simulink model "Computer"  (R2023a)
settings: Solver=VariableStepDiscrete  StartTime=0.0  StopTime=inf  RelTol=1e-3  EnableMultiTasking=on
values from neighbouring files (symbols this model uses):
  RomCode = Preprocessor(RomCode, c)    [ROM.m]
undefined symbols (not defined in the file or in its folder): c, in, RomCodeBreakpoints, RomData, RomDataBreakpoints, UartDataRx, UartDataRx_Active
libraries: Miscellaneous x281, simulink_extras x66, Memory_Blocks_Lib x46, simulink x42, Word_Multiplexers_Lib x31, Decoders_Lib x30, Encoders_Lib x10, Counters_Lib x9, Bit_Multiplexers_Lib x8, Arithmetic_Operations_Lib x5, Bit_Demultiplexers_Lib x4, Garbage x1
(part 1 of 6)
settings Model: NumberOfSteps=16  SnapshotInterval=1  PacingRate=8  Creator=Jozko Mrkvicka  LastModifiedBy=Jozko Mrkvicka
settings SolverCC: AlgebraicLoopSolver=TrustRegion
settings DataIOCC: ReturnWorkspaceOutputs=off
settings OptimizationCC: LifeSpan=inf
settings DebuggingCC: UnconnectedInputMsg=warning  UnconnectedOutputMsg=warning  UnconnectedLineMsg=warning  SFUnexpectedBacktrackingDiag=warning  SFNoUnconditionalDefaultTransitionDiag=warning  ArithmeticOperatorsInVariantConditions=warning
settings ModelReferenceCC: EnableRefExpFcnMdlSchedulingChecks=on
settings SFSimCC: SimUseLocalCustomCode=off  CustomCodeUndefinedFunction=UseInterfaceOnly
settings RTWCC: RTWUseLocalCustomCode=off
settings CodeAppCC: StateflowObjectComments=on
settings GRTTargetCC: TargetLangStandard=C89/C90 (ANSI)
settings ConfigComp: CovMetricSettings=dw  CovSaveCumulativeToWorkspaceVar=on  CovSaveSingleToWorkspaceVar=on  CovExternalEMLEnable=off
settings SimscapeCC: SimscapeNormalizeSystem=off

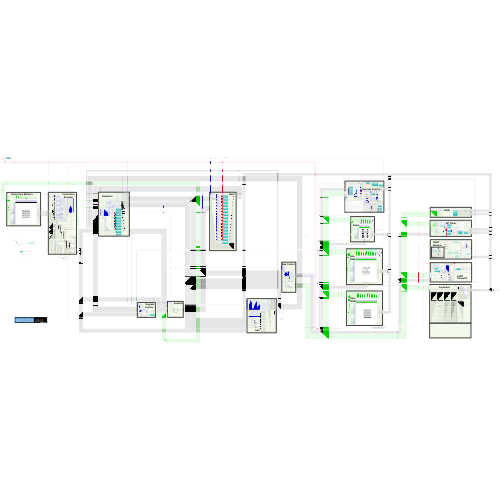
[thumbnail: Simulink's stored preview of the top-level diagram]
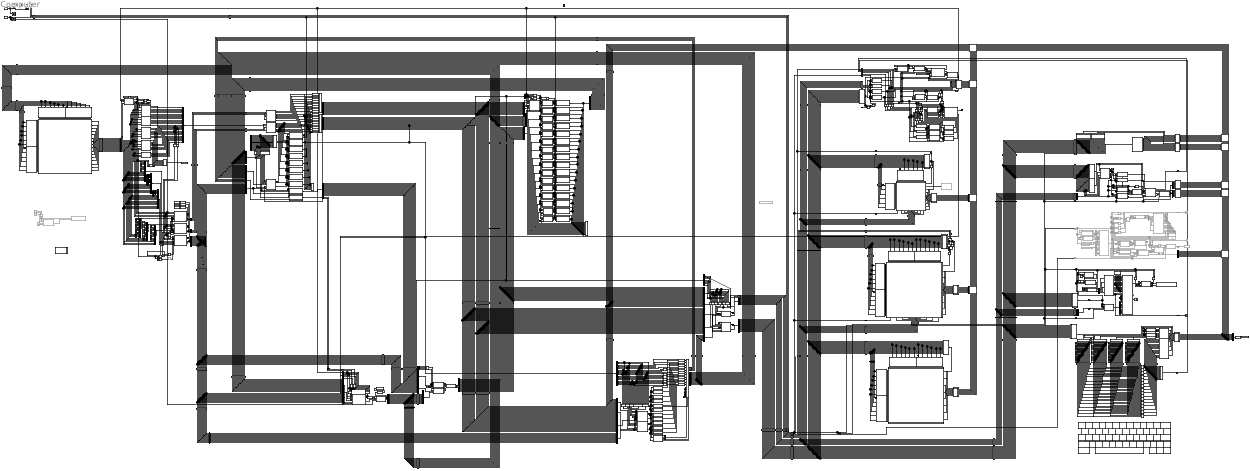
== system Computer ==
  note: TODO: Prerobit Interrupt control tak aby posielal adresu najprv dolu do zmuxovanych zbernic, a az z nich si ju bude program counter brat. Teraz je to spojene priamo.
  note: TODO: Nestacil by tu iba jeden delay blok pre celu zbernicu?
  note: TODO: Tento selector mozno nie je potrebny. Enablovat/disablovat output by sa mozno dalo pomocou signalov Enable(1b) v dekoderoch. Tam je vsak problem v tom, ze ked je enkoder disablovany, tak su vsetky jeho vystupy nulove. Potom pri konverzii nuly na index pola (uz priamo v subsysteme pamati) by mohlo dojst k problemu s matlabovskym polom. Tato poznamka plati pre vsetky vystupne selektory (Video, RAM, ROM).
  note: Note:
      | On physical layer, data read from the ferrite core memory will be immediately written back to that memory.
  note: janko halu š ka inside
  note: Interrupt Control
  note: Interrupt Control
  note: Interrupt Control
      |
      | Enabling/disabling of IRQs is controlled by IRQ Enable Register (memory mapped, read/write).
      | Each bit in the register controls specific IRQ (enable = 1, disable = 0).
      | The following interrupts are implemented in the system:
      | - (Bit 3) Keyboard IRQ
      | - (Bit 2) General Purpose Timer
      |
      | IRQs have different priorities, the higher is bit which enables an IRQ the higher priority that interrupt has.
      | Enabled IRQs are latched when they are activated by some system event (the keyboard IRQ is only exception, it is not latched at all).
      |
      | IRQ is handled in the following way:
      | - Execution of all instructions is blocked for one clock cycle.
      | - Actual Program Counter value (address of active instruction) is pushed to stack.
      | - Program Counter is loaded with an IRQ handler address of the active IRQ. The handler address is stored in the IRQ Vector Table and it can`t be reconfigured by user.
      | - Program execution jumps to the IRQ handler. Information about an IRQ handler being active is latched.
      | - When the IRQ handler is active, it can`t be interrupted by other IRQs, they are temporarily disabled, order of IRQ handling depends on their priorities).
      | - Code of the IRQ handler is executed.
      | - Once the IRQ is handled, it is deactivated. Instruction RET at the end of the handler also resets the handler latch. Now all other IRQs are re-enabled.
      | - Program execution jumps back to the address from which it was interrupted and it normally continues with next instruction.
  note: TODO: Ja si myslim ze format 0 by mal pouzivat iba unsigned immediate. Teraz pouziva signed (imm formatu 0 sa vzdy pouziva ako adresa a adresa nikdy nemoze byt zaporna).
  note: AuxALU
  note: Keyboard_IBM437
  note: Instruction Memory
  note: Video
  note: Data
      | ROM
  note: CYAN COLOR means that block contains sequential logic.
      | BLUE COLOR means that line represents control signal.
      | GREEN COLOR means that line represents address.
  note: Instruction Memory
  note: Stack
  note: Keyboard
  note: Keyboard
  note: Instruction_Decoder
  note: Instruction
      | Decoder
  note: ALU
  note: ALU
  note: Registers
  note: General_Purpose_Registers
  note: General_Purpose_Timer_16bit
  note: CMD_SET_STOP_VALUE
      | - Address 0x0000
      | - Data   <0x0000..0xFFFF>
      |
      | CMD_SET_START_VALUE
      | - Address 0x0001
      | - Data   <0x0000..0xFFFF>
      |
      | CMD_RESET
      | - Address 0x0002
      | - Data    N/A
      |
      | CMD_MODE
      | - Address 0x0003
      | - Data    0x0000 (One Shot)
      |           0x0001 (Free Run)
      |
      | CMD_RUN
      | - Address 0x0004
      | - Data    0x0000 (Halt)
      |           0x0001 (Run)
  note: 9000
  note: MRKVIČKA
  note: Stack
  note: UART
      | Transmitter
  note: UART Transmitter
  note: StartFcn*
      | disp('Starting UART...')
      | evalin('base', 'hSerialPort = serialport(in.UART_COM_PORT, in.UART_BAUD_RATE);');
      | evalin('base', 'configureCallback(hSerialPort, "byte", 1, @SerialPortCallback);');
  note: UART_Receiver
  note: This block is just a workaround (connector) between
      | the Simulink model of the UART digital hardware
      | and Windows virtual terminal. In real-world
      | implementation, this block will not be needed.
  note: StopFcn*
      | disp('Stopping UART...')
      | evalin('base', 'delete(hSerialPort);');
  note: This block is just a workaround (connector) between
      |                      the Simulink model of the UART digital hardware
      |                      and Windows virtual terminal. In real-world implementation,
      |                      this block will not be needed.
  note: UART
      | Receiver
  note: Data ROM
  note: Data
      | RAM
  note: Data RAM
  note: Video
  note: GP Timer
  note: Random_Number_Generator
  note: RNG
  note: Program Counter
  note: Program Counter
  note: Bus Control
  note: Bus Control
  "  Halt" : Constant  Value=0  OutDataTypeStr=boolean
  "  Idle" : Constant  Commented=on  OutDataTypeStr=boolean
  "  Reset" : Constant  Value=0  OutDataTypeStr=boolean
  "  Run" : Constant  OutDataTypeStr=boolean
  " Halt" : Constant  Value=0  OutDataTypeStr=boolean
   Halt{1,5..7,10} (5 alike) : Constant  Commented=on  Value=0  OutDataTypeStr=boolean
  " Halt2" : Constant  Commented=on  Value=0  OutDataTypeStr=uint16
  " Halt3" : Constant  Commented=on  Value=0  OutDataTypeStr=uint16
  " Halt4" : Constant  Value=0  OutDataTypeStr=boolean
  " Halt8" : Constant  Commented=on  Value=0  OutDataTypeStr=uint16
  " Halt9" : Constant  Value=0  OutDataTypeStr=uint16
  " Idle" : Constant  OutDataTypeStr=boolean
  " Reset" : Constant  Value=0  OutDataTypeStr=boolean
  " Run" : Constant  OutDataTypeStr=boolean
  " Run1" : Constant  Commented=on  OutDataTypeStr=boolean
  " Set" : Constant  OutDataTypeStr=boolean
  " StartBit" : Constant  Value=0  OutDataTypeStr=boolean
  " StopBit" : Constant  OutDataTypeStr=boolean
  !1 : Constant  Value=0  OutDataTypeStr=boolean
  "\"/?\"" : Constant  Value=0  OutDataTypeStr=boolean
  "\"2" : Constant  Value=0  OutDataTypeStr=boolean
  #3 : Constant  Value=0  OutDataTypeStr=boolean
  $4 : Constant  Value=0  OutDataTypeStr=boolean
  %5 : Constant  Value=0  OutDataTypeStr=boolean
  &6 : Constant  Value=0  OutDataTypeStr=boolean
  '7 : Constant  Value=0  OutDataTypeStr=boolean
  (8 : Constant  Value=0  OutDataTypeStr=boolean
  (UartRxPin) : Constant  Commented=on  Value=UartDataRx  OutDataTypeStr=uint8
  )9 : Constant  Value=0  OutDataTypeStr=boolean
  *: : Constant  Value=0  OutDataTypeStr=boolean
  +; : Constant  Value=0  OutDataTypeStr=boolean
  ,< : Constant  Value=0  OutDataTypeStr=boolean
  -= : Constant  Value=0  OutDataTypeStr=boolean
  .> : Constant  Value=0  OutDataTypeStr=boolean
  <0x0000..0x0FFF> : Subsystem
  <0x1000..0x1FFF> : Subsystem
  <0x2000..0x23FF> : Subsystem
  <0xFFF6..0xFFF6> : Subsystem
  <0xFFF7..0xFFF7> : Subsystem
  <0xFFF8..0xFFFD> : Subsystem
  <0xFFF8..0xFFFD>1 : Subsystem
  <0xFFFE..0xFFFE> : Subsystem
  <0xFFFF..0xFFFF> : Subsystem
  <0xFFFF..0xFFFF>1 : Subsystem
  @` : Constant  Value=0  OutDataTypeStr=boolean
  ADD ADDI MOVU SHIFT : Logic  Operator=OR  Inputs=13  IconShape=distinctive  AllPortsSameDT=off  OutDataTypeStr=boolean
  ADD_or_ADDI : Constant  Commented=on  Value=0  OutDataTypeStr=boolean
  Aa : Constant  Value=0  OutDataTypeStr=boolean
  Align{1,5,7..14,16..20,22..23,31,33,38,42,44..45,58..59,78..80,86..90,93,99..101} (37 alike) : Miscellaneous/Align16  SystemSampleTime=-1  VariantActivationTime=update diagram  Latency=0  AutoFrameSizeCalculation=off
  Align15 : Miscellaneous/Align6
  Align2 : Miscellaneous/Align6
  Align{21,24..30,34..37,39..41,43,81,92,95} (19 alike) : Miscellaneous/Align8  SystemSampleTime=-1  VariantActivationTime=update diagram  Latency=0  AutoFrameSizeCalculation=off
  Align{3..4,60..70,72..73,85,97..98} (18 alike) : Miscellaneous/Align12  SystemSampleTime=-1  VariantActivationTime=update diagram  Latency=0  AutoFrameSizeCalculation=off
  Align32 : Miscellaneous/Align5
  Align{46..51,54..57,82..84} (13 alike) : Miscellaneous/Align3  SystemSampleTime=-1  VariantActivationTime=update diagram  Latency=0  AutoFrameSizeCalculation=off
  Align{52..53,71,91} (4 alike) : Miscellaneous/Align2  SystemSampleTime=-1  VariantActivationTime=update diagram  Latency=0  AutoFrameSizeCalculation=off
  Align6 : Miscellaneous/Align6
  Align{74..77} (4 alike) : Miscellaneous/Align4  SystemSampleTime=-1  VariantActivationTime=update diagram  Latency=0  AutoFrameSizeCalculation=off
  Alignment{,1..8,10,13..15,17,23..26,28..30,34..36} (24 alike) : Miscellaneous/Alignment  SystemSampleTime=-1  VariantActivationTime=update diagram  Latency=0  AutoFrameSizeCalculation=off
  Alignment11 : Miscellaneous/Alignment  Commented=on  SystemSampleTime=-1  VariantActivationTime=update diagram  Latency=0  AutoFrameSizeCalculation=off
  Alignment12 : Miscellaneous/Alignment  Commented=on  SystemSampleTime=-1  VariantActivationTime=update diagram  Latency=0  AutoFrameSizeCalculation=off
  Alignment9 : Miscellaneous/Alignment  Commented=on  SystemSampleTime=-1  VariantActivationTime=update diagram  Latency=0  AutoFrameSizeCalculation=off
  AuxALU : Arithmetic_Operations_Lib/Word_Adder  SystemSampleTime=-1  VariantActivationTime=update diagram  Latency=0  AutoFrameSizeCalculation=off
      settings: LibrarySourceBlock=Arithmetic_Operations_Lib/Arithmetic_Operations_Lib/Word_Adder
  BaudRate : Scope
  Bb : Constant  Value=0  OutDataTypeStr=boolean
  Bit to Integer Converter{4..8,15} (6 alike) : simulink/Logic and Bit Operations/Bit to Integer Converter  nbits=16  bitOrder=MSB first  signedOutputValues=Unsigned  outDtype=uint16  outDtypeSigned=Inherit via internal rule
      settings: LibrarySourceBlock=|
      | commutil2/Bit to Integer
      | Converter
  Bit_Demux_{1..4} (4 alike) : Bit_Demultiplexers_Lib/Bit_Demux_2  SystemSampleTime=-1  VariantActivationTime=update diagram  Latency=0  AutoFrameSizeCalculation=off
      settings: LibrarySourceBlock=Garbage/Bit_Demux_2
  Bit_Mux_{1..4} (4 alike) : Bit_Multiplexers_Lib/Bit_Mux_2  SystemSampleTime=-1  VariantActivationTime=update diagram  Latency=0  AutoFrameSizeCalculation=off
  Bit_Mux_16 : Bit_Multiplexers_Lib/Bit_Mux_16  SystemSampleTime=-1  VariantActivationTime=update diagram  Latency=0  AutoFrameSizeCalculation=off
  Bit_Mux_16_Nand : Garbage/Bit_Mux_16_Nand  Commented=on  SystemSampleTime=-1  VariantActivationTime=update diagram  Latency=0  AutoFrameSizeCalculation=off
  Bit_Mux_2(1) : Bit_Multiplexers_Lib/Bit_Mux_2  SystemSampleTime=-1  VariantActivationTime=update diagram  Latency=0  AutoFrameSizeCalculation=off
  Bit_Mux_2(1)1 : Bit_Multiplexers_Lib/Bit_Mux_2  Commented=on  SystemSampleTime=-1  VariantActivationTime=update diagram  Latency=0  AutoFrameSizeCalculation=off
  Bit_Mux_2(1)2 : Bit_Multiplexers_Lib/Bit_Mux_2  SystemSampleTime=-1  VariantActivationTime=update diagram  Latency=0  AutoFrameSizeCalculation=off
  Block keyboard interrupt when the interrupt delay counter is running : Logic  Operator=NOT  IconShape=distinctive  AllPortsSameDT=off  OutDataTypeStr=boolean
  Bus Creator{1,4..9,11..14,21..26,29..30} (19 alike) : BusCreator  Inputs=16
  Bus Creator{2,10,20,27..28} (5 alike) : BusCreator  Inputs=8
  Bus Creator{15..18} (4 alike) : BusCreator  Inputs=12
  Bus Creator19 : BusCreator  Inputs=4
  Bus Creator3 : BusCreator  Inputs=29
  Bus Selector : BusSelector  OutputSignals=LDL,XOR,LDLI,OR,AND,ADD,ADDI,MOVU,SHIFTI,LDUI,LDU,NOT,SHIFT,MOVL,POP,MOV,SGMT,CMP,CMPI
  Bus Selector{1,9..10,13,18,26,28} (7 alike) : BusSelector  OutputSignals=b15,b14,b13,b12,b11,b10,b09,b08,b07,b06,b05,b04,b03,b02,b01,b00
  Bus Selector11 : BusSelector  OutputSignals=b11,b10,b09,b08,b07,b06,b05,b04,b03,b02,b01,b00
  Bus Selector15 : BusSelector  OutputSignals=b00
  Bus Selector16 : BusSelector  OutputSignals=b15,b14,b13,b12,b11,b10,b09,b08
  Bus Selector17 : BusSelector  OutputSignals=Equal,LessThanSigned
  Bus Selector19 : BusSelector  OutputSignals=b00,b01,b02,b03,b04,b05,b06,b07
  Bus Selector2 : BusSelector  OutputSignals=CMPI,CMP,NOT,XOR,OR,AND,ADDI,ADD,MOVU,SHIFT,SHIFTI,STUI,STU,STLI,STL,LDUI,LDU,LDLI,LDL
  Bus Selector20 : BusSelector  Commented=on  OutputSignals=b0,b1,b2,b3,b4,b5,b6,b7
  Bus Selector21 : BusSelector  Commented=on  OutputSignals=b3,b2,b1,b0
  Bus Selector22 : BusSelector  Commented=on  OutputSignals=b01,b00
  Bus Selector23 : BusSelector  OutputSignals=b03,b02,b01,b00
  Bus Selector24 : BusSelector  Commented=on  OutputSignals=b3,b2,b1,b0
  Bus Selector25 : BusSelector  OutputSignals=b07,b06,b05,b04,b03,b02,b01,b00
  Bus Selector27 : BusSelector  OutputSignals=b11,b10,b09,b08,b07,b06,b05,b04,b03,b02,b01,b00
  Bus Selector29 : BusSelector  OutputSignals=b02,b01,b00
  Bus Selector3 : BusSelector  OutputSignals=RET,STUI,STLI,STU,STL,LDUI,LDLI,LDU,LDL
  Bus Selector30 : BusSelector  OutputSignals=b02,b01,b00
  Bus Selector4 : BusSelector  OutputSignals=b07,b06,b05,b04,b03,b02,b01,b00
  Bus Selector5 : BusSelector  OutputSignals=PUSH,CALL,POP,RET
  Bus Selector6 : BusSelector  OutputSignals=b00,b01,b02,b03,b04,b05,b06,b07
  Bus Selector7 : BusSelector  OutputSignals=RET,JMP,CALL,JPE,JLT
  Bus Selector8 : BusSelector  OutputSignals=STUI,STLI,LDUI,LDLI,CALL
  CLK{,3..7} (6 alike) : Miscellaneous/Alignment  SystemSampleTime=-1  VariantActivationTime=update diagram  Latency=0  AutoFrameSizeCalculation=off
  CLK1 : Miscellaneous/Alignment  Commented=on  SystemSampleTime=-1  VariantActivationTime=update diagram  Latency=0  AutoFrameSizeCalculation=off
  CLK2 : Miscellaneous/Alignment  Commented=on  SystemSampleTime=-1  VariantActivationTime=update diagram  Latency=0  AutoFrameSizeCalculation=off
  CMP_or_CMPI : Constant  Commented=on  Value=0  OutDataTypeStr=boolean
  CPU : Scope
  Cc : Constant  Value=0  OutDataTypeStr=boolean
  Clear_RxBufferReady : Constant  Commented=on  OutDataTypeStr=boolean
  Clock : simulink_extras/Flip Flops/Clock  period=16
  Constant{1..2,5,9,11..13,15..16,18,26..44,46..59,61..66,69,72,75,87..90} (56 alike) : Constant  Value=0  OutDataTypeStr=boolean
  Constant{3,6..7,10,19,60,77} (7 alike) : Constant  Value=0  OutDataTypeStr=Bus: BUS_UINT16_T
  Constant45 : Constant  Commented=on  Value=10  OutDataTypeStr=uint8
  Constant67 : Constant  Value=in.IRQ_ADDR_KEYBOARD  OutDataTypeStr=uint16
  Constant68 : Constant  Value=in.IRQ_ADDR_UART  OutDataTypeStr=uint16
  Constant70 : Constant
  Constant71 : Constant  Value=in.IRQ_ADDR_TIMER  OutDataTypeStr=uint16
  Constant73 : Constant  Value=0
  Constant74 : Constant  Value=in.IRQ_ADDR_FPU  OutDataTypeStr=uint16
  Constant76 : Constant  Value=in.IRQ_Keyboard_Test  OutDataTypeStr=uint16
  Constant83 : Constant  Value=15  OutDataTypeStr=uint8
  Constant91 : Constant  Commented=on  Value=0  OutDataTypeStr=boolean
  Constant92 : Constant  Value=10  OutDataTypeStr=uint8
  Constant93 : Constant  Commented=on  Value=UartDataRx_Active  OutDataTypeStr=boolean
  Constant94 : Constant  Commented=on  Value=10  OutDataTypeStr=uint8
  Constant95 : Constant  OutDataTypeStr=boolean
  Constant96 : Constant  OutDataTypeStr=boolean
  Counter_16bit : Counters_Lib/Counter_16bit  SystemSampleTime=-1  VariantActivationTime=update diagram  Latency=0  AutoFrameSizeCalculation=off
  Counter_16bit(1) : Counters_Lib/Counter_16bit  SystemSampleTime=-1  VariantActivationTime=update diagram  Latency=0  AutoFrameSizeCalculation=off
  Counter_Control : Counters_Lib/Counter_Control  SystemSampleTime=-1  VariantActivationTime=update diagram  Latency=0  AutoFrameSizeCalculation=off
  Counter_Control(1) : Counters_Lib/Counter_Control  SystemSampleTime=-1  VariantActivationTime=update diagram  Latency=0  AutoFrameSizeCalculation=off
  CrRet undef : Constant  Value=0  OutDataTypeStr=boolean
  Ctrl01 : Constant  Value=0  OutDataTypeStr=boolean
  Ctrl02 : Constant  Value=0  OutDataTypeStr=boolean
  Ctrl03 : Constant  Value=0  OutDataTypeStr=boolean
  Ctrl04 : Constant  Value=0  OutDataTypeStr=boolean
  Ctrl05 : Constant  Value=0  OutDataTypeStr=boolean
  Ctrl06 : Constant  Value=0  OutDataTypeStr=boolean
  Ctrl07 : Constant  Value=0  OutDataTypeStr=boolean
  Ctrl12 : Constant  Value=0  OutDataTypeStr=boolean
  Ctrl14 : Constant  Value=0  OutDataTypeStr=boolean
  Ctrl15 : Constant  Value=0  OutDataTypeStr=boolean
  DataBitDetected (GoToNextState) : Logic  Commented=on  IconShape=distinctive  AllPortsSameDT=off  OutDataTypeStr=boolean
  Data_RAM (0x000 .. 0xFFF) : Subsystem
      settings: PortSchema="{\"entries\":[{\"content\":{\"sides\":[{\"content\":{\"connectorIds\":[\"In1\",\"In2\",\"In3\",\"In4\",\"In5\",\"In6\",\"In7\",\"In8\",\"In9\",\"In10\",\"In11\",\"In12\",\"In13\",\"In14\",\"In15\",\"In16\",\"In17\",\"In18\",\"In19\",\"In20\",\"In21\",\"In22\",\"In23\",\"In24\",\"In25\",\"In26\",\"In27\",\"In28\",\"In29\",\"In30\",\"In31\",\"In32\",\"In33\",\"In34\",\"In35\",\"In36\",\"In37\",\"In38\",\"In39\",\"In40\",\"In41\",\"In42\",\"In43\",\"In44\",\"In45\",\"In46\",\"In47\",\"In48\",\"In49\",\"In50\",\"In51\",\"In52\",\"In53\",\"In54\",\"In55\",\"In56\",\"In57\",\"In58\",\"In59\",\"In60\",\"In61\",\"In62\",\"In63\",\"In64\"]},\"type\":\"ConnectorPlacement.EquallySpacedRectSide\",\"uuid\":\"1db07b03-14d7-4059-8e9e-27241d1b2c6f\"},{\"content\":{\"connectorIds\":[\"In138\",\"Out1\",\"Out2\",\"Out3\",\"Out4\",\"Out5\",\"Out6\",\"Out7\",\"Out8\"],\"side\":\"RIGHT\"},\"type\":\"ConnectorPlacement.EquallySpacedRectSide\",\"uuid\":\"da5110d5-f105-41ed-a5ea-e540a7740f0d\"},{\"content\":{\"connectorIds\":[\"In65\",\"In66\",\"In67\",\"In68\",\"In69\",\"In70\",\"In71\",\"In72\",\"In73\",\"In74\",\"In75\",\"In76\",\"In77\",\"In78\",\"In79\",\"In80\",\"In81\",\"In82\",\"In83\",\"In84\",\"In85\",\"In86\",\"In87\",\"In88\",\"In89\",\"In90\",\"In91\",\"In92\",\"In93\",\"In94\",\"In95\",\"In96\",\"In97\",\"In98\",\"In99\",\"In100\",\"In101\",\"In102\",\"In103\",\"In104\",\"In105\",\"In106\",\"In107\",\"In108\",\"In109\",\"In110\",\"In111\",\"In112\",\"In113\",\"In114\",\"In115\",\"In116\",\"In117\",\"In118\",\"In119\",\"In120\",\"In121\",\"In122\",\"In123\",\"In124\",\"In125\",\"In126\",\"In127\",\"In128\"],\"side\":\"TOP\"},\"type\":\"ConnectorPlacement.EquallySpacedRectSide\",\"uuid\":\"ecc4e51e-7cb2-40ca-97e4-7326426aa5e7\"},{\"content\":{\"connectorIds\":[\"In129\",\"In130\",\"In131\",\"In132\",\"In133\",\"In134\",\"In135\",\"In136\",\"In137\"],\"side\":\"BOTTOM\"},\"type\":\"ConnectorPlacement.EquallySpacedRectSide\",\"uuid\":\"3d59fc9c-ab69-48a8-998e-8118c8f06a1a\"}]},\"type\":\"ConnectorPlacement.EquallySpacedConnector\",\"uuid\":\"5e28cbe1-b8ac-4836-91bf-5b5dc95013cb\"}],\"packageUris\":[\"http://schema.mathworks.com/mf0/Connector/R2020b\"],\"version\":\"1.0\"}"
  Data_ROM (0x000 .. 0xFFF) : Subsystem
      settings: PortSchema="{\"entries\":[{\"content\":{\"sides\":[{\"content\":{\"connectorIds\":[\"In1\",\"In2\",\"In3\",\"In4\",\"In5\",\"In6\",\"In7\",\"In8\",\"In9\",\"In10\",\"In11\",\"In12\",\"In13\",\"In14\",\"In15\",\"In16\",\"In17\",\"In18\",\"In19\",\"In20\",\"In21\",\"In22\",\"In23\",\"In24\",\"In25\",\"In26\",\"In27\",\"In28\",\"In29\",\"In30\",\"In31\",\"In32\",\"In33\",\"In34\",\"In35\",\"In36\",\"In37\",\"In38\",\"In39\",\"In40\",\"In41\",\"In42\",\"In43\",\"In44\",\"In45\",\"In46\",\"In47\",\"In48\",\"In49\",\"In50\",\"In51\",\"In52\",\"In53\",\"In54\",\"In55\",\"In56\",\"In57\",\"In58\",\"In59\",\"In60\",\"In61\",\"In62\",\"In63\",\"In64\"]},\"type\":\"ConnectorPlacement.EquallySpacedRectSide\",\"uuid\":\"1db07b03-14d7-4059-8e9e-27241d1b2c6f\"},{\"content\":{\"connectorIds\":[\"Out1\",\"Out2\",\"Out3\",\"Out4\",\"Out5\",\"Out6\",\"Out7\",\"Out8\"],\"side\":\"RIGHT\"},\"type\":\"ConnectorPlacement.EquallySpacedRectSide\",\"uuid\":\"da5110d5-f105-41ed-a5ea-e540a7740f0d\"},{\"content\":{\"connectorIds\":[\"In65\",\"In66\",\"In67\",\"In68\",\"In69\",\"In70\",\"In71\",\"In72\",\"In73\",\"In74\",\"In75\",\"In76\",\"In77\",\"In78\",\"In79\",\"In80\",\"In81\",\"In82\",\"In83\",\"In84\",\"In85\",\"In86\",\"In87\",\"In88\",\"In89\",\"In90\",\"In91\",\"In92\",\"In93\",\"In94\",\"In95\",\"In96\",\"In97\",\"In98\",\"In99\",\"In100\",\"In101\",\"In102\",\"In103\",\"In104\",\"In105\",\"In106\",\"In107\",\"In108\",\"In109\",\"In110\",\"In111\",\"In112\",\"In113\",\"In114\",\"In115\",\"In116\",\"In117\",\"In118\",\"In119\",\"In120\",\"In121\",\"In122\",\"In123\",\"In124\",\"In125\",\"In126\",\"In127\",\"In128\"],\"side\":\"TOP\"},\"type\":\"ConnectorPlacement.EquallySpacedRectSide\",\"uuid\":\"ecc4e51e-7cb2-40ca-97e4-7326426aa5e7\"}]},\"type\":\"ConnectorPlacement.EquallySpacedConnector\",\"uuid\":\"5e28cbe1-b8ac-4836-91bf-5b5dc95013cb\"}],\"packageUris\":[\"http://schema.mathworks.com/mf0/Connector/R2020b\"],\"version\":\"1.0\"}"
  Dd : Constant  Value=0  OutDataTypeStr=boolean
  Dec_1 : Decoders_Lib/Dec_8  SystemSampleTime=-1  VariantActivationTime=update diagram  Latency=0  AutoFrameSizeCalculation=off
  Dec_16 : Decoders_Lib/Dec_16  SystemSampleTime=-1  VariantActivationTime=update diagram  Latency=0  AutoFrameSizeCalculation=off
  Dec_32_Enbl{1,4..7,9,11..18} (14 alike) : Decoders_Lib/Dec_32_Enbl  SystemSampleTime=-1  VariantActivationTime=update diagram  Latency=0  AutoFrameSizeCalculation=off
  Dec_4_Enbl : Decoders_Lib/Dec_4_Enbl  SystemSampleTime=-1  VariantActivationTime=update diagram  Latency=0  AutoFrameSizeCalculation=off
  Dec_8 : Decoders_Lib/Dec_8  SystemSampleTime=-1  VariantActivationTime=update diagram  Latency=0  AutoFrameSizeCalculation=off
  Dec_8_Enbl : Decoders_Lib/Dec_8_Enbl  SystemSampleTime=-1  VariantActivationTime=update diagram  Latency=0  AutoFrameSizeCalculation=off
  Delay : Constant  Value=in.IRQ_KEYBOARD_DELAY  OutDataTypeStr=uint16
  Delay_8b : Miscellaneous/Delay_8b  SystemSampleTime=-1  VariantActivationTime=update diagram  Latency=0  AutoFrameSizeCalculation=off
  Delay_8b1 : Miscellaneous/Delay_8b  SystemSampleTime=-1  VariantActivationTime=update diagram  Latency=0  AutoFrameSizeCalculation=off
  Ee : Constant  Value=0  OutDataTypeStr=boolean
  Enable_IRQ_FPU : Memory_Blocks_Lib/Bit_DataEnbl  SystemSampleTime=-1  VariantActivationTime=update diagram  Latency=0  AutoFrameSizeCalculation=off
  Enable_IRQ_Keyboard : Memory_Blocks_Lib/Bit_DataEnbl  SystemSampleTime=-1  VariantActivationTime=update diagram  Latency=0  AutoFrameSizeCalculation=off
  Enable_IRQ_Timer : Memory_Blocks_Lib/Bit_DataEnbl  SystemSampleTime=-1  VariantActivationTime=update diagram  Latency=0  AutoFrameSizeCalculation=off
  Enable_IRQ_UART : Memory_Blocks_Lib/Bit_DataEnbl  SystemSampleTime=-1  VariantActivationTime=update diagram  Latency=0  AutoFrameSizeCalculation=off
  Enc_16 : Encoders_Lib/Enc_16  SystemSampleTime=-1  VariantActivationTime=update diagram  Latency=0  AutoFrameSizeCalculation=off
  Enc_2 : Encoders_Lib/Enc_8  SystemSampleTime=-1  VariantActivationTime=update diagram  Latency=0  AutoFrameSizeCalculation=off
  Entering_IRQ_Handler... (1 clock cycle) : Logic  Operator=NOT  IconShape=distinctive  AllPortsSameDT=off  OutDataTypeStr=boolean
  ErrorStopBitNotDetected : Terminator  Commented=on
  "Exiting_IRQ_Handler... (1 clock cycle) " : Logic  IconShape=distinctive  AllPortsSameDT=off  OutDataTypeStr=boolean
  Ff : Constant  Value=0  OutDataTypeStr=boolean
  "For simulation, use only data bits. Real-world implementation will use whole frame." : Logic  Operator=OR  Inputs=8  IconShape=distinctive  AllPortsSameDT=off  OutDataTypeStr=boolean
  Format 0: FF|OO|CCCC   CCCCCCCC : Decoders_Lib/Dec_4_Enbl  SystemSampleTime=-1  VariantActivationTime=update diagram  Latency=0  AutoFrameSizeCalculation=off
  Format 1: FF|OOO|SSS   CCCCCCCC : Decoders_Lib/Dec_8_Enbl  SystemSampleTime=-1  VariantActivationTime=update diagram  Latency=0  AutoFrameSizeCalculation=off
  Format 2: FF|OOO|DDD   CCCCCCCC : Decoders_Lib/Dec_8_Enbl  SystemSampleTime=-1  VariantActivationTime=update diagram  Latency=0  AutoFrameSizeCalculation=off
  Format 3: FF|OOOOO|R   R|DDD|R|SSS : Decoders_Lib/Dec_8_Enbl  SystemSampleTime=-1  VariantActivationTime=update diagram  Latency=0  AutoFrameSizeCalculation=off
  Format 3: FF|OOOOO|R   R|DDD|R|SSS2 : Decoders_Lib/Dec_8_Enbl  SystemSampleTime=-1  VariantActivationTime=update diagram  Latency=0  AutoFrameSizeCalculation=off
  Format_1_Signed : Logic  IconShape=distinctive  AllPortsSameDT=off  OutDataTypeStr=boolean
  Format_1_Unsigned : Logic  IconShape=distinctive  AllPortsSameDT=off  OutDataTypeStr=boolean
  Format_2_Signed : Logic  IconShape=distinctive  AllPortsSameDT=off  OutDataTypeStr=boolean
  Format_2_Unsigned : Logic  IconShape=distinctive  AllPortsSameDT=off  OutDataTypeStr=boolean
  FreqDivider : Counters_Lib/Counter_4bit_Cfg  SystemSampleTime=-1  VariantActivationTime=update diagram  Latency=0  AutoFrameSizeCalculation=off
  FromImmediate : Constant  Commented=on  Value=0  OutDataTypeStr=boolean
  General_Purpose_Register_{0..7} (8 alike) : Memory_Blocks_Lib/Word  SystemSampleTime=-1  VariantActivationTime=update diagram  Latency=0  AutoFrameSizeCalculation=off
      settings: LibrarySourceBlock=Memory_Blocks_Lib/Memory_Blocks_Lib/Word
  Gg : Constant  Value=0  OutDataTypeStr=boolean
  GreaterThan(1b) : Terminator
  GreaterThan(1b)1 : Terminator
  GreaterThan(1b)2 : Terminator
  Hh : Constant  Value=0  OutDataTypeStr=boolean
  IRQ_Active : Logic  Operator=NOT  IconShape=distinctive  AllPortsSameDT=off  OutDataTypeStr=boolean
  IRQ_FPU : Constant  Value=0  OutDataTypeStr=boolean
  IRQ_FPU_Latch : Memory_Blocks_Lib/Bit_DataEnbl  SystemSampleTime=-1  VariantActivationTime=update diagram  Latency=0  AutoFrameSizeCalculation=off
  IRQ_Handler_Active : Memory_Blocks_Lib/Bit_DataEnbl  SystemSampleTime=-1  VariantActivationTime=update diagram  Latency=0  AutoFrameSizeCalculation=off
  IRQ_Timer_Latch : Memory_Blocks_Lib/Bit_DataEnbl  SystemSampleTime=-1  VariantActivationTime=update diagram  Latency=0  AutoFrameSizeCalculation=off
  IRQ_UART : Constant  Value=0  OutDataTypeStr=boolean
  IRQ_UART_Latch : Memory_Blocks_Lib/Bit_DataEnbl  SystemSampleTime=-1  VariantActivationTime=update diagram  Latency=0  AutoFrameSizeCalculation=off
  IRQ_UART_RX (toStatusRegister...) : Display  Commented=on
  If IRQ is enabled then disable all instructions for one clock cycle to allow program counter to jump to a IRQ handler. : Logic  Operator=NOT  IconShape=distinctive  AllPortsSameDT=off  OutDataTypeStr=boolean
  Ii : Constant  Value=0  OutDataTypeStr=boolean
  Immediate_Signed : Logic  Commented=on  Operator=OR  IconShape=distinctive  AllPortsSameDT=off  OutDataTypeStr=boolean
  Immediate_Unsigned : Logic  Operator=OR  IconShape=distinctive  AllPortsSameDT=off  OutDataTypeStr=boolean
  Instruction_ADD : Arithmetic_Operations_Lib/Word_Adder  SystemSampleTime=-1  VariantActivationTime=update diagram  Latency=0  AutoFrameSizeCalculation=off
      settings: LibrarySourceBlock=Arithmetic_Operations_Lib/Arithmetic_Operations_Lib/Word_Adder
  Instruction_AND : Subsystem
  Instruction_CMP : Arithmetic_Operations_Lib/Word_Comparator  SystemSampleTime=-1  VariantActivationTime=update diagram  Latency=0  AutoFrameSizeCalculation=off
      settings: LibrarySourceBlock=Arithmetic_Operations_Lib/Arithmetic_Operations_Lib/Word_Comparator
  Instruction_LDL : Subsystem
  Instruction_LDU : Subsystem
  Instruction_MOVU : Subsystem
  Instruction_NOT : Arithmetic_Operations_Lib/Word_Not  SystemSampleTime=-1  VariantActivationTime=update diagram  Latency=0  AutoFrameSizeCalculation=off
      settings: LibrarySourceBlock=Arithmetic_Operations_Lib/Arithmetic_Operations_Lib/Bitwise_NOT
  Instruction_OR : Subsystem
  Instruction_ROM (0x000 .. 0xFFF) : Subsystem
      settings: PortSchema="{\"entries\":[{\"content\":{\"sides\":[{\"content\":{\"connectorIds\":[\"In1\",\"In2\",\"In3\",\"In4\",\"In5\",\"In6\",\"In7\",\"In8\",\"In9\",\"In10\",\"In11\",\"In12\",\"In13\",\"In14\",\"In15\",\"In16\",\"In17\",\"In18\",\"In19\",\"In20\",\"In21\",\"In22\",\"In23\",\"In24\",\"In25\",\"In26\",\"In27\",\"In28\",\"In29\",\"In30\",\"In31\",\"In32\",\"In33\",\"In34\",\"In35\",\"In36\",\"In37\",\"In38\",\"In39\",\"In40\",\"In41\",\"In42\",\"In43\",\"In44\",\"In45\",\"In46\",\"In47\",\"In48\",\"In49\",\"In50\",\"In51\",\"In52\",\"In53\",\"In54\",\"In55\",\"In56\",\"In57\",\"In58\",\"In59\",\"In60\",\"In61\",\"In62\",\"In63\",\"In64\"]},\"type\":\"ConnectorPlacement.EquallySpacedRectSide\",\"uuid\":\"1db07b03-14d7-4059-8e9e-27241d1b2c6f\"},{\"content\":{\"connectorIds\":[\"Out1\",\"Out2\",\"Out3\",\"Out4\",\"Out5\",\"Out6\",\"Out7\",\"Out8\",\"Out9\",\"Out10\",\"Out11\",\"Out12\",\"Out13\",\"Out14\",\"Out15\",\"Out16\"],\"side\":\"RIGHT\"},\"type\":\"ConnectorPlacement.EquallySpacedRectSide\",\"uuid\":\"da5110d5-f105-41ed-a5ea-e540a7740f0d\"},{\"content\":{\"connectorIds\":[\"In65\",\"In66\",\"In67\",\"In68\",\"In69\",\"In70\",\"In71\",\"In72\",\"In73\",\"In74\",\"In75\",\"In76\",\"In77\",\"In78\",\"In79\",\"In80\",\"In81\",\"In82\",\"In83\",\"In84\",\"In85\",\"In86\",\"In87\",\"In88\",\"In89\",\"In90\",\"In91\",\"In92\",\"In93\",\"In94\",\"In95\",\"In96\",\"In97\",\"In98\",\"In99\",\"In100\",\"In101\",\"In102\",\"In103\",\"In104\",\"In105\",\"In106\",\"In107\",\"In108\",\"In109\",\"In110\",\"In111\",\"In112\",\"In113\",\"In114\",\"In115\",\"In116\",\"In117\",\"In118\",\"In119\",\"In120\",\"In121\",\"In122\",\"In123\",\"In124\",\"In125\",\"In126\",\"In127\",\"In128\"],\"side\":\"TOP\"},\"type\":\"ConnectorPlacement.EquallySpacedRectSide\",\"uuid\":\"ecc4e51e-7cb2-40ca-97e4-7326426aa5e7\"}]},\"type\":\"ConnectorPlacement.EquallySpacedConnector\",\"uuid\":\"5e28cbe1-b8ac-4836-91bf-5b5dc95013cb\"}],\"packageUris\":[\"http://schema.mathworks.com/mf0/Connector/R2020b\"],\"version\":\"1.0\"}"
  Instruction_SHIFT : Subsystem
  Instruction_STL : Subsystem
  Instruction_STU : Subsystem
  Instruction_XOR : Arithmetic_Operations_Lib/Word_Xor  SystemSampleTime=-1  VariantActivationTime=update diagram  Latency=0  AutoFrameSizeCalculation=off
  IsAnyKeyPressed? : Logic  Operator=OR  Inputs=16  IconShape=distinctive  AllPortsSameDT=off  OutDataTypeStr=boolean
  Jj : Constant  Value=0  OutDataTypeStr=boolean
  Kk : Constant  Value=0  OutDataTypeStr=boolean
  Linear_Feedback_Shift_Register_15bit (random number generator) : Subsystem
  Ll : Constant  Value=0  OutDataTypeStr=boolean
  LnFeed Right : Constant  Value=0  OutDataTypeStr=boolean
  Logical Operator{1,27,31..32,35,71,75..76,78} (9 alike) : Logic  Operator=NOT  IconShape=distinctive  AllPortsSameDT=off  OutDataTypeStr=boolean
  Logical Operator10 : Logic  Operator=OR  Inputs=16  IconShape=distinctive  AllPortsSameDT=off  OutDataTypeStr=boolean
  Logical Operator{3,11,13,15..17,23,38,62} (9 alike) : Logic  Operator=OR  Inputs=4  IconShape=distinctive  AllPortsSameDT=off  OutDataTypeStr=boolean
  Logical Operator12 : Logic  Operator=OR  Inputs=6  IconShape=distinctive  AllPortsSameDT=off  OutDataTypeStr=boolean
  Logical Operator{9,14,24,26,29,39..42,49..51,54,69..70} (15 alike) : Logic  IconShape=distinctive  AllPortsSameDT=off  OutDataTypeStr=boolean
  Logical Operator18 : Logic  Operator=OR  Inputs=6  IconShape=distinctive  AllPortsSameDT=off  OutDataTypeStr=boolean
  Logical Operator19 : Logic  Operator=OR  Inputs=7  IconShape=distinctive  AllPortsSameDT=off  OutDataTypeStr=boolean
  Logical Operator{2,4..6,8,20,22,25,28,30,34,37,44..45,47,52..53,57,61,68} (20 alike) : Logic  Operator=OR  IconShape=distinctive  AllPortsSameDT=off  OutDataTypeStr=boolean
  Logical Operator21 : Logic  Operator=OR  Inputs=3  IconShape=distinctive  AllPortsSameDT=off  OutDataTypeStr=boolean
  Logical Operator36 : Logic  Operator=OR  Inputs=3  IconShape=distinctive  AllPortsSameDT=off  OutDataTypeStr=boolean
  Logical Operator43 : Logic  Commented=on  Operator=OR  Inputs=16  IconShape=distinctive  OutDataTypeStr=boolean
  Logical Operator46 : Logic  Operator=NOT  Inputs=4  IconShape=distinctive  AllPortsSameDT=off  OutDataTypeStr=boolean
  Logical Operator48 : Logic  Inputs=3  IconShape=distinctive  AllPortsSameDT=off  OutDataTypeStr=boolean
  Logical Operator55 : Logic  Operator=NAND  IconShape=distinctive  AllPortsSameDT=off  OutDataTypeStr=boolean
  Logical Operator56 : Logic  Operator=NAND  IconShape=distinctive  AllPortsSameDT=off  OutDataTypeStr=boolean
  Logical Operator58 : Logic  Operator=NAND  IconShape=distinctive  AllPortsSameDT=off  OutDataTypeStr=boolean
  Logical Operator59 : Logic  Commented=on  Operator=OR  Inputs=8  IconShape=distinctive  AllPortsSameDT=off  OutDataTypeStr=boolean
  Logical Operator60 : Logic  Commented=on  IconShape=distinctive  AllPortsSameDT=off  OutDataTypeStr=boolean
  Logical Operator63 : Logic  Commented=on  Operator=OR  Inputs=4  IconShape=distinctive  AllPortsSameDT=off  OutDataTypeStr=boolean
  Logical Operator64 : Logic  Commented=on  Operator=OR  IconShape=distinctive  AllPortsSameDT=off  OutDataTypeStr=boolean
  Logical Operator65 : Logic  Commented=on  IconShape=distinctive  AllPortsSameDT=off  OutDataTypeStr=boolean
  Logical Operator66 : Logic  Commented=on  Operator=NOT  IconShape=distinctive  AllPortsSameDT=off  OutDataTypeStr=boolean
  Logical Operator67 : Logic  Commented=on  Operator=OR  IconShape=distinctive  AllPortsSameDT=off  OutDataTypeStr=boolean
  Logical Operator7 : Logic  Operator=OR  Inputs=12  IconShape=distinctive  AllPortsSameDT=off  OutDataTypeStr=boolean
  Logical Operator72 : Logic  Commented=on  Operator=NOT  IconShape=distinctive  AllPortsSameDT=off  OutDataTypeStr=boolean
  Logical Operator73 : Logic  Commented=on  Operator=OR  IconShape=distinctive  AllPortsSameDT=off  OutDataTypeStr=boolean
  Logical Operator74 : Logic  Commented=on  Operator=OR  Inputs=3  IconShape=distinctive  AllPortsSameDT=off  OutDataTypeStr=boolean
  MATLAB Function : MATLAB Function  StartFcn=|  StopFcn=|  TreatAsAtomicUnit=on  SystemSampleTime=1
      StartFcn=|
      | %disp('Starting UART...')
      | evalin('base', 'hSerialPort = serialport(in.UART_COM_PORT, in.UART_BAUD_RATE);');
      | evalin('base', 'configureCallback(hSerialPort, "byte", 1, @SerialPortCallback);');
      StopFcn=|
      | %disp('Stopping UART...')
      | evalin('base', 'delete(hSerialPort);');
  MATLAB Function1 : MATLAB Function  Commented=on  TreatAsAtomicUnit=on
  Majority_Selector (2_out_of_3) : Subsystem  Commented=on
  Memory2 : Memory  Commented=on
  Merge16_Simulated : Miscellaneous/Merge16_Simulated
      settings: LibrarySourceBlock=Memory_Blocks_Lib/Memory_Blocks_Lib/4096x1B_RAM_Simulated
  Merge2_8b_Simulated{1..9} (9 alike) : Miscellaneous/Merge2_8b_Simulated  SystemSampleTime=-1  VariantActivationTime=update diagram  Latency=0  AutoFrameSizeCalculation=off
      settings: PortSchema="{\"entries\":[{\"content\":{\"sides\":[{\"content\":{\"connectorIds\":[\"In1\",\"In2\",\"In3\",\"In4\",\"In5\",\"In6\",\"In7\",\"In8\"]},\"type\":\"ConnectorPlacement.EquallySpacedRectSide\",\"uuid\":\"74758995-5ec8-49f8-a534-c3a678c5c312\"},{\"content\":{\"side\":\"RIGHT\"},\"type\":\"ConnectorPlacement.EquallySpacedRectSide\",\"uuid\":\"c467dbeb-9f00-48b9-a78d-a08162163a10\"},{\"content\":{\"connectorIds\":[\"Out1\",\"Out2\",\"Out3\",\"Out4\",\"Out5\",\"Out6\",\"Out7\",\"Out8\"],\"side\":\"TOP\"},\"type\":\"ConnectorPlacement.EquallySpacedRectSide\",\"uuid\":\"39dea3b5-6733-4ade-ab22-e62d310be187\"},{\"content\":{\"connectorIds\":[\"In9\",\"In10\",\"In11\",\"In12\",\"In13\",\"In14\",\"In15\",\"In16\"],\"side\":\"BOTTOM\"},\"type\":\"ConnectorPlacement.EquallySpacedRectSide\",\"uuid\":\"73149fc1-24d9-4bdc-92e2-12fb1d742836\"}]},\"type\":\"ConnectorPlacement.EquallySpacedConnector\",\"uuid\":\"fd2226dc-a4d3-43ad-9cda-54babd09ac78\"}],\"packageUris\":[\"http://schema.mathworks.com/mf0/Connector/R2020b\"],\"version\":\"1.0\"}"
  Merge8_Simulated : Miscellaneous/Merge8_Simulated
      settings: LibrarySourceBlock=Memory_Blocks_Lib/Memory_Blocks_Lib/4096x1B_RAM_Simulated
  Merge8_Simulated1 : Miscellaneous/Merge8_Simulated
      settings: LibrarySourceBlock=Memory_Blocks_Lib/Memory_Blocks_Lib/4096x1B_RAM_Simulated
  Mm : Constant  Value=0  OutDataTypeStr=boolean
  Mode : Memory_Blocks_Lib/Bit_DataEnbl  SystemSampleTime=-1  VariantActivationTime=update diagram  Latency=0  AutoFrameSizeCalculation=off
  Mux1 : Mux  Inputs=8
  Mux_1 : Word_Multiplexers_Lib/Word_Mux_4  SystemSampleTime=-1  VariantActivationTime=update diagram  Latency=0  AutoFrameSizeCalculation=off
  Mux_4 : Word_Multiplexers_Lib/Word_Mux_4  SystemSampleTime=-1  VariantActivationTime=update diagram  Latency=0  AutoFrameSizeCalculation=off
  NULL NULL : Constant  Value=0  OutDataTypeStr=boolean
  Name{1,5..6,8,11,16..17,19..29} (18 alike) : Miscellaneous/Name
  Nn : Constant  Value=0  OutDataTypeStr=boolean
  NotUsed0 : Constant  Commented=on  Value=0  OutDataTypeStr=boolean
  NotUsed1 : Constant  Value=0  OutDataTypeStr=boolean
  OneShot : Constant  Value=0  OutDataTypeStr=boolean
  Oo : Constant  Value=0  OutDataTypeStr=boolean
  Or{17..19,21} (4 alike) : Logic  Operator=OR  Inputs=16  IconShape=distinctive  AllPortsSameDT=off  OutDataTypeStr=boolean
  Or{20,22..36} (16 alike) : Logic  Operator=OR  Inputs=4  IconShape=distinctive  AllPortsSameDT=off  OutDataTypeStr=boolean
  Pp : Constant  Value=0  OutDataTypeStr=boolean
  Priority_Selector : Decoders_Lib/Priority_Selector_4  SystemSampleTime=-1  VariantActivationTime=update diagram  Latency=0  AutoFrameSizeCalculation=off
      settings: LibrarySourceBlock=Decoders_Lib/Priority_Selector
  Priority_Selector_1 : Decoders_Lib/Priority_Selector_2  SystemSampleTime=-1  VariantActivationTime=update diagram  Latency=0  AutoFrameSizeCalculation=off
  Priority_Selector_2 : Decoders_Lib/Priority_Selector_2  SystemSampleTime=-1  VariantActivationTime=update diagram  Latency=0  AutoFrameSizeCalculation=off
  Priority_Selector_3 : Decoders_Lib/Priority_Selector_2  SystemSampleTime=-1  VariantActivationTime=update diagram  Latency=0  AutoFrameSizeCalculation=off
  Program_Counter : Counters_Lib/Counter_16bit  SystemSampleTime=-1  VariantActivationTime=update diagram  Latency=0  AutoFrameSizeCalculation=off
  Push Button1 : PushButtonBlock  ButtonText=!1
  Push Button10 : PushButtonBlock  ButtonText=0
  Push Button12 : PushButtonBlock  ButtonText=G
  Push Button13 : PushButtonBlock  ButtonText=H
  Push Button14 : PushButtonBlock  ButtonText=J
  Push Button15 : PushButtonBlock  ButtonText=K
  Push Button16 : PushButtonBlock  ButtonText=L
  Push Button17 : PushButtonBlock  ButtonText=Z
  Push Button18 : PushButtonBlock  ButtonText=X
  Push Button19 : PushButtonBlock  ButtonText=C
  Push Button2 : PushButtonBlock  ButtonText=.>
  Push Button20 : PushButtonBlock  ButtonText=Q
  Push Button21 : PushButtonBlock  ButtonText=W
  Push Button22 : PushButtonBlock  ButtonText=E  OffValue=0.000000
  Push Button23 : PushButtonBlock  ButtonText=R
  Push Button24 : PushButtonBlock  ButtonText=T
  Push Button25 : PushButtonBlock  ButtonText=Y
  Push Button26 : PushButtonBlock  ButtonText=U
  Push Button27 : PushButtonBlock  ButtonText=I
  Push Button28 : PushButtonBlock  ButtonText=O
  Push Button29 : PushButtonBlock  ButtonText=P
  Push Button3 : PushButtonBlock  ButtonText=/?  OffValue=0.000000
  Push Button30 : PushButtonBlock  ButtonText=A
  Push Button31 : PushButtonBlock  ButtonText=S
  Push Button32 : PushButtonBlock  ButtonText=D
  Push Button33 : PushButtonBlock  ButtonText=F
  Push Button34 : PushButtonBlock  ButtonText=V
  Push Button35 : PushButtonBlock  ButtonText=B
  Push Button36 : PushButtonBlock  ButtonText=N
  Push Button37 : PushButtonBlock  ButtonText=M
  Push Button38 : PushButtonBlock  ButtonText=@`
  Push Button39 : PushButtonBlock  ButtonText=_
  Push Button40 : PushButtonBlock  ButtonText=\|  OffValue=0.000000
  Push Button41 : PushButtonBlock  ButtonText=^~
  Push Button42 : PushButtonBlock  ButtonText=-=
  Push Button43 : PushButtonBlock  ButtonText=SHIFT  ButtonType=Latch  OffValue=0.000000
  Push Button44 : PushButtonBlock  ButtonText=SPACE  ButtonType=Latch  OffValue=0.000000
  Push Button45 : PushButtonBlock  ButtonText=LEFT
  Push Button46 : PushButtonBlock  ButtonText=RIGHT
  Push Button47 : PushButtonBlock  ButtonText=DOWN
  Push Button48 : PushButtonBlock  ButtonText=UP
  Push Button49 : PushButtonBlock  ButtonText=]}
  Push Button50 : PushButtonBlock  ButtonText=,<
  Push Button51 : PushButtonBlock  ButtonText=╣ ╤░█  ButtonType=Latch  OffValue=0.000000
  Push Button52 : PushButtonBlock  ButtonText=&6
  Push Button53 : PushButtonBlock  ButtonText=%5
  Push Button54 : PushButtonBlock  ButtonText=+;
  Push Button55 : PushButtonBlock  ButtonText=*:
  Push Button56 : PushButtonBlock  ButtonText=Backspace
  Push Button57 : PushButtonBlock  ButtonText=$4
  Push Button58 : PushButtonBlock  ButtonText=)9
  Push Button59 : PushButtonBlock  ButtonText="\"2"
  Push Button60 : PushButtonBlock  ButtonText=[{
  Push Button61 : PushButtonBlock  ButtonText=(8
  Push Button62 : PushButtonBlock  ButtonText='7
  Push Button63 : PushButtonBlock  ButtonText=#3
  Push Button64 : PushButtonBlock  ButtonText=Enter
  Qq : Constant  Value=0  OutDataTypeStr=boolean
  Register Debug : Subsystem
  Reset : Constant  Value=0  OutDataTypeStr=boolean
  Rr : Constant  Value=0  OutDataTypeStr=boolean
  Run : Memory_Blocks_Lib/Bit_DataEnbl  SystemSampleTime=-1  VariantActivationTime=update diagram  Latency=0  AutoFrameSizeCalculation=off
  Run/Halt : Memory_Blocks_Lib/Bit_DataEnbl  SystemSampleTime=-1  VariantActivationTime=update diagram  Latency=0  AutoFrameSizeCalculation=off
  RxStateMachine : Counters_Lib/Counter_4bit_Cfg  Commented=on  SystemSampleTime=-1  VariantActivationTime=update diagram  Latency=0  AutoFrameSizeCalculation=off
  RxStates : Decoders_Lib/Dec_16  Commented=on  SystemSampleTime=-1  VariantActivationTime=update diagram  Latency=0  AutoFrameSizeCalculation=off
  Rx_Buffer : Memory_Blocks_Lib/Shift_Register  Commented=on  SystemSampleTime=-1  VariantActivationTime=update diagram  Latency=0  AutoFrameSizeCalculation=off
  Rx_Buffer_Ready : Memory_Blocks_Lib/Bit_DataEnbl  Commented=on  SystemSampleTime=-1  VariantActivationTime=update diagram  Latency=0  AutoFrameSizeCalculation=off
  "Rx_State_Machine " : Counters_Lib/Counter_4bit_Cfg  Commented=on  SystemSampleTime=-1  VariantActivationTime=update diagram  Latency=0  AutoFrameSizeCalculation=off
  STS : Constant  Commented=on  Value=0  OutDataTypeStr=boolean
  SamplingFinished(16x) : Miscellaneous/Color  SystemSampleTime=-1  VariantActivationTime=update diagram  Latency=0  AutoFrameSizeCalculation=off
  Scope : Scope
  Screen_40x25 : Subsystem  Commented=on
  Segment_Register : Subsystem
      settings: LibrarySourceBlock=Memory_Blocks_Lib/Memory_Blocks_Lib/Word
  "SelectUpperPage  " : Constant  Value=0  OutDataTypeStr=boolean
  Select_Address : Word_Multiplexers_Lib/Word_Mux_4  SystemSampleTime=-1  VariantActivationTime=update diagram  Latency=0  AutoFrameSizeCalculation=off
  "Select_Data  " : Word_Multiplexers_Lib/Word_Mux_2  SystemSampleTime=-1  VariantActivationTime=update diagram  Latency=0  AutoFrameSizeCalculation=off
  Select_Dest_Reg_Idx : Word_Multiplexers_Lib/Word_Mux_4  SystemSampleTime=-1  VariantActivationTime=update diagram  Latency=0  AutoFrameSizeCalculation=off
  Select_Immediate : Word_Multiplexers_Lib/Word_Mux_4  SystemSampleTime=-1  VariantActivationTime=update diagram  Latency=0  AutoFrameSizeCalculation=off
  Select_Src_Reg_Idx : Word_Multiplexers_Lib/Word_Mux_4  SystemSampleTime=-1  VariantActivationTime=update diagram  Latency=0  AutoFrameSizeCalculation=off
  Serial : Constant  Value=0  OutDataTypeStr=boolean
  Serial_Port_Sampling_Freq : simulink_extras/Flip Flops/Clock  period=1
  Set : Constant  OutDataTypeStr=boolean
  "Shift  " : Constant  Value=0  OutDataTypeStr=boolean
  Shift_Register (Higher_Byte) : Memory_Blocks_Lib/Shift_Register  Commented=on  SystemSampleTime=-1  VariantActivationTime=update diagram  Latency=0  AutoFrameSizeCalculation=off
  Shift_Register (Lower_Byte) : Memory_Blocks_Lib/Shift_Register  Commented=on  SystemSampleTime=-1  VariantActivationTime=update diagram  Latency=0  AutoFrameSizeCalculation=off
  Shift_Register3 : Memory_Blocks_Lib/Shift_Register  SystemSampleTime=-1  VariantActivationTime=update diagram  Latency=0  AutoFrameSizeCalculation=off
  Space/0 : Constant  Value=0  OutDataTypeStr=boolean
  Ss : Constant  Value=0  OutDataTypeStr=boolean
  Stack Debug : Subsystem
  StartBit : Constant  Commented=on  Value=0  OutDataTypeStr=boolean
  StartBitDetected (GoToStart) : Logic  Commented=on  Inputs=3  IconShape=distinctive  AllPortsSameDT=off  OutDataTypeStr=boolean
  StartBitNotDetected (GoToIdle) : Logic  Commented=on  Inputs=3  IconShape=distinctive  AllPortsSameDT=off  OutDataTypeStr=boolean
  StartVal : Memory_Blocks_Lib/Word  SystemSampleTime=-1  VariantActivationTime=update diagram  Latency=0  AutoFrameSizeCalculation=off
  StartValue : Constant  Value=0  OutDataTypeStr=uint16
  StatusFromALU : Constant  Commented=on  Value=0  OutDataTypeStr=boolean
  Status_Register : Subsystem
  Status_Register1 : Subsystem  Commented=on
  Status_TxBufferReady (will go to status register) : Terminator
  StopBit : Constant  Commented=on  OutDataTypeStr=boolean
  StopBitDetected (GoToStop) : Logic  Commented=on  Inputs=3  IconShape=distinctive  AllPortsSameDT=off  OutDataTypeStr=boolean
  StopBitNotDetected (GoToError) : Logic  Commented=on  Inputs=3  IconShape=distinctive  AllPortsSameDT=off  OutDataTypeStr=boolean
  StopVal : Memory_Blocks_Lib/Word  SystemSampleTime=-1  VariantActivationTime=update diagram  Latency=0  AutoFrameSizeCalculation=off
  Terminator{1..36,46} (37 alike) : Terminator
  Terminator{37..45} (9 alike) : Terminator  Commented=on
  Test_Outputs : Subsystem
  To Workspace1 : ToWorkspace  VariableName=instruction  SampleTime=-1
      settings: MaxDataPoints=1  Save2DSignal=2-D array (concatenate along first dimension)
  To Workspace16 : ToWorkspace  VariableName=program_counter  SampleTime=-1
      settings: MaxDataPoints=1  Save2DSignal=2-D array (concatenate along first dimension)
  To Workspace2 : ToWorkspace  VariableName=unknown_instruction  SampleTime=-1
      settings: MaxDataPoints=1  Save2DSignal=2-D array (concatenate along first dimension)
  To Workspace5 : ToWorkspace  VariableName=dest_reg_idx  SampleTime=-1
      settings: MaxDataPoints=1  Save2DSignal=2-D array (concatenate along first dimension)
  To Workspace6 : ToWorkspace  VariableName=src_reg_idx  SampleTime=-1
      settings: MaxDataPoints=1  Save2DSignal=2-D array (concatenate along first dimension)
  To Workspace7 : ToWorkspace  VariableName=keyboard  SampleTime=-1
      settings: MaxDataPoints=1  Save2DSignal=2-D array (concatenate along first dimension)
  To Workspace8 : ToWorkspace  VariableName=immediate  SampleTime=-1
      settings: MaxDataPoints=1  Save2DSignal=2-D array (concatenate along first dimension)
  Tt : Constant  Value=0  OutDataTypeStr=boolean
  Tx_Active_Latch (BlockTransmissionWhenIdle) : Memory_Blocks_Lib/Bit_DataEnbl  SystemSampleTime=-1  VariantActivationTime=update diagram  Latency=0  AutoFrameSizeCalculation=off
  Tx_Output_Buffer : Memory_Blocks_Lib/Byte  SystemSampleTime=-1  VariantActivationTime=update diagram  Latency=0  AutoFrameSizeCalculation=off
  Tx_State_Machine : Counters_Lib/Counter_4bit_Cfg  SystemSampleTime=-1  VariantActivationTime=update diagram  Latency=0  AutoFrameSizeCalculation=off
  Unknown Instruction : Logic  Operator=OR  Inputs=8  IconShape=distinctive  AllPortsSameDT=off  OutDataTypeStr=boolean
  Uu : Constant  Value=0  OutDataTypeStr=boolean
  Video_RAM (0x000 .. 0x3FF) : Subsystem
      settings: PortSchema="{\"entries\":[{\"content\":{\"sides\":[{\"content\":{\"connectorIds\":[\"In1\",\"In2\",\"In3\",\"In4\",\"In5\",\"In6\",\"In7\",\"In8\",\"In9\",\"In10\",\"In11\",\"In12\",\"In13\",\"In14\",\"In15\",\"In16\",\"In17\",\"In18\",\"In19\",\"In20\",\"In21\",\"In22\",\"In23\",\"In24\",\"In25\",\"In26\",\"In27\",\"In28\",\"In29\",\"In30\",\"In31\",\"In32\"]},\"type\":\"ConnectorPlacement.EquallySpacedRectSide\",\"uuid\":\"1eaf8664-d966-4015-add6-8fc8ededb4cf\"},{\"content\":{\"connectorIds\":[\"In74\",\"Out1\",\"Out2\",\"Out3\",\"Out4\",\"Out5\",\"Out6\",\"Out7\",\"Out8\",\"Out9\"],\"side\":\"RIGHT\"},\"type\":\"ConnectorPlacement.EquallySpacedRectSide\",\"uuid\":\"3c4416de-c171-4f92-9892-106dbfd5c35b\"},{\"content\":{\"connectorIds\":[\"In33\",\"In34\",\"In35\",\"In36\",\"In37\",\"In38\",\"In39\",\"In40\",\"In41\",\"In42\",\"In43\",\"In44\",\"In45\",\"In46\",\"In47\",\"In48\",\"In49\",\"In50\",\"In51\",\"In52\",\"In53\",\"In54\",\"In55\",\"In56\",\"In57\",\"In58\",\"In59\",\"In60\",\"In61\",\"In62\",\"In63\",\"In64\"],\"side\":\"TOP\"},\"type\":\"ConnectorPlacement.EquallySpacedRectSide\",\"uuid\":\"6f02514a-f13d-46d7-86d2-212fd71e0356\"},{\"content\":{\"connectorIds\":[\"In65\",\"In66\",\"In67\",\"In68\",\"In69\",\"In70\",\"In71\",\"In72\",\"In73\"],\"side\":\"BOTTOM\"},\"type\":\"ConnectorPlacement.EquallySpacedRectSide\",\"uuid\":\"2ea63344-e6d7-4ee2-99d1-4b7c6fc28cc8\"}]},\"type\":\"ConnectorPlacement.EquallySpacedConnector\",\"uuid\":\"dd0fe977-d8de-4751-ab8c-29f8f242b401\"}],\"packageUris\":[\"http://schema.mathworks.com/mf0/Connector/R2020b\"],\"version\":\"1.0\"}"
  Vv : Constant  Value=0  OutDataTypeStr=boolean
  Word_00 : Memory_Blocks_Lib/Word  SystemSampleTime=-1  VariantActivationTime=update diagram  Latency=0  AutoFrameSizeCalculation=off
      settings: LibrarySourceBlock=Memory_Blocks_Lib/Memory_Blocks_Lib/Word
  Word_01 : Memory_Blocks_Lib/Word  SystemSampleTime=-1  VariantActivationTime=update diagram  Latency=0  AutoFrameSizeCalculation=off
      settings: LibrarySourceBlock=Memory_Blocks_Lib/Memory_Blocks_Lib/Word
  Word_02 : Memory_Blocks_Lib/Word  SystemSampleTime=-1  VariantActivationTime=update diagram  Latency=0  AutoFrameSizeCalculation=off
      settings: LibrarySourceBlock=Memory_Blocks_Lib/Memory_Blocks_Lib/Word
  Word_03 : Memory_Blocks_Lib/Word  SystemSampleTime=-1  VariantActivationTime=update diagram  Latency=0  AutoFrameSizeCalculation=off
      settings: LibrarySourceBlock=Memory_Blocks_Lib/Memory_Blocks_Lib/Word
  Word_04 : Memory_Blocks_Lib/Word  SystemSampleTime=-1  VariantActivationTime=update diagram  Latency=0  AutoFrameSizeCalculation=off
      settings: LibrarySourceBlock=Memory_Blocks_Lib/Memory_Blocks_Lib/Word
  Word_05 : Memory_Blocks_Lib/Word  SystemSampleTime=-1  VariantActivationTime=update diagram  Latency=0  AutoFrameSizeCalculation=off
      settings: LibrarySourceBlock=Memory_Blocks_Lib/Memory_Blocks_Lib/Word
  Word_06 : Memory_Blocks_Lib/Word  SystemSampleTime=-1  VariantActivationTime=update diagram  Latency=0  AutoFrameSizeCalculation=off
      settings: LibrarySourceBlock=Memory_Blocks_Lib/Memory_Blocks_Lib/Word
  Word_07 : Memory_Blocks_Lib/Word  SystemSampleTime=-1  VariantActivationTime=update diagram  Latency=0  AutoFrameSizeCalculation=off
      settings: LibrarySourceBlock=Memory_Blocks_Lib/Memory_Blocks_Lib/Word
  Word_08 : Memory_Blocks_Lib/Word  SystemSampleTime=-1  VariantActivationTime=update diagram  Latency=0  AutoFrameSizeCalculation=off
      settings: LibrarySourceBlock=Memory_Blocks_Lib/Memory_Blocks_Lib/Word
  Word_09 : Memory_Blocks_Lib/Word  SystemSampleTime=-1  VariantActivationTime=update diagram  Latency=0  AutoFrameSizeCalculation=off
      settings: LibrarySourceBlock=Memory_Blocks_Lib/Memory_Blocks_Lib/Word
  Word_{10..15} (6 alike) : Memory_Blocks_Lib/Word  SystemSampleTime=-1  VariantActivationTime=update diagram  Latency=0  AutoFrameSizeCalculation=off
      settings: LibrarySourceBlock=Memory_Blocks_Lib/Memory_Blocks_Lib/Word
  Word_Enable{,1..26} (27 alike) : Miscellaneous/Word_Enable  SystemSampleTime=-1  VariantActivationTime=update diagram  Latency=0  AutoFrameSizeCalculation=off
  Word_Enable27 : Subsystem
  Word_Enable28 : Subsystem
  Word_Enable29 : Subsystem
  Word_Enable30 : Subsystem
  Word_Enable32 : Subsystem
  Word_Enable33 : Subsystem
  Word_Enable34 : Subsystem
  Word_Enable35 : Subsystem
  Word_Enable36 : Subsystem
  Word_Multiplexer_2_to_1 DirSel(00) : Word_Multiplexers_Lib/Word_Mux_2  SystemSampleTime=-1  VariantActivationTime=update diagram  Latency=0  AutoFrameSizeCalculation=off
      settings: LibrarySourceBlock=Word_Multiplexers_Lib/Word_Multiplexers_Lib/Word_Multiplexer_2_to_1_DirSel
  Word_Multiplexer_2_to_1 DirSel(01) : Word_Multiplexers_Lib/Word_Mux_2  SystemSampleTime=-1  VariantActivationTime=update diagram  Latency=0  AutoFrameSizeCalculation=off
      settings: LibrarySourceBlock=Word_Multiplexers_Lib/Word_Multiplexers_Lib/Word_Multiplexer_2_to_1_DirSel
  Word_Multiplexer_2_to_1 DirSel(02) : Word_Multiplexers_Lib/Word_Mux_2  SystemSampleTime=-1  VariantActivationTime=update diagram  Latency=0  AutoFrameSizeCalculation=off
      settings: LibrarySourceBlock=Word_Multiplexers_Lib/Word_Multiplexers_Lib/Word_Multiplexer_2_to_1_DirSel
  Word_Multiplexer_2_to_1 DirSel(03) : Word_Multiplexers_Lib/Word_Mux_2  SystemSampleTime=-1  VariantActivationTime=update diagram  Latency=0  AutoFrameSizeCalculation=off
      settings: LibrarySourceBlock=Word_Multiplexers_Lib/Word_Multiplexers_Lib/Word_Multiplexer_2_to_1_DirSel
  Word_Multiplexer_2_to_1 DirSel(04) : Word_Multiplexers_Lib/Word_Mux_2  SystemSampleTime=-1  VariantActivationTime=update diagram  Latency=0  AutoFrameSizeCalculation=off
      settings: LibrarySourceBlock=Word_Multiplexers_Lib/Word_Multiplexers_Lib/Word_Multiplexer_2_to_1_DirSel
  Word_Multiplexer_2_to_1 DirSel(05) : Word_Multiplexers_Lib/Word_Mux_2  SystemSampleTime=-1  VariantActivationTime=update diagram  Latency=0  AutoFrameSizeCalculation=off
      settings: LibrarySourceBlock=Word_Multiplexers_Lib/Word_Multiplexers_Lib/Word_Multiplexer_2_to_1_DirSel
  Word_Multiplexer_2_to_1 DirSel(06){,1..9} (10 alike) : Word_Multiplexers_Lib/Word_Mux_2  SystemSampleTime=-1  VariantActivationTime=update diagram  Latency=0  AutoFrameSizeCalculation=off
      settings: LibrarySourceBlock=Word_Multiplexers_Lib/Word_Multiplexers_Lib/Word_Multiplexer_2_to_1_DirSel
  Word_Mux_1 : Word_Multiplexers_Lib/Word_Mux_2  SystemSampleTime=-1  VariantActivationTime=update diagram  Latency=0  AutoFrameSizeCalculation=off
  Word_Mux_2 : Word_Multiplexers_Lib/Word_Mux_4  SystemSampleTime=-1  VariantActivationTime=update diagram  Latency=0  AutoFrameSizeCalculation=off
  Word_Mux_3 : Word_Multiplexers_Lib/Word_Mux_4  SystemSampleTime=-1  VariantActivationTime=update diagram  Latency=0  AutoFrameSizeCalculation=off
  Word_Mux_4 : Word_Multiplexers_Lib/Word_Mux_2  SystemSampleTime=-1  VariantActivationTime=update diagram  Latency=0  AutoFrameSizeCalculation=off
  Word_Mux_4(6) : Word_Multiplexers_Lib/Word_Mux_4  SystemSampleTime=-1  VariantActivationTime=update diagram  Latency=0  AutoFrameSizeCalculation=off
  Word_Mux_5 : Word_Multiplexers_Lib/Word_Mux_2  SystemSampleTime=-1  VariantActivationTime=update diagram  Latency=0  AutoFrameSizeCalculation=off
  Word_Mux_6 : Word_Multiplexers_Lib/Word_Mux_2  Commented=on  SystemSampleTime=-1  VariantActivationTime=update diagram  Latency=0  AutoFrameSizeCalculation=off
  Word_Mux_7 : Word_Multiplexers_Lib/Word_Mux_4  SystemSampleTime=-1  VariantActivationTime=update diagram  Latency=0  AutoFrameSizeCalculation=off
  Write : Logic  Operator=OR  IconShape=distinctive  AllPortsSameDT=off  OutDataTypeStr=boolean
  Ww : Constant  Value=0  OutDataTypeStr=boolean
  Xx : Constant  Value=0  OutDataTypeStr=boolean
  Yy : Constant  Value=0  OutDataTypeStr=boolean
  Zz : Constant  Value=0  OutDataTypeStr=boolean
  "[{" : Constant  Value=0  OutDataTypeStr=boolean
  \| : Constant  Value=0  OutDataTypeStr=boolean
  "]}" : Constant  Value=0  OutDataTypeStr=boolean
  ^~ : Constant  Value=0  OutDataTypeStr=boolean
  _ : Constant  Value=0  OutDataTypeStr=boolean
  bus_to_uint(byte) : Miscellaneous/bus_to_uint(byte)
  bus_to_uint(word) : Miscellaneous/bus_to_uint(word)  Commented=on
  logic : Logic  Operator=OR  IconShape=distinctive  AllPortsSameDT=off  OutDataTypeStr=boolean
  not{,1..3} (4 alike) : Logic  Operator=NOT  IconShape=distinctive  AllPortsSameDT=off  OutDataTypeStr=boolean
  uint_to_bus{,1..7} (8 alike) : Miscellaneous/uint_to_bus(word)
      settings: LibrarySourceBlock=Miscellaneous/uint_to_bus
  uint_to_bus(byte)1 : Miscellaneous/uint_to_bus(byte)  Commented=on  SystemSampleTime=-1  VariantActivationTime=update diagram  Latency=0  AutoFrameSizeCalculation=off
  uint_to_bus(byte)2 : Miscellaneous/uint_to_bus(byte)  SystemSampleTime=-1  VariantActivationTime=update diagram  Latency=0  AutoFrameSizeCalculation=off
  uint_to_bus(byte)4 : Miscellaneous/uint_to_bus(byte)  SystemSampleTime=-1  VariantActivationTime=update diagram  Latency=0  AutoFrameSizeCalculation=off
  uint_to_bus(byte)5 : Miscellaneous/uint_to_bus(byte)  Commented=on  SystemSampleTime=-1  VariantActivationTime=update diagram  Latency=0  AutoFrameSizeCalculation=off
  uint_to_bus(byte)6 : Miscellaneous/uint_to_bus(byte)  Commented=on  SystemSampleTime=-1  VariantActivationTime=update diagram  Latency=0  AutoFrameSizeCalculation=off
  uint_to_bus(word)1 : Miscellaneous/uint_to_bus(word)  Commented=on
  uint_to_bus(word)2 : Miscellaneous/uint_to_bus(word)  Commented=on
  uint_to_bus(word)3 : Miscellaneous/uint_to_bus(word)  Commented=on
  uint_to_bus(word)4 : Miscellaneous/uint_to_bus(word)
  undef Down : Constant  Value=0  OutDataTypeStr=boolean
  undef Left : Constant  Value=0  OutDataTypeStr=boolean
  undef Up : Constant  Value=0  OutDataTypeStr=boolean
  wires:
  <0x1000..0x1FFF>/1(Sel(1b)) -> Word_Enable35/1(Sel(1b)), Logical Operator14/2, Logical Operator54/2
  Dec_32_Enbl4/31 -> Instruction_ROM (0x000 .. 0xFFF)/127(X01)
  Dec_32_Enbl5/29 -> Instruction_ROM (0x000 .. 0xFFF)/93(X35)
  Bus Selector7/3 -> Logical Operator18/3, Logical Operator11/2  "<CALL>"
  Logical Operator32/1 -> Dec_32_Enbl4/1
  Word_Mux_4/2 -> AuxALU/1
  Dec_32_Enbl6/27 -> Instruction_ROM (0x000 .. 0xFFF)/59(Y05)
  Bus Selector3/5 -> Logical Operator2/1, Logical Operator16/1, Logical Operator15/1  "<STL>"
  Align61/4 -> Dec_32_Enbl4/4, Dec_32_Enbl5/4
  Dec_32_Enbl4/14 -> Instruction_ROM (0x000 .. 0xFFF)/110(X18)
  Dec_32_Enbl4/13 -> Instruction_ROM (0x000 .. 0xFFF)/109(X19)
  Bus Selector3/3 -> Logical Operator3/3, Logical Operator16/3, Logical Operator15/3  "<STLI>"
  Dec_32_Enbl6/32 -> Instruction_ROM (0x000 .. 0xFFF)/64(Y00)
  Dec_32_Enbl5/31 -> Instruction_ROM (0x000 .. 0xFFF)/95(X33)
  Dec_32_Enbl6/10 -> Instruction_ROM (0x000 .. 0xFFF)/42(Y22)
  Dec_32_Enbl4/5 -> Instruction_ROM (0x000 .. 0xFFF)/101(X27)
  Dec_32_Enbl4/10 -> Instruction_ROM (0x000 .. 0xFFF)/106(X22)
  Align6/1 -> Dec_32_Enbl7/6, Dec_32_Enbl6/6
  Dec_32_Enbl7/12 -> Instruction_ROM (0x000 .. 0xFFF)/12(Y52)
  Dec_32_Enbl7/1 -> Instruction_ROM (0x000 .. 0xFFF)/1(Y63)
  Dec_32_Enbl5/13 -> Instruction_ROM (0x000 .. 0xFFF)/77(X51)
  Logical Operator26/1 -> Video_RAM (0x000 .. 0x3FF)/74(Write(1b))
  Dec_32_Enbl5/19 -> Instruction_ROM (0x000 .. 0xFFF)/83(X45)
  Dec_32_Enbl5/27 -> Instruction_ROM (0x000 .. 0xFFF)/91(X37)
  Bus Creator23/1 -> Select_Address/8  "SrcRegVal"
  Dec_32_Enbl5/30 -> Instruction_ROM (0x000 .. 0xFFF)/94(X34)
  Dec_32_Enbl7/27 -> Instruction_ROM (0x000 .. 0xFFF)/27(Y37)
  Dec_32_Enbl5/17 -> Instruction_ROM (0x000 .. 0xFFF)/81(X47)
  Dec_32_Enbl7/28 -> Instruction_ROM (0x000 .. 0xFFF)/28(Y36)
  Dec_32_Enbl4/19 -> Instruction_ROM (0x000 .. 0xFFF)/115(X13)
  Dec_32_Enbl5/4 -> Instruction_ROM (0x000 .. 0xFFF)/68(X60)
  Dec_32_Enbl7/8 -> Instruction_ROM (0x000 .. 0xFFF)/8(Y56)
  Align6/6 -> Dec_32_Enbl7/1, Logical Operator31/1
  Dec_32_Enbl5/21 -> Instruction_ROM (0x000 .. 0xFFF)/85(X43)
  Dec_32_Enbl5/24 -> Instruction_ROM (0x000 .. 0xFFF)/88(X40)
  Logical Operator11/1 -> Mux_4/3
  Dec_32_Enbl6/19 -> Instruction_ROM (0x000 .. 0xFFF)/51(Y13)
  Dec_32_Enbl4/30 -> Instruction_ROM (0x000 .. 0xFFF)/126(X02)
  Dec_32_Enbl4/17 -> Instruction_ROM (0x000 .. 0xFFF)/113(X15)
  Dec_32_Enbl5/10 -> Instruction_ROM (0x000 .. 0xFFF)/74(X54)
  Dec_32_Enbl7/30 -> Instruction_ROM (0x000 .. 0xFFF)/30(Y34)
  Dec_32_Enbl7/21 -> Instruction_ROM (0x000 .. 0xFFF)/21(Y43)
  Dec_32_Enbl5/5 -> Instruction_ROM (0x000 .. 0xFFF)/69(X59)
  Dec_32_Enbl7/13 -> Instruction_ROM (0x000 .. 0xFFF)/13(Y51)
  Align71/1 -> Logical Operator9/1
  Dec_32_Enbl6/9 -> Instruction_ROM (0x000 .. 0xFFF)/41(Y23)
  Dec_32_Enbl6/24 -> Instruction_ROM (0x000 .. 0xFFF)/56(Y08)
  Dec_32_Enbl7/20 -> Instruction_ROM (0x000 .. 0xFFF)/20(Y44)
  Logical Operator31/1 -> Dec_32_Enbl6/1
  Dec_32_Enbl6/5 -> Instruction_ROM (0x000 .. 0xFFF)/37(Y27)
  Dec_32_Enbl7/10 -> Instruction_ROM (0x000 .. 0xFFF)/10(Y54)
  Dec_32_Enbl7/23 -> Instruction_ROM (0x000 .. 0xFFF)/23(Y41)
  Dec_32_Enbl7/16 -> Instruction_ROM (0x000 .. 0xFFF)/16(Y48)
  uint_to_bus1/1 -> Word_Mux_4/4
  Dec_32_Enbl5/2 -> Instruction_ROM (0x000 .. 0xFFF)/66(X62)
  Dec_32_Enbl7/26 -> Instruction_ROM (0x000 .. 0xFFF)/26(Y38)
  Dec_32_Enbl4/2 -> Instruction_ROM (0x000 .. 0xFFF)/98(X30)
  Align6/2 -> Dec_32_Enbl7/5, Dec_32_Enbl6/5
  Constant7/1 -> Select_Address/5
  Dec_32_Enbl5/3 -> Instruction_ROM (0x000 .. 0xFFF)/67(X61)
  Bus Selector5/1 -> Word_Mux_4(6)/3, Logical Operator36/2  "<PUSH>"
  Bus Selector3/9 -> Logical Operator4/1, Logical Operator17/1  "<LDL>"
  Align61/6 -> Dec_32_Enbl4/6, Dec_32_Enbl5/6
  Dec_32_Enbl7/6 -> Instruction_ROM (0x000 .. 0xFFF)/6(Y58)
  Dec_32_Enbl4/27 -> Instruction_ROM (0x000 .. 0xFFF)/123(X05)
  Dec_32_Enbl4/32 -> Instruction_ROM (0x000 .. 0xFFF)/128(X00)
  Dec_32_Enbl4/23 -> Instruction_ROM (0x000 .. 0xFFF)/119(X09)
  Dec_32_Enbl4/24 -> Instruction_ROM (0x000 .. 0xFFF)/120(X08)
  <0xFFFE..0xFFFE>/1(Sel(1b)) -> Word_Enable28/1(Sel(1b))
  Dec_32_Enbl5/22 -> Instruction_ROM (0x000 .. 0xFFF)/86(X42)
  Dec_32_Enbl7/4 -> Instruction_ROM (0x000 .. 0xFFF)/4(Y60)
  Bus Selector3/4 -> Logical Operator2/2, Logical Operator16/2, Logical Operator15/2  "<STU>"
  Select_Src_Reg_Idx/2 -> Bus Selector29/1, Bit to Integer Converter7/1  "SrcRegIdx"
  Dec_32_Enbl5/32 -> Instruction_ROM (0x000 .. 0xFFF)/96(X32)
  Dec_32_Enbl6/25 -> Instruction_ROM (0x000 .. 0xFFF)/57(Y07)
  Dec_32_Enbl6/30 -> Instruction_ROM (0x000 .. 0xFFF)/62(Y02)
  Dec_32_Enbl5/8 -> Instruction_ROM (0x000 .. 0xFFF)/72(X56)
  Dec_32_Enbl4/4 -> Instruction_ROM (0x000 .. 0xFFF)/100(X28)
  Bus Selector5/3 -> Logical Operator34/1  "<POP>"
  Dec_32_Enbl7/19 -> Instruction_ROM (0x000 .. 0xFFF)/19(Y45)
  Dec_32_Enbl4/7 -> Instruction_ROM (0x000 .. 0xFFF)/103(X25)
  Align6/5 -> Dec_32_Enbl7/2, Dec_32_Enbl6/2
  Dec_32_Enbl6/28 -> Instruction_ROM (0x000 .. 0xFFF)/60(Y04)
  Dec_32_Enbl7/17 -> Instruction_ROM (0x000 .. 0xFFF)/17(Y47)
  Dec_32_Enbl7/31 -> Instruction_ROM (0x000 .. 0xFFF)/31(Y33)
  Dec_32_Enbl6/8 -> Instruction_ROM (0x000 .. 0xFFF)/40(Y24)
  Dec_32_Enbl6/16 -> Instruction_ROM (0x000 .. 0xFFF)/48(Y16)
  Dec_32_Enbl7/5 -> Instruction_ROM (0x000 .. 0xFFF)/5(Y59)
  Word_Mux_5/2 -> AuxALU/2
  Dec_32_Enbl5/12 -> Instruction_ROM (0x000 .. 0xFFF)/76(X52)
  Dec_32_Enbl6/20 -> Instruction_ROM (0x000 .. 0xFFF)/52(Y12)
  Dec_32_Enbl5/16 -> Instruction_ROM (0x000 .. 0xFFF)/80(X48)
  Logical Operator38/1 -> Word_Mux_5/1, Word_Mux_4/1
  Bus Selector7/1 -> Logical Operator18/5, Mux_4/4  "<RET>"
  Dec_32_Enbl5/18 -> Instruction_ROM (0x000 .. 0xFFF)/82(X46)
  Dec_32_Enbl5/28 -> Instruction_ROM (0x000 .. 0xFFF)/92(X36)
  Dec_32_Enbl4/3 -> Instruction_ROM (0x000 .. 0xFFF)/99(X29)
  Dec_32_Enbl4/11 -> Instruction_ROM (0x000 .. 0xFFF)/107(X21)
  Dec_32_Enbl4/6 -> Instruction_ROM (0x000 .. 0xFFF)/102(X26)
  Constant9/1 -> Select_Address/1
  Dec_32_Enbl6/15 -> Instruction_ROM (0x000 .. 0xFFF)/47(Y17)
  Dec_32_Enbl6/23 -> Instruction_ROM (0x000 .. 0xFFF)/55(Y09)
  Align61/3 -> Dec_32_Enbl4/3, Dec_32_Enbl5/3
  Dec_32_Enbl5/26 -> Instruction_ROM (0x000 .. 0xFFF)/90(X38)
  Dec_32_Enbl6/29 -> Instruction_ROM (0x000 .. 0xFFF)/61(Y03)
  Dec_32_Enbl7/25 -> Instruction_ROM (0x000 .. 0xFFF)/25(Y39)
  Select_Dest_Reg_Idx/2 -> Bus Selector30/1, Bit to Integer Converter4/1  "DestRegIdx"
  Bus Selector3/8 -> Logical Operator4/2, Logical Operator17/2  "<LDU>"
  Logical Operator16/1 -> Align46/2
  Bus Selector5/4 -> Logical Operator34/2  "<RET>"
  Bus Selector3/6 -> Logical Operator3/2, Logical Operator17/4  "<LDUI>"
  Dec_32_Enbl5/20 -> Instruction_ROM (0x000 .. 0xFFF)/84(X44)
  Dec_32_Enbl5/15 -> Instruction_ROM (0x000 .. 0xFFF)/79(X49)
  Bus Selector8/2 -> Logical Operator38/2  "<STLI>"
  AuxALU/2 -> GreaterThan(1b)/1
  Dec_32_Enbl5/6 -> Instruction_ROM (0x000 .. 0xFFF)/70(X58)
  Bus Selector7/2 -> Logical Operator18/4, Logical Operator11/1  "<JMP>"
  Dec_32_Enbl5/23 -> Instruction_ROM (0x000 .. 0xFFF)/87(X41)
  Logical Operator15/1 -> "Select_Data  "/2
  Dec_32_Enbl4/28 -> Instruction_ROM (0x000 .. 0xFFF)/124(X04)
  Dec_32_Enbl4/22 -> Instruction_ROM (0x000 .. 0xFFF)/118(X10)
  Dec_32_Enbl7/7 -> Instruction_ROM (0x000 .. 0xFFF)/7(Y57)
  Align61/2 -> Dec_32_Enbl4/2, Dec_32_Enbl5/2
  Dec_32_Enbl6/22 -> Instruction_ROM (0x000 .. 0xFFF)/54(Y10)
  Align6/4 -> Dec_32_Enbl6/3, Dec_32_Enbl7/3
  Bus Selector7/5 -> Logical Operator24/2  "<JLT>"
  Dec_32_Enbl7/24 -> Instruction_ROM (0x000 .. 0xFFF)/24(Y40)
  Dec_32_Enbl5/7 -> Instruction_ROM (0x000 .. 0xFFF)/71(X57)
  Dec_32_Enbl4/29 -> Instruction_ROM (0x000 .. 0xFFF)/125(X03)
  Dec_32_Enbl6/3 -> Instruction_ROM (0x000 .. 0xFFF)/35(Y29)
  Bus Creator26/1 -> Select_Address/7  "DestRegVal"
  Dec_32_Enbl7/2 -> Instruction_ROM (0x000 .. 0xFFF)/2(Y62)
  Dec_32_Enbl7/29 -> Instruction_ROM (0x000 .. 0xFFF)/29(Y35)
  Dec_32_Enbl6/26 -> Instruction_ROM (0x000 .. 0xFFF)/58(Y06)
  Logical Operator9/1 -> Logical Operator18/2, Logical Operator11/3
  Dec_32_Enbl6/17 -> Instruction_ROM (0x000 .. 0xFFF)/49(Y15)
  Dec_32_Enbl7/32 -> Instruction_ROM (0x000 .. 0xFFF)/32(Y32)
  Dec_32_Enbl7/14 -> Instruction_ROM (0x000 .. 0xFFF)/14(Y50)
  Dec_32_Enbl7/3 -> Instruction_ROM (0x000 .. 0xFFF)/3(Y61)
  Dec_32_Enbl5/1 -> Instruction_ROM (0x000 .. 0xFFF)/65(X63)
  Word_00/1 -> Stack Debug/1(In1), Word_Multiplexer_2_to_1 DirSel(01)/4  "Stack"
  Dec_32_Enbl6/7 -> Instruction_ROM (0x000 .. 0xFFF)/39(Y25)
  Dec_32_Enbl4/20 -> Instruction_ROM (0x000 .. 0xFFF)/116(X12)
  Dec_32_Enbl5/14 -> Instruction_ROM (0x000 .. 0xFFF)/78(X50)
  Bus Selector3/2 -> Logical Operator3/4, Logical Operator16/4, Logical Operator15/4  "<STUI>"
  Dec_32_Enbl6/1 -> Instruction_ROM (0x000 .. 0xFFF)/33(Y31)
  Dec_32_Enbl4/26 -> Instruction_ROM (0x000 .. 0xFFF)/122(X06)
  Dec_32_Enbl4/18 -> Instruction_ROM (0x000 .. 0xFFF)/114(X14)
  Dec_32_Enbl7/11 -> Instruction_ROM (0x000 .. 0xFFF)/11(Y53)
  Logical Operator4/1 -> Select_Address/4
  Dec_32_Enbl5/11 -> Instruction_ROM (0x000 .. 0xFFF)/75(X53)
  Dec_32_Enbl6/6 -> Instruction_ROM (0x000 .. 0xFFF)/38(Y26)
  Dec_32_Enbl6/31 -> Instruction_ROM (0x000 .. 0xFFF)/63(Y01)
  Dec_32_Enbl6/14 -> Instruction_ROM (0x000 .. 0xFFF)/46(Y18)
  Dec_32_Enbl5/9 -> Instruction_ROM (0x000 .. 0xFFF)/73(X55)
  Dec_32_Enbl6/4 -> Instruction_ROM (0x000 .. 0xFFF)/36(Y28)
  Align6/3 -> Dec_32_Enbl7/4, Dec_32_Enbl6/4
  Dec_32_Enbl5/25 -> Instruction_ROM (0x000 .. 0xFFF)/89(X39)
  Dec_32_Enbl6/11 -> Instruction_ROM (0x000 .. 0xFFF)/43(Y21)
  Align71/2 -> Logical Operator24/1
  Align59/16 -> Bus Creator12/16
  Dec_32_Enbl6/2 -> Instruction_ROM (0x000 .. 0xFFF)/34(Y30)
  Dec_32_Enbl4/16 -> Instruction_ROM (0x000 .. 0xFFF)/112(X16)
  Bus Selector8/4 -> Logical Operator38/4  "<LDLI>"
  Dec_32_Enbl7/18 -> Instruction_ROM (0x000 .. 0xFFF)/18(Y46)
  Bus Selector3/7 -> Logical Operator3/1, Logical Operator17/3  "<LDLI>"
  Bus Selector7/4 -> Logical Operator9/2  "<JPE>"
  Dec_32_Enbl4/9 -> Instruction_ROM (0x000 .. 0xFFF)/105(X23)
  Dec_32_Enbl6/13 -> Instruction_ROM (0x000 .. 0xFFF)/45(Y19)
  Bus Selector5/2 -> Word_Mux_4(6)/2, Logical Operator36/3  "<CALL>"
  Dec_32_Enbl4/12 -> Instruction_ROM (0x000 .. 0xFFF)/108(X20)
  Align61/5 -> Dec_32_Enbl4/5, Dec_32_Enbl5/5
  Dec_32_Enbl4/15 -> Instruction_ROM (0x000 .. 0xFFF)/111(X17)
  Dec_32_Enbl6/12 -> Instruction_ROM (0x000 .. 0xFFF)/44(Y20)
  Dec_32_Enbl4/8 -> Instruction_ROM (0x000 .. 0xFFF)/104(X24)
  Video_RAM (0x000 .. 0x3FF)/1(Video(1000B)) -> Screen_40x25/1(Data(1000B))
  Dec_32_Enbl4/25 -> Instruction_ROM (0x000 .. 0xFFF)/121(X07)
  Bus Selector8/1 -> Logical Operator38/1  "<STUI>"
  Bus Creator22/1 -> Word_Mux_4(6)/7
  Dec_32_Enbl7/22 -> Instruction_ROM (0x000 .. 0xFFF)/22(Y42)
  Dec_32_Enbl4/21 -> Instruction_ROM (0x000 .. 0xFFF)/117(X11)
  Dec_32_Enbl7/9 -> Instruction_ROM (0x000 .. 0xFFF)/9(Y55)
  Bus Selector8/3 -> Logical Operator38/3  "<LDUI>"
  Dec_32_Enbl6/21 -> Instruction_ROM (0x000 .. 0xFFF)/53(Y11)
  Dec_32_Enbl6/18 -> Instruction_ROM (0x000 .. 0xFFF)/50(Y14)
  Logical Operator2/1 -> Select_Address/3
  Logical Operator24/1 -> Logical Operator18/1, Logical Operator11/4
  Align61/1 -> Dec_32_Enbl5/1, Logical Operator32/1
  Dec_32_Enbl7/15 -> Instruction_ROM (0x000 .. 0xFFF)/15(Y49)
  Logical Operator3/1 -> Select_Address/2
  Dec_32_Enbl4/1 -> Instruction_ROM (0x000 .. 0xFFF)/97(X31)
  Logical Operator36/1 -> Word_Multiplexer_2_to_1 DirSel(06)9/1, Word_Multiplexer_2_to_1 DirSel(06)6/1, Word_Multiplexer_2_to_1 DirSel(06)5/1, Word_Multiplexer_2_to_1 DirSel(06)1/1, Word_Multiplexer_2_to_1 DirSel(06)/1, Word_Multiplexer_2_to_1 DirSel(00)/1, Word_Multiplexer_2_to_1 DirSel(01)/1, Word_Multiplexer_2_to_1 DirSel(02)/1, Word_Multiplexer_2_to_1 DirSel(03)/1, Word_Multiplexer_2_to_1 DirSel(04)/1, Word_Multiplexer_2_to_1 DirSel(05)/1, Word_Multiplexer_2_to_1 DirSel(06)2/1, Word_Multiplexer_2_to_1 DirSel(06)3/1, Word_Multiplexer_2_to_1 DirSel(06)4/1, Word_Multiplexer_2_to_1 DirSel(06)7/1, Word_Multiplexer_2_to_1 DirSel(06)8/1, Write/1
  Logical Operator34/1 -> Word_Multiplexer_2_to_1 DirSel(00)/2, Word_Multiplexer_2_to_1 DirSel(01)/2, Word_Multiplexer_2_to_1 DirSel(02)/2, Word_Multiplexer_2_to_1 DirSel(03)/2, Word_Multiplexer_2_to_1 DirSel(04)/2, Word_Multiplexer_2_to_1 DirSel(05)/2, Word_Multiplexer_2_to_1 DirSel(06)/2, Word_Multiplexer_2_to_1 DirSel(06)1/2, Word_Multiplexer_2_to_1 DirSel(06)2/2, Word_Multiplexer_2_to_1 DirSel(06)3/2, Word_Multiplexer_2_to_1 DirSel(06)4/2, Word_Multiplexer_2_to_1 DirSel(06)5/2, Word_Multiplexer_2_to_1 DirSel(06)6/2, Word_Multiplexer_2_to_1 DirSel(06)7/2, Word_Multiplexer_2_to_1 DirSel(06)8/2, Word_Multiplexer_2_to_1 DirSel(06)9/2, Write/2
  Write/1 -> Word_15/2, Word_00/2, Word_00/1, Word_01/2, Word_01/1, Word_02/2, Word_02/1, Word_03/2, Word_03/1, Word_04/2, Word_04/1, Word_05/2, Word_05/1, Word_06/2, Word_06/1, Word_07/2, Word_07/1, Word_08/2, Word_08/1, Word_09/2, Word_09/1, Word_10/2, Word_10/1, Word_11/2, Word_11/1, Word_12/2, Word_12/1, Word_13/2, Word_13/1, Word_14/2, Word_14/1, Word_15/1
  Word_Multiplexer_2_to_1 DirSel(00)/2 -> Word_00/3
  Word_01/1 -> Stack Debug/2(In16), Word_Multiplexer_2_to_1 DirSel(00)/3, Word_Multiplexer_2_to_1 DirSel(02)/4
  Constant10/1 -> Word_Multiplexer_2_to_1 DirSel(00)/4
  Word_Mux_4(6)/2 -> Word_Multiplexer_2_to_1 DirSel(06)9/3
  Word_09/1 -> Word_Multiplexer_2_to_1 DirSel(06)2/3, Stack Debug/10(In8), Word_Multiplexer_2_to_1 DirSel(06)4/4
  Word_Multiplexer_2_to_1 DirSel(06)9/2 -> Word_15/3
  Word_Multiplexer_2_to_1 DirSel(06)8/2 -> Word_14/3
  Word_Multiplexer_2_to_1 DirSel(06)7/2 -> Word_13/3
  Word_Multiplexer_2_to_1 DirSel(06)6/2 -> Word_12/3
  Word_Multiplexer_2_to_1 DirSel(06)5/2 -> Word_11/3
  Word_Multiplexer_2_to_1 DirSel(06)4/2 -> Word_10/3
  Word_Multiplexer_2_to_1 DirSel(06)3/2 -> Word_09/3
  Word_Multiplexer_2_to_1 DirSel(06)2/2 -> Word_08/3
  Word_Multiplexer_2_to_1 DirSel(06)1/2 -> Word_07/3
  Word_Multiplexer_2_to_1 DirSel(06)/2 -> Word_06/3
  Word_Multiplexer_2_to_1 DirSel(05)/2 -> Word_05/3
  Word_Multiplexer_2_to_1 DirSel(04)/2 -> Word_04/3
  Word_Multiplexer_2_to_1 DirSel(03)/2 -> Word_03/3
  Word_Multiplexer_2_to_1 DirSel(02)/2 -> Word_02/3
  Word_Multiplexer_2_to_1 DirSel(01)/2 -> Word_01/3
  Word_14/1 -> Word_Multiplexer_2_to_1 DirSel(06)7/3, Stack Debug/15(In3), Word_Multiplexer_2_to_1 DirSel(06)9/4
  Word_13/1 -> Word_Multiplexer_2_to_1 DirSel(06)6/3, Stack Debug/14(In4), Word_Multiplexer_2_to_1 DirSel(06)8/4
  Word_12/1 -> Word_Multiplexer_2_to_1 DirSel(06)5/3, Stack Debug/13(In5), Word_Multiplexer_2_to_1 DirSel(06)7/4
  Word_11/1 -> Word_Multiplexer_2_to_1 DirSel(06)4/3, Stack Debug/12(In6), Word_Multiplexer_2_to_1 DirSel(06)6/4
  Word_10/1 -> Word_Multiplexer_2_to_1 DirSel(06)3/3, Stack Debug/11(In7), Word_Multiplexer_2_to_1 DirSel(06)5/4
  Word_08/1 -> Word_Multiplexer_2_to_1 DirSel(06)1/3, Stack Debug/9(In9), Word_Multiplexer_2_to_1 DirSel(06)3/4
  Word_07/1 -> Stack Debug/8(In10), Word_Multiplexer_2_to_1 DirSel(06)/3, Word_Multiplexer_2_to_1 DirSel(06)2/4
  Word_06/1 -> Stack Debug/7(In11), Word_Multiplexer_2_to_1 DirSel(05)/3, Word_Multiplexer_2_to_1 DirSel(06)1/4
  Word_05/1 -> Stack Debug/6(In12), Word_Multiplexer_2_to_1 DirSel(04)/3, Word_Multiplexer_2_to_1 DirSel(06)/4
  Word_04/1 -> Stack Debug/5(In13), Word_Multiplexer_2_to_1 DirSel(03)/3, Word_Multiplexer_2_to_1 DirSel(05)/4
  Word_03/1 -> Stack Debug/4(In14), Word_Multiplexer_2_to_1 DirSel(02)/3, Word_Multiplexer_2_to_1 DirSel(04)/4
  Word_02/1 -> Stack Debug/3(In15), Word_Multiplexer_2_to_1 DirSel(01)/3, Word_Multiplexer_2_to_1 DirSel(03)/4
  Align14/2 -> Or28/1
  Align13/9 -> Or36/2
  Align13/1 -> Or29/2
  Align11/2 -> Or28/4
  Align13/14 -> Or31/2
  Align16/14 -> Or31/3
  Align13/5 -> Or25/2
  Align11/4 -> Or26/4
  Align11/10 -> Or35/4
  Align16/10 -> Or35/3
  Align13/7 -> Or23/2
  Align14/4 -> Or26/1
  Align11/14 -> Or31/4
  Align14/5 -> Or25/1
  Align13/16 -> Or22/2
  Align11/6 -> Or24/4
  Bit_Demux_2/1 -> Enc_2/7
  Bit_Demux_2/2 -> Enc_2/8
  Align16/16 -> Or22/3
  Bit_Demux_4/1 -> Enc_2/1
  Or18/1 -> Bit_Demux_1/2
  Enc_16/1 -> Word_Enable28/6(b03)  "b03"
  Align12/8 -> Enc_16/8
  "]}"/1 -> Or17/14, Align11/14
  ^~/1 -> Or17/15, Align11/15
  _/1 -> Or17/16, Align11/16
  "[{"/1 -> Or17/12, Align11/12
  Align13/15 -> Or30/2
  Gg/1 -> Or21/8, Align16/8
  Align12/6 -> Enc_16/6
  Align11/16 -> Or22/4
  Align13/12 -> Or33/2
  Align14/1 -> Or29/1
  Align14/7 -> Or23/1
  Enc_2/1 -> Word_Enable28/3(b06)  "b06"
  "SelectUpperPage  "/1 -> Word_Enable28/2(b07)  "b07"
  Uu/1 -> Or17/6, Align11/6
  Align12/7 -> Enc_16/7
  Hh/1 -> Or21/9, Align16/9
  Ii/1 -> Or21/10, Align16/10
  Ll/1 -> Or21/13, Align16/13
  Logical Operator30/1 -> Align16/16, Or21/16
  Kk/1 -> Or21/12, Align16/12
  Bit_Demux_1/1 -> Enc_2/5
  Align16/6 -> Or24/3
  Align12/9 -> Enc_16/9
  Enc_16/2 -> Word_Enable28/7(b02)  "b02"
  Enc_2/2 -> Word_Enable28/4(b05)  "b05"
  Align11/3 -> Or27/4
  Align13/10 -> Or35/2
  Pp/1 -> Or17/1, Align11/1
  Ww/1 -> Or17/8, Align11/8
  Align12/14 -> Enc_16/14
  Or35/1 -> Align12/7, IsAnyKeyPressed?/7
  Or36/1 -> Align12/8, IsAnyKeyPressed?/8
  Align14/16 -> Or22/1
  Align16/7 -> Or23/3
  Bit_Demux_3/1 -> Enc_2/2
  Or32/1 -> Align12/4, IsAnyKeyPressed?/4
  Or33/1 -> Align12/5, IsAnyKeyPressed?/5
  Align12/12 -> Enc_16/12
  Align16/3 -> Or27/3
  Or17/1 -> Bit_Demux_4/2
  Ctrl01/1 -> Or19/2, Align14/2
  Ctrl03/1 -> Or19/4, Align14/4
  Ctrl02/1 -> Or19/3, Align14/3
  NULL NULL/1 -> Or19/1, Align14/1
  Ctrl05/1 -> Or19/6, Align14/6
  Or20/1 -> IsAnyKeyPressed?/9, Align12/9
  Zz/1 -> Or17/11, Align11/11
  Mm/1 -> Or21/14, Align16/14
  *:/1 -> Or18/11, Align13/11
  ,</1 -> Or18/13, Align13/13
  (8/1 -> Or18/9, Align13/9
  .>/1 -> Or18/15, Align13/15
  )9/1 -> Or18/10, Align13/10
  "\"/?\""/1 -> Or18/16, Align13/16
  -=/1 -> Or18/14, Align13/14
  Ctrl04/1 -> Or19/5, Align14/5
  Align12/13 -> Enc_16/13
  Align14/12 -> Or33/1
  Or28/1 -> IsAnyKeyPressed?/15, Align12/15
  Align12/15 -> Enc_16/15
  Align11/11 -> Or34/4
  Align13/6 -> Or24/2
  Align11/8 -> Or20/4
  Ctrl07/1 -> Or19/8, Align14/8
  Align14/6 -> Or24/1
  Or26/1 -> IsAnyKeyPressed?/13, Align12/13
  Align11/1 -> Or29/4
  Align16/9 -> Or36/3
  Align11/15 -> Or30/4
  !1/1 -> Or18/2, Align13/2
  #3/1 -> Or18/4, Align13/4
  '7/1 -> Or18/8, Align13/8
  %5/1 -> Or18/6, Align13/6
  Align14/9 -> Or36/1
  Tt/1 -> Or17/5, Align11/5
  Align16/12 -> Or33/3
  Nn/1 -> Or21/15, Align16/15
  "Shift  "/1 -> Bit_Demux_4/1, Bit_Demux_3/1, Bit_Demux_1/1, Bit_Demux_2/1
  Align11/13 -> Or32/3
  Align16/5 -> Or25/3
  Enc_2/3 -> Word_Enable28/5(b04)  "b04"
  Align13/13 -> Or32/2
  Space/0/1 -> Or18/1, Align13/1
  Align12/1 -> Enc_16/1
  Align14/15 -> Or30/1
  undef Left/1 -> Or19/12, Align14/12
  Ctrl14/1 -> Or19/15, Align14/15
  CrRet undef/1 -> Or19/14, Align14/14
  undef Up/1 -> Or19/9, Align14/9
  undef Down/1 -> Or19/10, Align14/10
  LnFeed Right/1 -> Or19/11, Align14/11
  Align14/13 -> Or32/4
  $4/1 -> Or18/5, Align13/5
  Aa/1 -> Or21/2, Align16/2
  Ff/1 -> Or21/7, Align16/7
  &6/1 -> Or18/7, Align13/7
  Align16/1 -> Or29/3
  Ee/1 -> Or21/6, Align16/6
  Bb/1 -> Or21/3, Align16/3
  Align12/10 -> Enc_16/10
  Cc/1 -> Or21/4, Align16/4
  \|/1 -> Or17/13, Align11/13
  Dd/1 -> Or21/5, Align16/5
  Ctrl15/1 -> Or19/16, Align14/16
  Bit_Demux_1/2 -> Enc_2/6
  Xx/1 -> Or17/9, Align11/9
  Bit to Integer Converter5/1 -> To Workspace7/1
  Ctrl12/1 -> Or19/13, Align14/13
  @`/1 -> Or21/1, Align16/1
  Align12/5 -> Enc_16/5
  Align13/8 -> Or20/2
  IsAnyKeyPressed?/1 -> Alignment14/1  "IRQ_Keyboard"
  Align12/3 -> Enc_16/3
  Or23/1 -> IsAnyKeyPressed?/10, Align12/10
  Align11/7 -> Or23/4
  Or34/1 -> Align12/6, IsAnyKeyPressed?/6
  Or22/1 -> Align12/1, IsAnyKeyPressed?/1
  Rr/1 -> Or17/3, Align11/3
  Align11/5 -> Or25/4
  Align11/12 -> Or33/4
  Or19/1 -> Bit_Demux_2/2
  Qq/1 -> Or17/2, Align11/2
  Align16/4 -> Or26/3
  Align12/11 -> Enc_16/11
  Align11/9 -> Or36/4
  Align14/11 -> Or34/1
  Or21/1 -> Bit_Demux_3/2
  +;/1 -> Or18/12, Align13/12
  Ss/1 -> Or17/4, Align11/4
  Align14/10 -> Or35/1
  Align16/13 -> Or32/1
  Or27/1 -> IsAnyKeyPressed?/14, Align12/14
  Align16/11 -> Or34/3
  Align12/2 -> Enc_16/2
  Align13/3 -> Or27/2
  Or25/1 -> IsAnyKeyPressed?/12, Align12/12
  Jj/1 -> Or21/11, Align16/11
  Align13/4 -> Or26/2
  Align13/2 -> Or28/2
  Align14/3 -> Or27/1
  Enc_16/4 -> Word_Enable28/9(b00)  "b00"
  Bit_Demux_3/2 -> Enc_2/4
  Or29/1 -> IsAnyKeyPressed?/16, Align12/16
  Align12/4 -> Enc_16/4
  Align13/11 -> Or34/2
  Align14/8 -> Or20/1
  Or24/1 -> IsAnyKeyPressed?/11, Align12/11
  "\"2"/1 -> Or18/3, Align13/3
  Or30/1 -> Align12/2, IsAnyKeyPressed?/2
  Vv/1 -> Or17/7, Align11/7
  Bit_Demux_4/2 -> Enc_2/3
  Align16/8 -> Or20/3
  Enc_16/3 -> Word_Enable28/8(b01)  "b01"
  Ctrl06/1 -> Or19/7, Align14/7
  Align16/2 -> Or28/3
  Align14/14 -> Or31/1
  Or31/1 -> Align12/3, IsAnyKeyPressed?/3
  Align16/15 -> Or30/3
  Align12/16 -> Enc_16/16
  Yy/1 -> Or17/10, Align11/10
  Format 1: FF|OOO|SSS   CCCCCCCC/4 -> Bus Creator3/21  "SGMT"
  Bit to Integer Converter8/1 -> To Workspace8/1
  Format 2: FF|OOO|DDD   CCCCCCCC/5 -> Bus Creator3/17, Logical Operator21/2  "ADDI"
  Format 1: FF|OOO|SSS   CCCCCCCC/6 -> Bus Creator3/23  "STUI"
  Format 3: FF|OOOOO|R   R|DDD|R|SSS/1 -> Bus Creator3/8  "SHIFT"
  Constant53/1 -> Bus Creator8/6  "b10"
  Constant63/1 -> Bus Creator8/4  "b12"
  Constant50/1 -> Bus Creator8/2  "b14"
  Constant62/1 -> Bus Creator8/11  "b05"
  Constant55/1 -> Bus Creator8/13  "b03"
  Constant56/1 -> Bus Creator8/7  "b09"
  Constant61/1 -> Bus Creator8/3  "b13"
  Constant58/1 -> Bus Creator8/9  "b07"
  Constant57/1 -> Bus Creator8/8  "b08"
  Align9/15 -> Bus Creator4/15, Bus Creator9/15, Bus Creator7/15, Bus Creator6/15
  Align9/14 -> Bus Creator4/14, Bus Creator9/14, Bus Creator7/14, Bus Creator6/14
  Constant59/1 -> Bus Creator8/10  "b06"
  Bit to Integer Converter6/1 -> To Workspace1/1
  Bus Creator7/1 -> Select_Immediate/6, Select_Immediate/7
  Format 1: FF|OOO|SSS   CCCCCCCC/7 -> Bus Creator3/24, Format_1_Unsigned/1, Logical Operator1/1  "STLI"
  Constant54/1 -> Bus Creator8/12  "b04"
  Constant30/1 -> Bus Creator4/10  "b06"
  Constant26/1 -> Bus Creator4/6  "b10"
  Constant33/1 -> Bus Creator4/13  "b03"
  Constant5/1 -> Bus Creator4/3  "b13"
  Format 1: FF|OOO|SSS   CCCCCCCC/2 -> Unknown Instruction/6
  Constant28/1 -> Bus Creator4/8  "b08"
  Constant31/1 -> Bus Creator4/11  "b05"
  Constant13/1 -> Bus Creator4/4  "b12"
  Constant29/1 -> Bus Creator4/9  "b07"
  Constant32/1 -> Bus Creator4/12  "b04"
  Constant46/1 -> Bus Creator5/11  "b05"
  Constant48/1 -> Bus Creator5/13  "b03"
  Constant38/1 -> Bus Creator5/1  "b15"
  Constant40/1 -> Bus Creator5/6  "b10"
  Constant44/1 -> Bus Creator5/10  "b06"
  Constant43/1 -> Bus Creator5/9  "b07"
  Constant42/1 -> Bus Creator5/8  "b08"
  Constant36/1 -> Bus Creator5/3  "b13"
  Name22/1 -> Bus Creator5/15  "b01"
  Name23/1 -> Bus Creator5/16  "b00"
  Bus Creator4/1 -> Select_Src_Reg_Idx/5
  Format 3: FF|OOOOO|R   R|DDD|R|SSS/4 -> Bus Creator3/11  "STL"
  Format 3: FF|OOOOO|R   R|DDD|R|SSS2/4 -> Bus Creator3/3  "LDU"
  Format 2: FF|OOO|DDD   CCCCCCCC/6 -> Bus Creator3/18, Logical Operator20/2  "MOVU"
  Name17/1 -> Bus Creator8/14  "b02"
  Format 3: FF|OOOOO|R   R|DDD|R|SSS/5 -> Bus Creator3/12  "STU"
  Name16/1 -> Bus Creator9/1  "b15"
  Constant35/1 -> Bus Creator5/2  "b14"
  Name11/1 -> Bus Creator9/2  "b14"
  Name29/1 -> Bus Creator9/4  "b12"
  Name28/1 -> Bus Creator9/3  "b13"
  Align9/5 -> Bus Creator9/5, Name29/1, Name28/1, Name11/1, Name16/1, Format 1: FF|OOO|SSS   CCCCCCCC/4, Format 3: FF|OOOOO|R   R|DDD|R|SSS2/2, Format 3: FF|OOOOO|R   R|DDD|R|SSS/2, Format 2: FF|OOO|DDD   CCCCCCCC/4
  Align9/7 -> Name19/1, Bus Creator9/7, Format 3: FF|OOOOO|R   R|DDD|R|SSS2/4, Format 3: FF|OOOOO|R   R|DDD|R|SSS/4
  Format 1: FF|OOO|SSS   CCCCCCCC/3 -> Unknown Instruction/7
  Format 3: FF|OOOOO|R   R|DDD|R|SSS2/7 -> Bus Creator3/6  "POP"
  Align9/12 -> Bus Creator6/12, Bus Creator7/12, Name23/1, Bus Creator9/12
  Constant15/1 -> Bus Creator4/1  "b15"
  Constant1/1 -> Bus Creator4/2  "b14"
  Constant16/1 -> Bus Creator4/5  "b11"
  Constant41/1 -> Bus Creator5/7  "b09"
  Name21/1 -> Bus Creator5/14  "b02"
  Name6/1 -> Bus Creator7/4  "b12"
  Constant47/1 -> Bus Creator5/12  "b04"
  Format 1: FF|OOO|SSS   CCCCCCCC/1 -> Unknown Instruction/5
  Name27/1 -> Bus Creator7/8  "b08"
  Name26/1 -> Bus Creator7/7  "b09"
  Constant52/1 -> Bus Creator8/5  "b11"
  Name25/1 -> Bus Creator7/6  "b10"
  Name1/1 -> Bus Creator7/2  "b14"
  Constant66/1 -> Bus Creator6/5  "b11"
  Constant12/1 -> Bus Creator6/8  "b08"
  Constant64/1 -> Bus Creator6/4  "b12"
  Constant11/1 -> Bus Creator6/7  "b09"
  Constant49/1 -> Bus Creator6/3  "b13"
  Constant51/1 -> Bus Creator8/1  "b15"
  Constant65/1 -> Bus Creator6/1  "b15"
  Format 2: FF|OOO|DDD   CCCCCCCC/4 -> Bus Creator3/16, Logical Operator21/3  "LDUI"
  Format 2: FF|OOO|DDD   CCCCCCCC/8 -> Bus Creator3/20, Logical Operator21/1  "MOVL"
  Logical Operator20/1 -> Format_2_Unsigned/2
  Dec_4_Enbl/2 -> Format 2: FF|OOO|DDD   CCCCCCCC/1, Format_2_Signed/1, Format_2_Unsigned/1, Select_Dest_Reg_Idx/2, Select_Src_Reg_Idx/2
  Format_2_Signed/1 -> Select_Immediate/2
  Dec_4_Enbl/4 -> Select_Immediate/4, Select_Dest_Reg_Idx/4, Select_Src_Reg_Idx/4, Format 0: FF|OO|CCCC   CCCCCCCC/1
  Constant60/1 -> Select_Dest_Reg_Idx/8, Select_Src_Reg_Idx/8
  Format 1: FF|OOO|SSS   CCCCCCCC/8 -> Bus Creator3/25  "CMPI"
  Format 3: FF|OOOOO|R   R|DDD|R|SSS2/5 -> Bus Creator3/4  "CMP"
  Constant34/1 -> Bus Creator6/2  "b14"
  Name5/1 -> Bus Creator7/3  "b13"
  Name8/1 -> Bus Creator8/16  "b00"
  Format 0: FF|OO|CCCC   CCCCCCCC/1 -> Bus Creator3/26  "JLT"
  Format 3: FF|OOOOO|R   R|DDD|R|SSS/8 -> Bus Creator3/15  "MOV"
  Bus Creator8/1 -> Select_Dest_Reg_Idx/7, Select_Dest_Reg_Idx/6, Select_Src_Reg_Idx/7, Select_Src_Reg_Idx/6
  Format 3: FF|OOOOO|R   R|DDD|R|SSS2/3 -> Bus Creator3/2  "LDL"
  Name24/1 -> Bus Creator7/5  "b11"
  Align9/4 -> Format 0: FF|OO|CCCC   CCCCCCCC/3, Format 1: FF|OOO|SSS   CCCCCCCC/3, Logical Operator55/2, not/1, Format 2: FF|OOO|DDD   CCCCCCCC/3
  Format 1: FF|OOO|SSS   CCCCCCCC/5 -> Bus Creator3/22  "SHIFTI"
  Align9/3 -> Logical Operator58/2, Format 0: FF|OO|CCCC   CCCCCCCC/2, Format 1: FF|OOO|SSS   CCCCCCCC/2, Format 2: FF|OOO|DDD   CCCCCCCC/2
  Format 3: FF|OOOOO|R   R|DDD|R|SSS2/2 -> Bus Creator3/1  "AND"
  Align9/10 -> Name21/1, Bus Creator9/10, Bus Creator7/10, Bus Creator6/10
  Constant2/1 -> Bus Creator6/6  "b10"
  Format_2_Unsigned/1 -> Immediate_Unsigned/1
  Bus Creator5/1 -> Select_Dest_Reg_Idx/5
  Name20/1 -> Bus Creator7/1  "b15"
  Format 3: FF|OOOOO|R   R|DDD|R|SSS/7 -> Bus Creator3/14  "NOT"
  Format 0: FF|OO|CCCC   CCCCCCCC/2 -> Bus Creator3/27  "JPE"
  Bit to Integer Converter7/1 -> To Workspace6/1
  Bus Creator6/1 -> Select_Immediate/5
  Bus Creator9/1 -> Select_Immediate/8
  Constant39/1 -> Bus Creator5/5  "b11"
  Align9/9 -> Bus Creator9/9, Bus Creator7/9, Name27/1, Name26/1, Name25/1, Name24/1, Name6/1, Name5/1, Name1/1, Name20/1, Bus Creator6/9
  Format 3: FF|OOOOO|R   R|DDD|R|SSS2/8 -> Bus Creator3/7  "PUSH"
  Format 3: FF|OOOOO|R   R|DDD|R|SSS2/6 -> Bus Creator3/5  "RET"
  Format 0: FF|OO|CCCC   CCCCCCCC/4 -> Bus Creator3/29  "JMP"
  Align9/8 -> Name8/1, Bus Creator9/8
  Format 3: FF|OOOOO|R   R|DDD|R|SSS/2 -> Bus Creator3/9  "ADD"
  Bit to Integer Converter4/1 -> To Workspace5/1
  Align7/1 -> Align9/1
  Dec_4_Enbl/1 -> Logical Operator56/1, Logical Operator58/1, Select_Dest_Reg_Idx/1, Select_Src_Reg_Idx/1, Logical Operator55/1
  Align7/2 -> Align9/2
  Logical Operator21/1 -> Format_2_Signed/2
  Constant27/1 -> Bus Creator4/7  "b09"
  Format 3: FF|OOOOO|R   R|DDD|R|SSS2/1 -> Unknown Instruction/1
  Name19/1 -> Bus Creator8/15  "b01"
  Format 2: FF|OOO|DDD   CCCCCCCC/2 -> Unknown Instruction/3
  Align9/6 -> Name17/1, Bus Creator9/6, Format 3: FF|OOOOO|R   R|DDD|R|SSS2/3, Format 3: FF|OOOOO|R   R|DDD|R|SSS/3
  Align9/16 -> Bus Creator4/16, Bus Creator9/16, Bus Creator7/16, Bus Creator6/16
  Format 2: FF|OOO|DDD   CCCCCCCC/3 -> Unknown Instruction/4
  Align9/11 -> Name22/1, Bus Creator9/11, Bus Creator7/11, Bus Creator6/11
  Format 2: FF|OOO|DDD   CCCCCCCC/1 -> Unknown Instruction/2
  Align9/13 -> Bus Creator9/13, Bus Creator7/13, Bus Creator6/13
  ? -> Bit to Integer Converter6/1
  Format 2: FF|OOO|DDD   CCCCCCCC/7 -> Bus Creator3/19, Logical Operator20/1  "LDLI"
  Constant37/1 -> Bus Creator5/4  "b12"
  Format 0: FF|OO|CCCC   CCCCCCCC/3 -> Bus Creator3/28  "CALL"
  Dec_4_Enbl/3 -> Format_1_Signed/2, Format_1_Unsigned/2, Select_Dest_Reg_Idx/3, Select_Src_Reg_Idx/3, Format 1: FF|OOO|SSS   CCCCCCCC/1
  Instruction_SHIFT/1(Data_Out(2B)) -> Word_Enable6/2
  Instruction_LDU/1(Data(2B)) -> Word_Enable9/2
  Instruction_LDL/1(Data(2B)) -> Word_Enable10/2
  Instruction_STU/1(DataOut(2B)) -> Word_Enable7/2
  Instruction_STL/1(DataOut(2B)) -> Word_Enable8/2
  Instruction_OR/1(A||B(2B)) -> Word_Enable3/2
  Instruction_XOR/1 -> Word_Enable2/2
  Instruction_MOVU/1(Data(2B)) -> Word_Enable5/2
  Instruction_AND/1(A.B(2B)) -> Word_Enable4/2
  Instruction_NOT/1 -> Word_Enable/2
  Instruction_ADD/1 -> Word_Enable1/2
  Instruction_CMP/1 -> GreaterThan(1b)2/1
  Instruction_CMP/2 -> Align74/2  "(uint) A<B"
  Instruction_CMP/3 -> GreaterThan(1b)1/1
  Word_Mux_2/2 -> Instruction_NOT/1, Instruction_XOR/1, Instruction_OR/1(A(2B)), Instruction_AND/1(A(2B)), Instruction_ADD/1, Instruction_MOVU/2(Data_0(2B)), Instruction_SHIFT/1(Data_In(2B)), Instruction_STU/1(Data(2B)), Instruction_STL/1(Data(2B)), Instruction_LDU/1(Data_0(2B)), Instruction_LDL/1(Data_1(2B)), Instruction_CMP/1
  Word_Mux_3/2 -> Instruction_XOR/2, Instruction_OR/2(B(2B)), Instruction_AND/2(B(2B)), Instruction_ADD/2, Instruction_MOVU/1(Data_1(2B)), Instruction_SHIFT/2(Count(2B)), Instruction_LDU/2(Data_1(2B)), Instruction_LDL/2(Data_0(2B)), Instruction_CMP/2
  Instruction_CMP/4 -> Align74/3  "(int) A<B"
  Instruction_CMP/5 -> Align74/4  "A=B"
  Logical Operator37/1 -> Word_Enable10/1
  Logical Operator28/1 -> Word_Enable9/1
  Logical Operator25/1 -> Word_Enable8/1
  Logical Operator5/1 -> Word_Enable7/1
  Logical Operator6/1 -> Word_Enable6/1
  Logical Operator8/1 -> Word_Enable1/1
  Instruction_ADD/2 -> Align74/1  "Overflow"
  Word_Enable8/1 -> Merge16_Simulated/9
  Constant6/1 -> Merge16_Simulated/12, Merge16_Simulated/13, Merge16_Simulated/14, Merge16_Simulated/15, Merge16_Simulated/16
  Word_Enable5/1 -> Merge16_Simulated/6
  Word_Enable/1 -> Merge16_Simulated/1
  Word_Enable1/1 -> Merge16_Simulated/5
  Word_Enable10/1 -> Merge16_Simulated/11
  Word_Enable4/1 -> Merge16_Simulated/4
  Word_Enable2/1 -> Merge16_Simulated/2
  Word_Enable7/1 -> Merge16_Simulated/8
  Word_Enable3/1 -> Merge16_Simulated/3
  Word_Enable9/1 -> Merge16_Simulated/10
  Align76/1 -> Align77/1
  Bus Selector28/16 -> Align81/8, Align78/16  "<b00>"
  Bus Selector2/3 -> Word_Enable/1, Logical Operator7/11  "<NOT>"
  Logical Operator12/1 -> Word_Mux_3/3
  Bus Selector2/6 -> Word_Enable4/1, Logical Operator7/8, Logical Operator12/3  "<AND>"
  Bus Selector2/2 -> Logical Operator12/6, Logical Operator7/12  "<CMP>"
  Logical Operator19/1 -> Word_Mux_2/3
  Bus Selector2/13 -> Logical Operator5/2, Logical Operator19/3  "<STU>"
  Bus Creator28/1 -> Word_Mux_3/6  "DataMem"
  Logical Operator23/1 -> Word_Mux_3/4
  Constant18/1 -> Word_Mux_2/1, Word_Mux_2/2, Word_Mux_3/1
  Logical Operator13/1 -> Word_Mux_3/2
  Bus Selector2/15 -> Logical Operator25/2, Logical Operator19/1  "<STL>"
  Bus Selector2/19 -> Logical Operator13/1, Logical Operator37/2, Logical Operator7/1  "<LDL>"
  Bus Selector2/11 -> Logical Operator6/2, Logical Operator19/5, Logical Operator23/1  "<SHIFTI>"
  Bus Selector2/12 -> Logical Operator5/1, Logical Operator19/4  "<STUI>"
  Bus Selector2/8 -> Logical Operator8/2, Logical Operator7/6, Logical Operator12/2  "<ADD>"
  Bus Selector2/9 -> Word_Enable5/1, Logical Operator19/6, Logical Operator23/2  "<MOVU>"
  Bus Selector2/10 -> Logical Operator6/1, Logical Operator7/5, Logical Operator12/1  "<SHIFT>"
  Constant19/1 -> Word_Mux_2/5, Word_Mux_3/5, Word_Mux_2/6
  Bus Selector2/18 -> Logical Operator13/2, Logical Operator37/1, Logical Operator7/2  "<LDLI>"
  Bus Selector2/7 -> Logical Operator8/1, Logical Operator7/7, Logical Operator23/3  "<ADDI>"
  Bus Selector2/17 -> Logical Operator13/3, Logical Operator28/2, Logical Operator7/3  "<LDU>"
  Logical Operator7/1 -> Word_Mux_2/4
  Bus Selector2/4 -> Word_Enable2/1, Logical Operator7/10, Logical Operator12/5  "<XOR>"
  Bus Selector2/5 -> Word_Enable3/1, Logical Operator7/9, Logical Operator12/4  "<OR>"
  Bus Creator25/1 -> Word_Mux_2/8  "DestRegVal"
  Bus Selector2/14 -> Logical Operator25/1, Logical Operator19/2  "<STLI>"
  Bus Selector2/1 -> Logical Operator23/4, Logical Operator19/7  "<CMPI>"
  Bus Selector2/16 -> Logical Operator28/1, Logical Operator7/4, Logical Operator13/4  "<LDUI>"
  Dec_1/3 -> Word_Enable22/1, General_Purpose_Register_5/1
  Word_Mux_7/2 -> General_Purpose_Register_7/3, General_Purpose_Register_6/3, General_Purpose_Register_5/3, General_Purpose_Register_4/3, General_Purpose_Register_3/3, General_Purpose_Register_2/3, General_Purpose_Register_1/3, General_Purpose_Register_0/3
  Dec_1/1 -> Word_Enable24/1, General_Purpose_Register_7/1
  Dec_1/4 -> Word_Enable21/1, General_Purpose_Register_4/1
  Dec_1/2 -> Word_Enable23/1, General_Purpose_Register_6/1
  Logical Operator10/1 -> General_Purpose_Register_6/2, General_Purpose_Register_5/2, General_Purpose_Register_4/2, General_Purpose_Register_3/2, General_Purpose_Register_2/2, General_Purpose_Register_1/2, General_Purpose_Register_0/2, General_Purpose_Register_7/2
  Dec_1/6 -> Word_Enable19/1, General_Purpose_Register_2/1
  Dec_1/7 -> Word_Enable17/1, General_Purpose_Register_1/1
  Dec_1/5 -> Word_Enable20/1, General_Purpose_Register_3/1
  Dec_1/8 -> Word_Enable16/1, General_Purpose_Register_0/1
  Dec_8/1 -> Word_Enable15/1
  Dec_8/2 -> Word_Enable14/1
  Dec_8/3 -> Word_Enable13/1
  Dec_8/4 -> Word_Enable12/1
  Dec_8/5 -> Word_Enable11/1
  Dec_8/6 -> Word_Enable18/1
  Dec_8/7 -> Word_Enable26/1
  Dec_8/8 -> Word_Enable25/1
  Align84/2 -> Dec_1/2
  Align84/1 -> Dec_1/1
  Align83/3 -> Dec_8/3
  Align83/1 -> Dec_8/1
  Align84/3 -> Dec_1/3
  Align83/2 -> Dec_8/2
  General_Purpose_Register_7/1 -> Word_Enable15/2, Word_Enable24/2, Register Debug/8(In1)
  General_Purpose_Register_6/1 -> Word_Enable14/2, Word_Enable23/2, Register Debug/7(In2)
  General_Purpose_Register_5/1 -> Word_Enable13/2, Word_Enable22/2, Register Debug/6(In3)
  General_Purpose_Register_4/1 -> Word_Enable12/2, Word_Enable21/2, Register Debug/5(In4)
  General_Purpose_Register_3/1 -> Word_Enable11/2, Word_Enable20/2, Register Debug/4(In5)
  General_Purpose_Register_2/1 -> Word_Enable18/2, Word_Enable19/2, Register Debug/3(In6)
  General_Purpose_Register_0/1 -> Word_Enable25/2, Word_Enable16/2, Register Debug/1(In8)
  Word_Enable24/1 -> Merge8_Simulated1/1
  Word_Enable23/1 -> Merge8_Simulated1/2
  Word_Enable22/1 -> Merge8_Simulated1/3
  Word_Enable21/1 -> Merge8_Simulated1/4
  Word_Enable20/1 -> Merge8_Simulated1/5
  Word_Enable19/1 -> Merge8_Simulated1/6
  Word_Enable17/1 -> Merge8_Simulated1/7
  Word_Enable16/1 -> Merge8_Simulated1/8
  Word_Enable15/1 -> Merge8_Simulated/1
  Word_Enable14/1 -> Merge8_Simulated/2
  Word_Enable13/1 -> Merge8_Simulated/3
  Word_Enable12/1 -> Merge8_Simulated/4
  Word_Enable11/1 -> Merge8_Simulated/5
  Word_Enable18/1 -> Merge8_Simulated/6
  Word_Enable26/1 -> Merge8_Simulated/7
  Word_Enable25/1 -> Merge8_Simulated/8
  General_Purpose_Register_1/1 -> Word_Enable26/2, Word_Enable17/2, Register Debug/2(In7)
  Status_Register/1(Data(2B)) -> Bus Selector17/1  "Status_Register"
  Bus Selector/16 -> Logical Operator10/16, Word_Mux_7/2  "<MOV>"
  ADD ADDI MOVU SHIFT/1 -> Word_Mux_7/1
  Bus Selector/18 -> Logical Operator22/2  "<CMP>"
  Bus Selector/17 -> Segment_Register/3(Write(1b)), Segment_Register/2(Select(1b))  "<SGMT>"
  Logical Operator22/1 -> Status_Register/2(Sel_CMP_or_CMPI(1b))
  Bus Selector/14 -> Word_Mux_7/4, Logical Operator10/14  "<MOVL>"
  Bus Selector/5 -> Logical Operator10/5, ADD ADDI MOVU SHIFT/5  "<AND>"
  Bus Selector/15 -> Word_Mux_7/3, Logical Operator10/15  "<POP>"
  Bus Selector/12 -> Logical Operator10/12, ADD ADDI MOVU SHIFT/12  "<NOT>"
  Bus Selector/2 -> Logical Operator10/2, ADD ADDI MOVU SHIFT/2  "<XOR>"
  Bus Selector/10 -> ADD ADDI MOVU SHIFT/10, Logical Operator10/10  "<LDUI>"
  Select_Immediate/2 -> Bus Selector27/1, Bit to Integer Converter8/1
  Bus Selector/7 -> ADD ADDI MOVU SHIFT/7, Logical Operator10/7  "<ADDI>"
  Bus Selector/13 -> ADD ADDI MOVU SHIFT/13, Logical Operator10/13  "<SHIFT>"
  Bus Selector/19 -> Logical Operator22/1  "<CMPI>"
  Bus Selector/3 -> ADD ADDI MOVU SHIFT/3, Logical Operator10/3  "<LDLI>"
  Bus Selector/11 -> Logical Operator10/11, ADD ADDI MOVU SHIFT/11  "<LDU>"
  Bus Selector/9 -> Logical Operator10/9, ADD ADDI MOVU SHIFT/9  "<SHIFTI>"
  Merge8_Simulated/1 -> Word_Mux_7/6, Bus Selector13/1
  Bus Selector/1 -> ADD ADDI MOVU SHIFT/1, Logical Operator10/1  "<LDL>"
  Bus Selector/4 -> Logical Operator10/4, ADD ADDI MOVU SHIFT/4  "<OR>"
  Bus Selector/6 -> Logical Operator10/6, ADD ADDI MOVU SHIFT/6  "<ADD>"
  Bus Selector/8 -> Logical Operator10/8, ADD ADDI MOVU SHIFT/8  "<MOVU>"
  Word_15/1 -> Bus Selector9/1, Word_Multiplexer_2_to_1 DirSel(06)8/3, Stack Debug/16(In2)  "Stack"
  Word_Enable6/1 -> Merge16_Simulated/7
  Mux_1/2 -> Alignment26/1
  Constant69/1 -> Mux_4/1
  Bus Selector8/5 -> Word_Mux_5/2, Word_Mux_4/2  "<CALL>"
  Constant70/1 -> uint_to_bus1/1
  logic/1 -> Entering_IRQ_Handler... (1 clock cycle)/1
  Set/1 -> Bit_Mux_2/3
  Reset/1 -> Bit_Mux_2/4
  IRQ_Active/1 -> logic/2
  IRQ_Handler_Active/1 -> logic/1, "Exiting_IRQ_Handler... (1 clock cycle) "/2
  Entering_IRQ_Handler... (1 clock cycle)/1 -> Alignment4/1, Bit_Mux_2/1, Logical Operator44/2
  "Exiting_IRQ_Handler... (1 clock cycle) "/1 -> Logical Operator47/2, Bit_Mux_2(1)/2, Bit_Mux_2/2, Logical Operator51/1, Logical Operator50/1, Logical Operator49/1, Logical Operator44/1
  Logical Operator18/1 -> Program_Counter/1, Logical Operator27/1
  Mux_4/2 -> Program_Counter/3
  Run/1 -> Counter_Control/1
  Mode/1 -> Counter_Control/2
  Dec_8_Enbl/6 -> Logical Operator45/1  "CmdReset"
  Counter_Control/1 -> Alignment17/1  "IRQ_Timer"
  Dec_8_Enbl/5 -> Mode/1  "CmdMode"
  Word_Mux_1/2 -> Counter_Control/4
  StartVal/1 -> Word_Mux_1/4
  Counter_Control/4 -> Counter_16bit/3
  Counter_Control/2 -> Counter_16bit/1
  Align23/16 -> Align22/16, Align42/16
  Dec_8_Enbl/7 -> StartVal/2, StartVal/1, Logical Operator46/1, Word_Mux_1/1, Logical Operator45/2  "CmdSetStartVal"
  Align23/15 -> Align22/15, Align42/15
  <0xFFF8..0xFFFD>1/1(Sel(1b)) -> Dec_8_Enbl/1, Word_Enable29/1(Sel(1b))
  Dec_8_Enbl/8 -> StopVal/2, StopVal/1  "CmdSetStopVal"
  Align23/14 -> Align22/14, Align42/14
  Dec_8_Enbl/4 -> Run/1  "CmdRun"
  Logical Operator45/1 -> Counter_Control/3
  Counter_Control/3 -> Counter_16bit/2
  StopVal/1 -> Counter_Control/5
  Counter_16bit/1 -> Counter_Control/6, Bus Selector25/1, Bus Selector16/1
  Bus Selector15/1 -> Mode/2, Run/2  "<b00>"
  Logical Operator46/1 -> Word_Mux_1/2
  Immediate_Unsigned/1 -> Select_Immediate/1
  Format_1_Unsigned/1 -> Immediate_Unsigned/2
  Logical Operator1/1 -> Format_1_Signed/1
  Format_1_Signed/1 -> Select_Immediate/3
  Bit to Integer Converter15/1 -> To Workspace16/1
  Logical Operator27/1 -> Program_Counter/2
  Delay/1 -> uint_to_bus2/1
  Constant73/1 -> uint_to_bus3/1
  uint_to_bus3/1 -> Word_Mux_4(6)/5
  Constant75/1 -> Word_Mux_4(6)/1
  Constant76/1 -> Logical Operator30/2
  Oo/1 -> Logical Operator30/1
  OneShot/1 -> Counter_Control(1)/2
  uint_to_bus2/1 -> Counter_Control(1)/5
  Counter_Control(1)/2 -> Counter_16bit(1)/1
  Counter_Control(1)/3 -> Counter_16bit(1)/2
  Counter_Control(1)/4 -> Counter_16bit(1)/3
  StartValue/1 -> uint_to_bus4/1
  uint_to_bus4/1 -> Counter_Control(1)/4
  Counter_16bit(1)/1 -> Counter_Control(1)/6
  "  Reset"/1 -> Counter_Control(1)/3
  Counter_Control(1)/1 -> Bit_Mux_2(1)/1, Logical Operator47/1
  " Run"/1 -> Bit_Mux_2(1)/4
  " Halt"/1 -> Bit_Mux_2(1)/3
  Run/Halt/1 -> Counter_Control(1)/1, Block keyboard interrupt when the interrupt delay counter is running/1
  Logical Operator62/1 -> IRQ_Active/1
  IRQ_Timer_Latch/1 -> Priority_Selector/2
  Logical Operator40/1 -> Priority_Selector_1/2, Logical Operator57/1
  IRQ_UART_Latch/1 -> Priority_Selector/3
  Clock/1 -> Align47/3, CPU/1, Alignment25/1
  Logical Operator42/1 -> Priority_Selector_3/2, Logical Operator61/1
  IRQ_FPU_Latch/1 -> Priority_Selector/4
  Priority_Selector/1 -> Mux_1/1, Logical Operator62/4
  Priority_Selector/2 -> Mux_1/2, Logical Operator49/2, Logical Operator62/3
  Priority_Selector/3 -> Mux_1/3, Logical Operator50/2, Logical Operator62/2
  Constant71/1 -> uint_to_bus5/1
  Constant67/1 -> uint_to_bus/1
  uint_to_bus/1 -> Mux_1/5
  uint_to_bus5/1 -> Mux_1/6
  Constant68/1 -> uint_to_bus6/1
  Constant74/1 -> uint_to_bus7/1
  uint_to_bus6/1 -> Mux_1/7
  uint_to_bus7/1 -> Mux_1/8
  Constant77/1 -> Mux_4/5
  Priority_Selector/4 -> Mux_1/4, Logical Operator51/2, Logical Operator62/1
  Logical Operator44/1 -> IRQ_Handler_Active/1
  Bit_Mux_2/1 -> IRQ_Handler_Active/2
  Bit_Mux_2(1)/1 -> Run/Halt/2
  Logical Operator47/1 -> Run/Halt/1
  Logical Operator61/1 -> IRQ_FPU_Latch/1
  Logical Operator57/1 -> IRQ_UART_Latch/1
  Bit_Mux_3/1 -> IRQ_FPU_Latch/2
  Logical Operator53/1 -> IRQ_Timer_Latch/1
  Alignment1/1 -> "Exiting_IRQ_Handler... (1 clock cycle) "/1
  Bus Creator3/1 -> Bus Selector5/1, Bus Selector3/1, Bus Selector8/1, Bus Selector/1, Bus Selector7/1, Bus Selector2/1
  IRQ_UART/1 -> Logical Operator40/2
  Logical Operator39/1 -> Priority_Selector_2/2, Logical Operator53/1
  <0xFFF7..0xFFF7>/1(Sel(1b)) -> Logical Operator41/1, Logical Operator29/1, Word_Enable36/1(Sel(1b))
  Logical Operator29/1 -> Logical Operator41/2
  Logical Operator48/1 -> Priority_Selector/1
  Bit_Mux_4/1 -> IRQ_UART_Latch/2
  Bit_Mux_1/1 -> IRQ_Timer_Latch/2
  Logical Operator49/1 -> Logical Operator53/2, Priority_Selector_2/1
  Logical Operator51/1 -> Logical Operator61/2, Priority_Selector_3/1
  Logical Operator50/1 -> Logical Operator57/2, Priority_Selector_1/1
  Enable_IRQ_UART/1 -> Logical Operator40/1, Word_Enable36/8(b01)  "b01"
  Enable_IRQ_FPU/1 -> Logical Operator42/1, Word_Enable36/9(b00)  "b00"
  Constant89/1 -> Word_Enable36/4(b05)  "b05"
  Constant88/1 -> Word_Enable36/3(b06)  "b06"
  Constant87/1 -> Word_Enable36/2(b07)  "b07"
  Constant90/1 -> Word_Enable36/5(b04)  "b04"
  Enable_IRQ_Timer/1 -> Logical Operator39/1, Word_Enable36/7(b02)  "b02"
  Enable_IRQ_Keyboard/1 -> Logical Operator48/1, Word_Enable36/6(b03)  "b03"
  Align41/5 -> Enable_IRQ_Keyboard/2
  Align41/6 -> Enable_IRQ_Timer/2
  Align41/7 -> Enable_IRQ_UART/2
  Align41/8 -> Enable_IRQ_FPU/2
  Logical Operator41/1 -> Enable_IRQ_Keyboard/1, Enable_IRQ_Timer/1, Enable_IRQ_UART/1, Enable_IRQ_FPU/1
  Alignment/1 -> Logical Operator48/2  "IRQ_Keyboard"
  Alignment2/1 -> Logical Operator39/2
  If IRQ is enabled then disable all instructions for one clock cycle to allow program counter to jump to a IRQ handler./1 -> Dec_4_Enbl/1
  IRQ_FPU/1 -> Logical Operator42/2
  Priority_Selector_3/2 -> Bit_Mux_3/2
  Priority_Selector_3/1 -> Bit_Mux_3/1
  " Set"/1 -> Bit_Mux_4/4, Bit_Mux_3/4, Bit_Mux_1/4
  Priority_Selector_2/1 -> Bit_Mux_1/1
  " Reset"/1 -> Bit_Mux_4/3, Bit_Mux_3/3, Bit_Mux_1/3
  Priority_Selector_2/2 -> Bit_Mux_1/2
  Priority_Selector_1/1 -> Bit_Mux_4/1
  Priority_Selector_1/2 -> Bit_Mux_4/2
  Block keyboard interrupt when the interrupt delay counter is running/1 -> Logical Operator48/3
  Alignment4/1 -> If IRQ is enabled then disable all instructions for one clock cycle to allow program counter to jump to a IRQ handler./1, Alignment24/1, Word_Mux_4(6)/4, Logical Operator36/1  "IRQ"
  Alignment5/1 -> IRQ_Handler_Active/3, IRQ_Timer_Latch/3, IRQ_UART_Latch/3, IRQ_FPU_Latch/3, Counter_Control(1)/7, Counter_16bit(1)/4, Run/Halt/3, Enable_IRQ_FPU/3, Enable_IRQ_UART/3, Enable_IRQ_Timer/3, Enable_IRQ_Keyboard/3
  Logical Operator17/1 -> Align46/3, "Select_Data  "/1
  Constant3/1 -> "Select_Data  "/3
  Logical Operator14/1 -> Logical Operator52/2
  Logical Operator54/1 -> Terminator22/1
  Bus Creator27/1 -> Terminator21/1  "DataMem"
  Constant72/1 -> Logical Operator52/1
  Format 3: FF|OOOOO|R   R|DDD|R|SSS/6 -> Bus Creator3/13  "XOR"
  Format 3: FF|OOOOO|R   R|DDD|R|SSS/3 -> Bus Creator3/10  "OR"
  not2/1 -> Format 3: FF|OOOOO|R   R|DDD|R|SSS/1
  not1/1 -> Format 3: FF|OOOOO|R   R|DDD|R|SSS2/1
  Logical Operator55/1 -> not1/1
  Logical Operator56/1 -> not2/1
  not/1 -> Logical Operator56/2
  not3/1 -> Unknown Instruction/8
  Unknown Instruction/1 -> To Workspace2/1
  Logical Operator58/1 -> not3/1
  Mux_1/1 -> Terminator3/1
  Mux_4/1 -> Terminator5/1
  Select_Address/1 -> Terminator6/1
  "Select_Data  "/1 -> Terminator7/1
  Select_Dest_Reg_Idx/1 -> Terminator8/1
  Select_Src_Reg_Idx/1 -> Terminator9/1
  Select_Immediate/1 -> Terminator10/1
  Word_Multiplexer_2_to_1 DirSel(00)/1 -> Terminator11/1
  Word_Multiplexer_2_to_1 DirSel(01)/1 -> Terminator12/1
  Word_Multiplexer_2_to_1 DirSel(02)/1 -> Terminator13/1
  Word_Multiplexer_2_to_1 DirSel(03)/1 -> Terminator14/1
  Word_Multiplexer_2_to_1 DirSel(04)/1 -> Terminator15/1
  Word_Multiplexer_2_to_1 DirSel(05)/1 -> Terminator16/1
  Word_Multiplexer_2_to_1 DirSel(06)/1 -> Terminator17/1
  Word_Multiplexer_2_to_1 DirSel(06)1/1 -> Terminator18/1
  Word_Multiplexer_2_to_1 DirSel(06)2/1 -> Terminator19/1
  Word_Multiplexer_2_to_1 DirSel(06)3/1 -> Terminator20/1
  Word_Multiplexer_2_to_1 DirSel(06)4/1 -> Terminator23/1
  Word_Multiplexer_2_to_1 DirSel(06)5/1 -> Terminator24/1
  Word_Multiplexer_2_to_1 DirSel(06)6/1 -> Terminator25/1
  Word_Multiplexer_2_to_1 DirSel(06)7/1 -> Terminator26/1
  Word_Multiplexer_2_to_1 DirSel(06)8/1 -> Terminator27/1
  Word_Multiplexer_2_to_1 DirSel(06)9/1 -> Terminator28/1
  Word_Mux_4(6)/1 -> Terminator29/1
  Word_Mux_1/1 -> Terminator30/1
  Word_Mux_2/1 -> Terminator31/1
  Word_Mux_3/1 -> Terminator32/1
  Word_Mux_4/1 -> Terminator33/1
  Word_Mux_5/1 -> Terminator34/1
  Word_Mux_7/1 -> Terminator35/1
  Alignment10/1 -> Status_TxBufferReady (will go to status register)/1  "Status_TxBufferReady"
  Logical Operator70/1 -> MATLAB Function/1(UartWrite)
  Shift_Register (Higher_Byte)/2 -> Bus Selector22/1
  Dec_16/15 -> Bit_Mux_16/15
  Shift_Register (Lower_Byte)/1 -> Shift_Register (Higher_Byte)/2, Majority_Selector (2_out_of_3)/3(C(1b))
  " Halt6"/1 -> Shift_Register (Higher_Byte)/1
  Tx_Active_Latch (BlockTransmissionWhenIdle)/1 -> Logical Operator71/1
  Memory2/1 -> RxStateMachine/3
  Constant91/1 -> RxStateMachine/1
  Tx_State_Machine/1 -> Logical Operator70/1, Bit_Mux_2(1)2/2, Logical Operator68/1
  (UartRxPin)/1 -> uint_to_bus(byte)5/1
  Clear_RxBufferReady/1 -> Logical Operator73/2
  "  Idle"/1 -> Bit_Mux_16_Nand/20
  Logical Operator73/1 -> Bit_Mux_2(1)1/2, Logical Operator64/2
  RxStates/14 -> Logical Operator59/7  "Data7"
  RxStates/8 -> Logical Operator59/1  "Data1"
  "  Run"/1 -> Bit_Mux_2(1)2/3
  Logical Operator68/1 -> Tx_Active_Latch (BlockTransmissionWhenIdle)/1
  Tx_State_Machine/2 -> Bus Selector23/1
  Bus Selector23/2 -> Dec_16/2  "<b02>"
  Bit_Mux_16/1 -> Shift_Register3/2, Scope/1
  uint_to_bus(byte)2/1 -> Tx_State_Machine/2
  bus_to_uint(word)/1 -> Bus Selector6/1
  " Halt7"/1 -> Rx_Buffer/1
  Bit_Mux_2(1)1/1 -> Rx_Buffer_Ready/2
  Rx_Buffer_Ready/1 -> Alignment9/1
  Logical Operator63/1 -> Memory2/1
  RxStates/9 -> Logical Operator59/2  "Data2"
  Logical Operator72/1 -> StopBitNotDetected (GoToError)/2
  Constant93/1 -> Logical Operator65/2
  Bus Selector21/3 -> RxStates/3  "<b1>"
  StartBitDetected (GoToStart)/1 -> Logical Operator63/4
  StopBitDetected (GoToStop)/1 -> Logical Operator63/3
  DataBitDetected (GoToNextState)/1 -> Logical Operator63/1
  RxStateMachine/2 -> Bus Selector21/1
  CLK2/1 -> Logical Operator65/1, MATLAB Function1/2(CLK), StopBitDetected (GoToStop)/1, StartBitNotDetected (GoToIdle)/1, DataBitDetected (GoToNextState)/1, StopBitNotDetected (GoToError)/1, Rx_Buffer_Ready/3, Logical Operator60/2, StartBitDetected (GoToStart)/1  "CLK(Baudrate)"
  RxStates/12 -> Logical Operator59/5  "Data5"
  Bus Selector21/4 -> RxStates/4  "<b0>"
  Alignment12/1 -> ErrorStopBitNotDetected/1  "Error_StopBitNotDetected"
  RxStates/1 -> Terminator37/1
  RxStates/6 -> StartBitNotDetected (GoToIdle)/3, Logical Operator64/1, Bit_Mux_2(1)1/1, Logical Operator67/2  "Stop"
  RxStates/5 -> Terminator41/1
  RxStates/3 -> Terminator39/1
  RxStates/2 -> Terminator38/1
  RxStates/15 -> Logical Operator73/1, Logical Operator59/8  "Start"
  Shift_Register3/1 -> Terminator36/1
  Dec_16/3 -> Bit_Mux_16/3
  " StopBit"/1 -> Bit_Mux_16/22
  NotUsed0/1 -> Bit_Mux_16_Nand/5, Bit_Mux_16_Nand/6, Bit_Mux_16_Nand/7, Bit_Mux_16_Nand/8, Bit_Mux_16_Nand/9
  "  Halt"/1 -> Bit_Mux_2(1)2/4
  Dec_16/2 -> Bit_Mux_16/2
  " Halt9"/1 -> uint_to_bus(word)4/1
  Dec_16/9 -> Bit_Mux_16/9, "For simulation, use only data bits. Real-world implementation will use whole frame."/3
  FreqDivider/2 -> Terminator46/1
  Logical Operator71/1 -> Tx_State_Machine/1
  " StartBit"/1 -> Bit_Mux_16/31
  RxStates/11 -> Logical Operator59/4  "Data4"
  Bus Selector23/3 -> Dec_16/3  "<b01>"
  Constant83/1 -> uint_to_bus(byte)4/1
  Shift_Register (Lower_Byte)/2 -> Terminator45/1
  bus_to_uint(byte)/1 -> MATLAB Function/2(UartDataTx)
  uint_to_bus(word)4/1 -> Shift_Register3/3
  " Halt8"/1 -> uint_to_bus(word)3/1
  Serial/1 -> Shift_Register3/1
  " Halt1"/1 -> Bit_Mux_2(1)1/4
  Logical Operator69/1 -> Shift_Register3/4
  uint_to_bus(byte)4/1 -> FreqDivider/2
  " Halt4"/1 -> FreqDivider/1
  Constant92/1 -> uint_to_bus(byte)2/1
  " Halt3"/1 -> uint_to_bus(word)1/1
  uint_to_bus(word)2/1 -> Shift_Register (Higher_Byte)/3
  Dec_16/14 -> "For simulation, use only data bits. Real-world implementation will use whole frame."/8, Bit_Mux_16/14
  Dec_16/5 -> Bit_Mux_16/5
  Dec_16/16 -> Bit_Mux_16/16, Alignment10/1
  RxStates/4 -> Terminator40/1
  Dec_16/7 -> Bit_Mux_16/7, "For simulation, use only data bits. Real-world implementation will use whole frame."/1
  Dec_16/13 -> "For simulation, use only data bits. Real-world implementation will use whole frame."/7, Bit_Mux_16/13
  Dec_16/12 -> "For simulation, use only data bits. Real-world implementation will use whole frame."/6, Bit_Mux_16/12
  Bit_Mux_16_Nand/1 -> Shift_Register (Lower_Byte)/2
  Bus Selector23/4 -> Dec_16/4  "<b00>"
  Dec_16/10 -> "For simulation, use only data bits. Real-world implementation will use whole frame."/4, Bit_Mux_16/10
  RxStates/16 -> Logical Operator67/1  "Idle"
  uint_to_bus(word)3/1 -> Rx_Buffer/3
  <0xFFF6..0xFFF6>/1(Sel(1b)) -> Alignment6/1
  Logical Operator64/1 -> Rx_Buffer_Ready/1
  " Halt2"/1 -> uint_to_bus(word)2/1
  Dec_16/11 -> "For simulation, use only data bits. Real-world implementation will use whole frame."/5, Bit_Mux_16/11
  Bit_Mux_2(1)2/1 -> Tx_Active_Latch (BlockTransmissionWhenIdle)/2
  Rx_Buffer/1 -> Terminator43/1
  Constant45/1 -> uint_to_bus(byte)1/1
  Logical Operator66/1 -> StartBitDetected (GoToStart)/2
  Alignment9/1 -> IRQ_UART_RX (toStatusRegister...)/1  "Status_RxBufferReady"
  Dec_16/1 -> Bit_Mux_16/1
  Tx_Output_Buffer/1 -> Bus Selector19/1
  Bus Selector19/8 -> Bit_Mux_16/30  "<b07>"
  RxStates/13 -> Logical Operator59/6  "Data6"
  uint_to_bus(byte)6/1 -> "Rx_State_Machine "/2
  Bus Selector19/4 -> Bit_Mux_16/26  "<b03>"
  Bus Selector20/4 -> Bit_Mux_16_Nand/14  "<b3>"
  Bus Selector22/2 -> Majority_Selector (2_out_of_3)/2(A(1b))  "<b00>"
  RxStates/7 -> StopBitDetected (GoToStop)/3, StopBitNotDetected (GoToError)/3  "Data0"
  Bus Selector20/7 -> Bit_Mux_16_Nand/17  "<b6>"
  Dec_16/6 -> Bit_Mux_16/6
  StartBit/1 -> Bit_Mux_16_Nand/19
  Bus Selector20/5 -> Bit_Mux_16_Nand/15  "<b4>"
  Bus Selector20/2 -> Bit_Mux_16_Nand/12  "<b1>"
  Bus Selector21/1 -> RxStates/1  "<b3>"
  StartBitNotDetected (GoToIdle)/1 -> Logical Operator63/2
  Bus Selector19/3 -> Bit_Mux_16/25  "<b02>"
  " Halt10"/1 -> "Rx_State_Machine "/1
  Logical Operator59/1 -> DataBitDetected (GoToNextState)/2, Logical Operator60/1
  RxStates/10 -> Logical Operator59/3  "Data3"
  Dec_16/8 -> "For simulation, use only data bits. Real-world implementation will use whole frame."/2, Bit_Mux_16/8
  uint_to_bus(word)1/1 -> Shift_Register (Lower_Byte)/3
  Constant94/1 -> uint_to_bus(byte)6/1
  Bus Selector20/8 -> Bit_Mux_16_Nand/18  "<b7>"
  uint_to_bus(byte)5/1 -> Bus Selector20/1
  Bus Selector19/7 -> Bit_Mux_16/29  "<b06>"
  RxStateMachine/1 -> Terminator44/1
  FreqDivider/1 -> SamplingFinished(16x)/1
  Bus Selector20/6 -> Bit_Mux_16_Nand/16  "<b5>"
  "Rx_State_Machine "/2 -> Bus Selector24/1
  Bus Selector24/1 -> Bit_Mux_16_Nand/1  "<b3>"
  uint_to_bus(byte)1/1 -> RxStateMachine/2
  Majority_Selector (2_out_of_3)/1(D(1b)) -> Rx_Buffer/2, Logical Operator66/1, StopBitDetected (GoToStop)/2, StartBitNotDetected (GoToIdle)/2, Logical Operator72/1
  Shift_Register3/2 -> bus_to_uint(byte)/1
  Logical Operator65/1 -> "Rx_State_Machine "/3
  Bus Selector24/3 -> Bit_Mux_16_Nand/3  "<b1>"
  Alignment11/1 -> bus_to_uint(word)/1  "Data"
  Dec_16/4 -> Bit_Mux_16/4
  StopBitNotDetected (GoToError)/1 -> Alignment12/1
  StopBit/1 -> Bit_Mux_16_Nand/10
  Bus Selector20/1 -> Bit_Mux_16_Nand/11  "<b0>"
  Bus Selector22/1 -> Majority_Selector (2_out_of_3)/1(B(1b))  "<b01>"
  Alignment6/1 -> Tx_Output_Buffer/3, Tx_Output_Buffer/2, Tx_Output_Buffer/1, Logical Operator68/2, Bit_Mux_2(1)2/1  "Write"
  Bus Selector19/2 -> Bit_Mux_16/24  "<b01>"
  Bus Selector23/1 -> Dec_16/1  "<b03>"
  Rx_Buffer/2 -> Alignment11/1
  Bus Selector24/2 -> Bit_Mux_16_Nand/2  "<b2>"
  Logical Operator60/1 -> Rx_Buffer/4
  " Idle"/1 -> Bit_Mux_16/32
  SamplingFinished(16x)/1 -> Align47/2
  Bus Selector19/6 -> Bit_Mux_16/28  "<b05>"
  NotUsed1/1 -> Bit_Mux_16/17, Bit_Mux_16/18, Bit_Mux_16/21, Bit_Mux_16/20, Bit_Mux_16/19
  Alignment7/1 -> Tx_Output_Buffer/4  "Data"
  "For simulation, use only data bits. Real-world implementation will use whole frame."/1 -> Logical Operator69/1
  CLK/1 -> Logical Operator70/2, Logical Operator69/2, Tx_State_Machine/3, Tx_Active_Latch (BlockTransmissionWhenIdle)/3  "CLK(Baudrate)"
  Bus Selector20/3 -> Bit_Mux_16_Nand/13  "<b2>"
  Shift_Register (Higher_Byte)/1 -> Terminator42/1
  Bus Selector24/4 -> Bit_Mux_16_Nand/4  "<b0>"
  Bus Selector19/5 -> Bit_Mux_16/27  "<b04>"
  Logical Operator67/1 -> StartBitDetected (GoToStart)/3
  Serial_Port_Sampling_Freq/1 -> BaudRate/1, Align47/1, FreqDivider/3
  Bus Selector21/2 -> RxStates/2  "<b2>"
  " Halt5"/1 -> Shift_Register (Lower_Byte)/1
  "Rx_State_Machine "/1 -> MATLAB Function1/1(Reset)
  " Run1"/1 -> Bit_Mux_2(1)1/3
  CLK1/1 -> Shift_Register (Lower_Byte)/4, Shift_Register (Higher_Byte)/4  "CLK(Sampling)"
  Bus Selector19/1 -> Bit_Mux_16/23  "<b00>"
  CLK3/1 -> Tx_Output_Buffer/5  "CLK(CPU)"
  Logical Operator74/1 -> Status_Register1/2(Write(1b)1), Word_Mux_6/1
  Word_Mux_6/2 -> Status_Register1/3(Status(2B))
  CMP_or_CMPI/1 -> Logical Operator74/1
  ADD_or_ADDI/1 -> Logical Operator74/2
  StatusFromALU/1 -> Word_Mux_6/3
  STS/1 -> Word_Mux_6/2
  FromImmediate/1 -> Word_Mux_6/4
  Align61/12 -> Align6/1
  Align61/11 -> Align6/2
  Align61/10 -> Align6/3
  Align61/9 -> Align6/4
  Align61/8 -> Align6/5
  Align61/7 -> Align6/6
  Instruction_ROM (0x000 .. 0xFFF)/2(b14) -> Align7/2
  Instruction_ROM (0x000 .. 0xFFF)/3(b13) -> Align7/3
  Instruction_ROM (0x000 .. 0xFFF)/4(b12) -> Align7/4
  Instruction_ROM (0x000 .. 0xFFF)/5(b11) -> Align7/5
  Instruction_ROM (0x000 .. 0xFFF)/6(b10) -> Align7/6
  Instruction_ROM (0x000 .. 0xFFF)/16(b00) -> Align7/16
  Instruction_ROM (0x000 .. 0xFFF)/15(b01) -> Align7/15
  Instruction_ROM (0x000 .. 0xFFF)/14(b02) -> Align7/14
  Instruction_ROM (0x000 .. 0xFFF)/13(b03) -> Align7/13
  Instruction_ROM (0x000 .. 0xFFF)/12(b04) -> Align7/12
  Instruction_ROM (0x000 .. 0xFFF)/11(b05) -> Align7/11
  Instruction_ROM (0x000 .. 0xFFF)/10(b06) -> Align7/10
  Instruction_ROM (0x000 .. 0xFFF)/9(b07) -> Align7/9
  Instruction_ROM (0x000 .. 0xFFF)/8(b08) -> Align7/8
  Instruction_ROM (0x000 .. 0xFFF)/7(b09) -> Align7/7
  Instruction_ROM (0x000 .. 0xFFF)/1(b15) -> Align7/1
  Alignment8/1 -> Dec_4_Enbl/2
  Alignment13/1 -> Dec_4_Enbl/3
  Alignment14/1 -> Alignment/1
  Dec_32_Enbl12/1 -> Data_ROM (0x000 .. 0xFFF)/1(Y63)
  Dec_32_Enbl12/2 -> Data_ROM (0x000 .. 0xFFF)/2(Y62)
  Dec_32_Enbl12/3 -> Data_ROM (0x000 .. 0xFFF)/3(Y61)
  Dec_32_Enbl12/4 -> Data_ROM (0x000 .. 0xFFF)/4(Y60)
  Dec_32_Enbl12/5 -> Data_ROM (0x000 .. 0xFFF)/5(Y59)
  Dec_32_Enbl12/6 -> Data_ROM (0x000 .. 0xFFF)/6(Y58)
  Dec_32_Enbl12/7 -> Data_ROM (0x000 .. 0xFFF)/7(Y57)
  Dec_32_Enbl12/8 -> Data_ROM (0x000 .. 0xFFF)/8(Y56)
  Dec_32_Enbl12/9 -> Data_ROM (0x000 .. 0xFFF)/9(Y55)
  Dec_32_Enbl12/10 -> Data_ROM (0x000 .. 0xFFF)/10(Y54)
  Dec_32_Enbl12/11 -> Data_ROM (0x000 .. 0xFFF)/11(Y53)
  Dec_32_Enbl12/12 -> Data_ROM (0x000 .. 0xFFF)/12(Y52)
  Dec_32_Enbl12/13 -> Data_ROM (0x000 .. 0xFFF)/13(Y51)
  Dec_32_Enbl12/14 -> Data_ROM (0x000 .. 0xFFF)/14(Y50)
  Dec_32_Enbl12/15 -> Data_ROM (0x000 .. 0xFFF)/15(Y49)
  Dec_32_Enbl12/16 -> Data_ROM (0x000 .. 0xFFF)/16(Y48)
  Dec_32_Enbl12/17 -> Data_ROM (0x000 .. 0xFFF)/17(Y47)
  Dec_32_Enbl12/18 -> Data_ROM (0x000 .. 0xFFF)/18(Y46)
  Dec_32_Enbl12/19 -> Data_ROM (0x000 .. 0xFFF)/19(Y45)
  Dec_32_Enbl12/20 -> Data_ROM (0x000 .. 0xFFF)/20(Y44)
  Dec_32_Enbl12/21 -> Data_ROM (0x000 .. 0xFFF)/21(Y43)
  Dec_32_Enbl12/22 -> Data_ROM (0x000 .. 0xFFF)/22(Y42)
  Dec_32_Enbl12/23 -> Data_ROM (0x000 .. 0xFFF)/23(Y41)
  Dec_32_Enbl12/24 -> Data_ROM (0x000 .. 0xFFF)/24(Y40)
  Dec_32_Enbl12/25 -> Data_ROM (0x000 .. 0xFFF)/25(Y39)
  Dec_32_Enbl12/26 -> Data_ROM (0x000 .. 0xFFF)/26(Y38)
  Dec_32_Enbl12/27 -> Data_ROM (0x000 .. 0xFFF)/27(Y37)
  Dec_32_Enbl12/28 -> Data_ROM (0x000 .. 0xFFF)/28(Y36)
  Dec_32_Enbl12/29 -> Data_ROM (0x000 .. 0xFFF)/29(Y35)
  Dec_32_Enbl12/30 -> Data_ROM (0x000 .. 0xFFF)/30(Y34)
  Dec_32_Enbl12/31 -> Data_ROM (0x000 .. 0xFFF)/31(Y33)
  Dec_32_Enbl12/32 -> Data_ROM (0x000 .. 0xFFF)/32(Y32)
  Dec_32_Enbl11/1 -> Data_ROM (0x000 .. 0xFFF)/33(Y31)
  Dec_32_Enbl11/2 -> Data_ROM (0x000 .. 0xFFF)/34(Y30)
  Dec_32_Enbl11/3 -> Data_ROM (0x000 .. 0xFFF)/35(Y29)
  Dec_32_Enbl11/4 -> Data_ROM (0x000 .. 0xFFF)/36(Y28)
  Dec_32_Enbl11/5 -> Data_ROM (0x000 .. 0xFFF)/37(Y27)
  Dec_32_Enbl11/6 -> Data_ROM (0x000 .. 0xFFF)/38(Y26)
  Dec_32_Enbl11/7 -> Data_ROM (0x000 .. 0xFFF)/39(Y25)
  Dec_32_Enbl11/8 -> Data_ROM (0x000 .. 0xFFF)/40(Y24)
  Dec_32_Enbl11/9 -> Data_ROM (0x000 .. 0xFFF)/41(Y23)
  Dec_32_Enbl11/10 -> Data_ROM (0x000 .. 0xFFF)/42(Y22)
  Dec_32_Enbl11/11 -> Data_ROM (0x000 .. 0xFFF)/43(Y21)
  Dec_32_Enbl11/12 -> Data_ROM (0x000 .. 0xFFF)/44(Y20)
  Dec_32_Enbl11/13 -> Data_ROM (0x000 .. 0xFFF)/45(Y19)
  Dec_32_Enbl11/14 -> Data_ROM (0x000 .. 0xFFF)/46(Y18)
  Dec_32_Enbl11/15 -> Data_ROM (0x000 .. 0xFFF)/47(Y17)
  Dec_32_Enbl11/16 -> Data_ROM (0x000 .. 0xFFF)/48(Y16)
  Dec_32_Enbl11/17 -> Data_ROM (0x000 .. 0xFFF)/49(Y15)
  Dec_32_Enbl11/18 -> Data_ROM (0x000 .. 0xFFF)/50(Y14)
  Dec_32_Enbl11/19 -> Data_ROM (0x000 .. 0xFFF)/51(Y13)
  Dec_32_Enbl11/20 -> Data_ROM (0x000 .. 0xFFF)/52(Y12)
  Dec_32_Enbl11/21 -> Data_ROM (0x000 .. 0xFFF)/53(Y11)
  Dec_32_Enbl11/22 -> Data_ROM (0x000 .. 0xFFF)/54(Y10)
  Dec_32_Enbl11/23 -> Data_ROM (0x000 .. 0xFFF)/55(Y09)
  Dec_32_Enbl11/24 -> Data_ROM (0x000 .. 0xFFF)/56(Y08)
  Dec_32_Enbl11/25 -> Data_ROM (0x000 .. 0xFFF)/57(Y07)
  Dec_32_Enbl11/26 -> Data_ROM (0x000 .. 0xFFF)/58(Y06)
  Dec_32_Enbl11/27 -> Data_ROM (0x000 .. 0xFFF)/59(Y05)
  Dec_32_Enbl11/28 -> Data_ROM (0x000 .. 0xFFF)/60(Y04)
  Dec_32_Enbl11/29 -> Data_ROM (0x000 .. 0xFFF)/61(Y03)
  Dec_32_Enbl11/30 -> Data_ROM (0x000 .. 0xFFF)/62(Y02)
  Dec_32_Enbl11/31 -> Data_ROM (0x000 .. 0xFFF)/63(Y01)
  Dec_32_Enbl11/32 -> Data_ROM (0x000 .. 0xFFF)/64(Y00)
  Dec_32_Enbl9/1 -> Data_ROM (0x000 .. 0xFFF)/65(X63)
  Dec_32_Enbl9/2 -> Data_ROM (0x000 .. 0xFFF)/66(X62)
  Dec_32_Enbl9/3 -> Data_ROM (0x000 .. 0xFFF)/67(X61)
  Dec_32_Enbl9/4 -> Data_ROM (0x000 .. 0xFFF)/68(X60)
  Dec_32_Enbl9/5 -> Data_ROM (0x000 .. 0xFFF)/69(X59)
  Dec_32_Enbl9/6 -> Data_ROM (0x000 .. 0xFFF)/70(X58)
  Dec_32_Enbl9/7 -> Data_ROM (0x000 .. 0xFFF)/71(X57)
  Dec_32_Enbl9/8 -> Data_ROM (0x000 .. 0xFFF)/72(X56)
  Dec_32_Enbl9/9 -> Data_ROM (0x000 .. 0xFFF)/73(X55)
  Dec_32_Enbl9/10 -> Data_ROM (0x000 .. 0xFFF)/74(X54)
  Dec_32_Enbl9/11 -> Data_ROM (0x000 .. 0xFFF)/75(X53)
  Dec_32_Enbl9/12 -> Data_ROM (0x000 .. 0xFFF)/76(X52)
  Dec_32_Enbl9/13 -> Data_ROM (0x000 .. 0xFFF)/77(X51)
  Dec_32_Enbl9/14 -> Data_ROM (0x000 .. 0xFFF)/78(X50)
  Dec_32_Enbl9/15 -> Data_ROM (0x000 .. 0xFFF)/79(X49)
  Dec_32_Enbl9/16 -> Data_ROM (0x000 .. 0xFFF)/80(X48)
  Dec_32_Enbl9/17 -> Data_ROM (0x000 .. 0xFFF)/81(X47)
  Dec_32_Enbl9/18 -> Data_ROM (0x000 .. 0xFFF)/82(X46)
  Dec_32_Enbl9/19 -> Data_ROM (0x000 .. 0xFFF)/83(X45)
  Dec_32_Enbl9/20 -> Data_ROM (0x000 .. 0xFFF)/84(X44)
  Dec_32_Enbl9/21 -> Data_ROM (0x000 .. 0xFFF)/85(X43)
  Dec_32_Enbl9/22 -> Data_ROM (0x000 .. 0xFFF)/86(X42)
  Dec_32_Enbl9/23 -> Data_ROM (0x000 .. 0xFFF)/87(X41)
  Dec_32_Enbl9/24 -> Data_ROM (0x000 .. 0xFFF)/88(X40)
  Dec_32_Enbl9/25 -> Data_ROM (0x000 .. 0xFFF)/89(X39)
  Dec_32_Enbl9/26 -> Data_ROM (0x000 .. 0xFFF)/90(X38)
  Dec_32_Enbl9/27 -> Data_ROM (0x000 .. 0xFFF)/91(X37)
  Dec_32_Enbl9/28 -> Data_ROM (0x000 .. 0xFFF)/92(X36)
  Dec_32_Enbl9/29 -> Data_ROM (0x000 .. 0xFFF)/93(X35)
  Dec_32_Enbl9/30 -> Data_ROM (0x000 .. 0xFFF)/94(X34)
  Dec_32_Enbl9/31 -> Data_ROM (0x000 .. 0xFFF)/95(X33)
  Dec_32_Enbl9/32 -> Data_ROM (0x000 .. 0xFFF)/96(X32)
  Dec_32_Enbl1/32 -> Data_ROM (0x000 .. 0xFFF)/128(X00)
  Dec_32_Enbl1/31 -> Data_ROM (0x000 .. 0xFFF)/127(X01)
  Dec_32_Enbl1/30 -> Data_ROM (0x000 .. 0xFFF)/126(X02)
  Dec_32_Enbl1/29 -> Data_ROM (0x000 .. 0xFFF)/125(X03)
  Dec_32_Enbl1/28 -> Data_ROM (0x000 .. 0xFFF)/124(X04)
  Dec_32_Enbl1/27 -> Data_ROM (0x000 .. 0xFFF)/123(X05)
  Dec_32_Enbl1/26 -> Data_ROM (0x000 .. 0xFFF)/122(X06)
  Dec_32_Enbl1/25 -> Data_ROM (0x000 .. 0xFFF)/121(X07)
  Dec_32_Enbl1/24 -> Data_ROM (0x000 .. 0xFFF)/120(X08)
  Dec_32_Enbl1/23 -> Data_ROM (0x000 .. 0xFFF)/119(X09)
  Dec_32_Enbl1/22 -> Data_ROM (0x000 .. 0xFFF)/118(X10)
  Dec_32_Enbl1/21 -> Data_ROM (0x000 .. 0xFFF)/117(X11)
  Dec_32_Enbl1/20 -> Data_ROM (0x000 .. 0xFFF)/116(X12)
  Dec_32_Enbl1/19 -> Data_ROM (0x000 .. 0xFFF)/115(X13)
  Dec_32_Enbl1/18 -> Data_ROM (0x000 .. 0xFFF)/114(X14)
  Dec_32_Enbl1/17 -> Data_ROM (0x000 .. 0xFFF)/113(X15)
  Dec_32_Enbl1/16 -> Data_ROM (0x000 .. 0xFFF)/112(X16)
  Dec_32_Enbl1/15 -> Data_ROM (0x000 .. 0xFFF)/111(X17)
  Dec_32_Enbl1/14 -> Data_ROM (0x000 .. 0xFFF)/110(X18)
  Dec_32_Enbl1/13 -> Data_ROM (0x000 .. 0xFFF)/109(X19)
  Dec_32_Enbl1/12 -> Data_ROM (0x000 .. 0xFFF)/108(X20)
  Dec_32_Enbl1/11 -> Data_ROM (0x000 .. 0xFFF)/107(X21)
  Dec_32_Enbl1/10 -> Data_ROM (0x000 .. 0xFFF)/106(X22)
  Dec_32_Enbl1/9 -> Data_ROM (0x000 .. 0xFFF)/105(X23)
  Dec_32_Enbl1/8 -> Data_ROM (0x000 .. 0xFFF)/104(X24)
  Dec_32_Enbl1/7 -> Data_ROM (0x000 .. 0xFFF)/103(X25)
  Dec_32_Enbl1/6 -> Data_ROM (0x000 .. 0xFFF)/102(X26)
  Dec_32_Enbl1/5 -> Data_ROM (0x000 .. 0xFFF)/101(X27)
  Dec_32_Enbl1/4 -> Data_ROM (0x000 .. 0xFFF)/100(X28)
  Dec_32_Enbl1/3 -> Data_ROM (0x000 .. 0xFFF)/99(X29)
  Dec_32_Enbl1/2 -> Data_ROM (0x000 .. 0xFFF)/98(X30)
  Dec_32_Enbl1/1 -> Data_ROM (0x000 .. 0xFFF)/97(X31)
  Align10/15 -> <0x0000..0x0FFF>/15(b01), Align2/2
  Align2/6 -> Dec_32_Enbl12/1, Logical Operator75/1
  Align10/16 -> Align2/1, <0x0000..0x0FFF>/16(b00)
  Align10/12 -> <0x0000..0x0FFF>/12(b04), Align2/5
  Align2/2 -> Dec_32_Enbl12/5, Dec_32_Enbl11/5
  Align10/10 -> <0x0000..0x0FFF>/10(b06), Dec_32_Enbl1/6, Dec_32_Enbl9/6
  Align10/7 -> Dec_32_Enbl9/3, <0x0000..0x0FFF>/7(b09), Dec_32_Enbl1/3
  Align10/9 -> Dec_32_Enbl9/5, <0x0000..0x0FFF>/9(b07), Dec_32_Enbl1/5
  Align2/3 -> Dec_32_Enbl12/4, Dec_32_Enbl11/4
  Align10/14 -> <0x0000..0x0FFF>/14(b02), Align2/3
  Align10/6 -> <0x0000..0x0FFF>/6(b10), Dec_32_Enbl1/2, Dec_32_Enbl9/2
  Align10/11 -> <0x0000..0x0FFF>/11(b05), Align2/6
  Align10/8 -> Dec_32_Enbl9/4, <0x0000..0x0FFF>/8(b08), Dec_32_Enbl1/4
  Align2/1 -> Dec_32_Enbl12/6, Dec_32_Enbl11/6
  Align2/4 -> Dec_32_Enbl12/3, Dec_32_Enbl11/3
  Align10/5 -> <0x0000..0x0FFF>/5(b11), Logical Operator76/1, Dec_32_Enbl9/1
  Align10/13 -> <0x0000..0x0FFF>/13(b03), Align2/4
  Align2/5 -> Dec_32_Enbl11/2, Dec_32_Enbl12/2
  Logical Operator76/1 -> Dec_32_Enbl1/1
  Logical Operator75/1 -> Dec_32_Enbl11/1
  Dec_32_Enbl14/22 -> Video_RAM (0x000 .. 0x3FF)/54(X10)
  Dec_32_Enbl14/8 -> Video_RAM (0x000 .. 0x3FF)/40(X24)
  Dec_32_Enbl14/25 -> Video_RAM (0x000 .. 0x3FF)/57(X07)
  Align32/3 -> Dec_32_Enbl15/4
  Dec_32_Enbl14/19 -> Video_RAM (0x000 .. 0x3FF)/51(X13)
  Dec_32_Enbl14/18 -> Video_RAM (0x000 .. 0x3FF)/50(X14)
  Dec_32_Enbl14/29 -> Video_RAM (0x000 .. 0x3FF)/61(X03)
  Dec_32_Enbl14/9 -> Video_RAM (0x000 .. 0x3FF)/41(X23)
  Dec_32_Enbl14/7 -> Video_RAM (0x000 .. 0x3FF)/39(X25)
  Dec_32_Enbl14/1 -> Video_RAM (0x000 .. 0x3FF)/33(X31)
  Dec_32_Enbl14/14 -> Video_RAM (0x000 .. 0x3FF)/46(X18)
  Dec_32_Enbl14/23 -> Video_RAM (0x000 .. 0x3FF)/55(X09)
  Dec_32_Enbl14/10 -> Video_RAM (0x000 .. 0x3FF)/42(X22)
  Dec_32_Enbl14/4 -> Video_RAM (0x000 .. 0x3FF)/36(X28)
  Dec_32_Enbl14/5 -> Video_RAM (0x000 .. 0x3FF)/37(X27)
  Dec_32_Enbl14/11 -> Video_RAM (0x000 .. 0x3FF)/43(X21)
  Dec_32_Enbl14/12 -> Video_RAM (0x000 .. 0x3FF)/44(X20)
  Dec_32_Enbl14/15 -> Video_RAM (0x000 .. 0x3FF)/47(X17)
  Dec_32_Enbl14/13 -> Video_RAM (0x000 .. 0x3FF)/45(X19)
  Dec_32_Enbl14/6 -> Video_RAM (0x000 .. 0x3FF)/38(X26)
  Dec_32_Enbl14/2 -> Video_RAM (0x000 .. 0x3FF)/34(X30)
  Dec_32_Enbl14/20 -> Video_RAM (0x000 .. 0x3FF)/52(X12)
  Dec_32_Enbl14/21 -> Video_RAM (0x000 .. 0x3FF)/53(X11)
  Dec_32_Enbl14/17 -> Video_RAM (0x000 .. 0x3FF)/49(X15)
  Dec_32_Enbl14/28 -> Video_RAM (0x000 .. 0x3FF)/60(X04)
  Dec_32_Enbl14/26 -> Video_RAM (0x000 .. 0x3FF)/58(X06)
  Dec_32_Enbl14/31 -> Video_RAM (0x000 .. 0x3FF)/63(X01)
  Dec_32_Enbl14/27 -> Video_RAM (0x000 .. 0x3FF)/59(X05)
  Dec_32_Enbl14/30 -> Video_RAM (0x000 .. 0x3FF)/62(X02)
  Dec_32_Enbl14/16 -> Video_RAM (0x000 .. 0x3FF)/48(X16)
  Dec_32_Enbl14/24 -> Video_RAM (0x000 .. 0x3FF)/56(X08)
  Dec_32_Enbl14/32 -> Video_RAM (0x000 .. 0x3FF)/64(X00)
  Dec_32_Enbl15/24 -> Video_RAM (0x000 .. 0x3FF)/24(Y08)
  Dec_32_Enbl15/31 -> Video_RAM (0x000 .. 0x3FF)/31(Y01)
  Dec_32_Enbl15/9 -> Video_RAM (0x000 .. 0x3FF)/9(Y23)
  Dec_32_Enbl15/4 -> Video_RAM (0x000 .. 0x3FF)/4(Y28)
  Dec_32_Enbl15/26 -> Video_RAM (0x000 .. 0x3FF)/26(Y06)
  Dec_32_Enbl15/17 -> Video_RAM (0x000 .. 0x3FF)/17(Y15)
  Dec_32_Enbl15/3 -> Video_RAM (0x000 .. 0x3FF)/3(Y29)
  Dec_32_Enbl15/16 -> Video_RAM (0x000 .. 0x3FF)/16(Y16)
  Dec_32_Enbl15/14 -> Video_RAM (0x000 .. 0x3FF)/14(Y18)
  Dec_32_Enbl15/2 -> Video_RAM (0x000 .. 0x3FF)/2(Y30)
  Dec_32_Enbl15/22 -> Video_RAM (0x000 .. 0x3FF)/22(Y10)
  Dec_32_Enbl15/7 -> Video_RAM (0x000 .. 0x3FF)/7(Y25)
  Dec_32_Enbl15/28 -> Video_RAM (0x000 .. 0x3FF)/28(Y04)
  Dec_32_Enbl15/25 -> Video_RAM (0x000 .. 0x3FF)/25(Y07)
  Dec_32_Enbl15/11 -> Video_RAM (0x000 .. 0x3FF)/11(Y21)
  Dec_32_Enbl15/5 -> Video_RAM (0x000 .. 0x3FF)/5(Y27)
  Dec_32_Enbl15/1 -> Video_RAM (0x000 .. 0x3FF)/1(Y31)
  Dec_32_Enbl15/19 -> Video_RAM (0x000 .. 0x3FF)/19(Y13)
  Dec_32_Enbl15/23 -> Video_RAM (0x000 .. 0x3FF)/23(Y09)
  Dec_32_Enbl15/8 -> Video_RAM (0x000 .. 0x3FF)/8(Y24)
  Dec_32_Enbl15/15 -> Video_RAM (0x000 .. 0x3FF)/15(Y17)
  Dec_32_Enbl15/27 -> Video_RAM (0x000 .. 0x3FF)/27(Y05)
  Dec_32_Enbl15/12 -> Video_RAM (0x000 .. 0x3FF)/12(Y20)
  Dec_32_Enbl15/18 -> Video_RAM (0x000 .. 0x3FF)/18(Y14)
  Dec_32_Enbl15/10 -> Video_RAM (0x000 .. 0x3FF)/10(Y22)
  Dec_32_Enbl15/13 -> Video_RAM (0x000 .. 0x3FF)/13(Y19)
  Align32/2 -> Dec_32_Enbl15/5
  Align32/4 -> Dec_32_Enbl15/3
  Dec_32_Enbl15/20 -> Video_RAM (0x000 .. 0x3FF)/20(Y12)
  Dec_32_Enbl15/30 -> Video_RAM (0x000 .. 0x3FF)/30(Y02)
  Dec_32_Enbl15/6 -> Video_RAM (0x000 .. 0x3FF)/6(Y26)
  Dec_32_Enbl15/21 -> Video_RAM (0x000 .. 0x3FF)/21(Y11)
  Align32/1 -> Dec_32_Enbl15/6
  Dec_32_Enbl14/3 -> Video_RAM (0x000 .. 0x3FF)/35(X29)
  Dec_32_Enbl15/32 -> Video_RAM (0x000 .. 0x3FF)/32(Y00)
  Dec_32_Enbl15/29 -> Video_RAM (0x000 .. 0x3FF)/29(Y03)
  Align32/5 -> Dec_32_Enbl15/2
  Align9/1 -> Alignment8/1
  Align9/2 -> Alignment13/1
  Align7/16 -> Align9/16
  Align7/15 -> Align9/15
  Align7/14 -> Align9/14
  Align7/13 -> Align9/13
  Align7/11 -> Align9/11
  Align7/12 -> Align9/12
  Align7/10 -> Align9/10
  Align7/9 -> Align9/9
  Align7/8 -> Align9/8
  Align7/7 -> Align9/7
  Align7/6 -> Align9/6
  Align7/5 -> Align9/5
  Align7/4 -> Align9/4
  Align7/3 -> Align9/3
  Word_Enable30/1("b07 ") -> Merge2_8b_Simulated1/9
  Word_Enable30/2("b06 ") -> Merge2_8b_Simulated1/10
  Word_Enable30/3("b05 ") -> Merge2_8b_Simulated1/11
  Word_Enable30/4("b04 ") -> Merge2_8b_Simulated1/12
  Word_Enable30/5("b03 ") -> Merge2_8b_Simulated1/13
  Word_Enable30/6("b02 ") -> Merge2_8b_Simulated1/14
  Word_Enable30/8("b00 ") -> Merge2_8b_Simulated1/16
  <0x0000..0x0FFF>/1(Sel(1b)) -> Word_Enable30/1(Sel(1b))
  Align10/4 -> <0x0000..0x0FFF>/4(b12)
  Align10/3 -> <0x0000..0x0FFF>/3(b13)
  Align10/2 -> <0x0000..0x0FFF>/2(b14)
  Align10/1 -> <0x0000..0x0FFF>/1(b15)
  Align18/11 -> <0x1000..0x1FFF>/11(b05), Align15/6
  Align18/9 -> Dec_32_Enbl18/5, <0x1000..0x1FFF>/9(b07), Dec_32_Enbl13/5
  Align18/13 -> <0x1000..0x1FFF>/13(b03), Align15/4
  Align18/15 -> <0x1000..0x1FFF>/15(b01), Align15/2
  Align18/5 -> Dec_32_Enbl18/1, <0x1000..0x1FFF>/5(b11), Logical Operator78/1
  Align18/4 -> <0x1000..0x1FFF>/4(b12)
  Dec_32_Enbl18/23 -> Data_RAM (0x000 .. 0xFFF)/87(X41)
  Dec_32_Enbl18/25 -> Data_RAM (0x000 .. 0xFFF)/89(X39)
  Dec_32_Enbl18/24 -> Data_RAM (0x000 .. 0xFFF)/88(X40)
  Dec_32_Enbl18/2 -> Data_RAM (0x000 .. 0xFFF)/66(X62)
  Dec_32_Enbl18/14 -> Data_RAM (0x000 .. 0xFFF)/78(X50)
  Align18/14 -> Align15/3, <0x1000..0x1FFF>/14(b02)
  Dec_32_Enbl16/27 -> Data_RAM (0x000 .. 0xFFF)/59(Y05)
  Dec_32_Enbl13/19 -> Data_RAM (0x000 .. 0xFFF)/115(X13)
  Dec_32_Enbl17/4 -> Data_RAM (0x000 .. 0xFFF)/4(Y60)
  Align18/8 -> Dec_32_Enbl18/4, <0x1000..0x1FFF>/8(b08), Dec_32_Enbl13/4
  Align18/3 -> <0x1000..0x1FFF>/3(b13)
  Dec_32_Enbl13/15 -> Data_RAM (0x000 .. 0xFFF)/111(X17)
  Dec_32_Enbl13/7 -> Data_RAM (0x000 .. 0xFFF)/103(X25)
  Dec_32_Enbl17/30 -> Data_RAM (0x000 .. 0xFFF)/30(Y34)
  Dec_32_Enbl17/29 -> Data_RAM (0x000 .. 0xFFF)/29(Y35)
  Dec_32_Enbl17/23 -> Data_RAM (0x000 .. 0xFFF)/23(Y41)
  Dec_32_Enbl17/17 -> Data_RAM (0x000 .. 0xFFF)/17(Y47)
  Dec_32_Enbl17/18 -> Data_RAM (0x000 .. 0xFFF)/18(Y46)
  Dec_32_Enbl17/16 -> Data_RAM (0x000 .. 0xFFF)/16(Y48)
  Dec_32_Enbl13/14 -> Data_RAM (0x000 .. 0xFFF)/110(X18)
  Dec_32_Enbl17/19 -> Data_RAM (0x000 .. 0xFFF)/19(Y45)
  Dec_32_Enbl13/26 -> Data_RAM (0x000 .. 0xFFF)/122(X06)
  Dec_32_Enbl17/14 -> Data_RAM (0x000 .. 0xFFF)/14(Y50)
  Dec_32_Enbl16/4 -> Data_RAM (0x000 .. 0xFFF)/36(Y28)
  Dec_32_Enbl16/13 -> Data_RAM (0x000 .. 0xFFF)/45(Y19)
  Align15/3 -> Dec_32_Enbl17/4, Dec_32_Enbl16/4
  Dec_32_Enbl13/1 -> Data_RAM (0x000 .. 0xFFF)/97(X31)
  Dec_32_Enbl18/29 -> Data_RAM (0x000 .. 0xFFF)/93(X35)
  Dec_32_Enbl13/27 -> Data_RAM (0x000 .. 0xFFF)/123(X05)
  Dec_32_Enbl13/30 -> Data_RAM (0x000 .. 0xFFF)/126(X02)
  Dec_32_Enbl18/28 -> Data_RAM (0x000 .. 0xFFF)/92(X36)
  Dec_32_Enbl18/17 -> Data_RAM (0x000 .. 0xFFF)/81(X47)
  Dec_32_Enbl18/26 -> Data_RAM (0x000 .. 0xFFF)/90(X38)
  Dec_32_Enbl18/9 -> Data_RAM (0x000 .. 0xFFF)/73(X55)
  Dec_32_Enbl13/28 -> Data_RAM (0x000 .. 0xFFF)/124(X03)
  Dec_32_Enbl13/29 -> Data_RAM (0x000 .. 0xFFF)/125(X04)
  Dec_32_Enbl13/20 -> Data_RAM (0x000 .. 0xFFF)/116(X12)
  Dec_32_Enbl16/32 -> Data_RAM (0x000 .. 0xFFF)/64(Y00)
  Dec_32_Enbl18/4 -> Data_RAM (0x000 .. 0xFFF)/68(X60)
  Dec_32_Enbl16/12 -> Data_RAM (0x000 .. 0xFFF)/44(Y20)
  Dec_32_Enbl17/2 -> Data_RAM (0x000 .. 0xFFF)/2(Y62)
  Align18/1 -> <0x1000..0x1FFF>/1(b15)
  Dec_32_Enbl13/23 -> Data_RAM (0x000 .. 0xFFF)/119(X09)
  Dec_32_Enbl17/32 -> Data_RAM (0x000 .. 0xFFF)/32(Y32)
  Dec_32_Enbl17/3 -> Data_RAM (0x000 .. 0xFFF)/3(Y61)
  Dec_32_Enbl13/16 -> Data_RAM (0x000 .. 0xFFF)/112(X16)
  Logical Operator78/1 -> Dec_32_Enbl13/1
  Dec_32_Enbl18/5 -> Data_RAM (0x000 .. 0xFFF)/69(X59)
  Dec_32_Enbl17/11 -> Data_RAM (0x000 .. 0xFFF)/11(Y53)
  Dec_32_Enbl17/21 -> Data_RAM (0x000 .. 0xFFF)/21(Y43)
  Dec_32_Enbl18/19 -> Data_RAM (0x000 .. 0xFFF)/83(X45)
  Dec_32_Enbl17/28 -> Data_RAM (0x000 .. 0xFFF)/28(Y36)
  Dec_32_Enbl17/6 -> Data_RAM (0x000 .. 0xFFF)/6(Y58)
  Dec_32_Enbl17/8 -> Data_RAM (0x000 .. 0xFFF)/8(Y56)
  Dec_32_Enbl16/6 -> Data_RAM (0x000 .. 0xFFF)/38(Y26)
  Dec_32_Enbl16/8 -> Data_RAM (0x000 .. 0xFFF)/40(Y24)
  Dec_32_Enbl17/13 -> Data_RAM (0x000 .. 0xFFF)/13(Y51)
  Dec_32_Enbl16/1 -> Data_RAM (0x000 .. 0xFFF)/33(Y31)
  Dec_32_Enbl16/20 -> Data_RAM (0x000 .. 0xFFF)/52(Y12)
  Dec_32_Enbl17/12 -> Data_RAM (0x000 .. 0xFFF)/12(Y52)
  Dec_32_Enbl17/10 -> Data_RAM (0x000 .. 0xFFF)/10(Y54)
  Logical Operator35/1 -> Dec_32_Enbl16/1
  Dec_32_Enbl18/7 -> Data_RAM (0x000 .. 0xFFF)/71(X57)
  Align18/6 -> Dec_32_Enbl18/2, <0x1000..0x1FFF>/6(b10), Dec_32_Enbl13/2
  Dec_32_Enbl18/16 -> Data_RAM (0x000 .. 0xFFF)/80(X48)
  Dec_32_Enbl13/24 -> Data_RAM (0x000 .. 0xFFF)/120(X08)
  Align18/16 -> <0x1000..0x1FFF>/16(b00), Align15/1
  Align15/2 -> Dec_32_Enbl17/5, Dec_32_Enbl16/5
  Align15/6 -> Dec_32_Enbl17/1, Logical Operator35/1
  Dec_32_Enbl18/3 -> Data_RAM (0x000 .. 0xFFF)/67(X61)
  Align15/4 -> Dec_32_Enbl17/3, Dec_32_Enbl16/3
  Dec_32_Enbl13/13 -> Data_RAM (0x000 .. 0xFFF)/109(X19)
  Dec_32_Enbl17/22 -> Data_RAM (0x000 .. 0xFFF)/22(Y42)
  Align18/7 -> Dec_32_Enbl18/3, <0x1000..0x1FFF>/7(b09), Dec_32_Enbl13/3
  Dec_32_Enbl18/15 -> Data_RAM (0x000 .. 0xFFF)/79(X49)
  Align15/1 -> Dec_32_Enbl17/6, Dec_32_Enbl16/6
  Dec_32_Enbl18/6 -> Data_RAM (0x000 .. 0xFFF)/70(X58)
  Select_Address/2 -> Bus Selector26/1
  Dec_32_Enbl18/1 -> Data_RAM (0x000 .. 0xFFF)/65(X63)
  Dec_32_Enbl17/1 -> Data_RAM (0x000 .. 0xFFF)/1(Y63)
  Dec_32_Enbl16/22 -> Data_RAM (0x000 .. 0xFFF)/54(Y10)
  Dec_32_Enbl16/21 -> Data_RAM (0x000 .. 0xFFF)/53(Y11)
  Dec_32_Enbl16/5 -> Data_RAM (0x000 .. 0xFFF)/37(Y27)
  Dec_32_Enbl13/21 -> Data_RAM (0x000 .. 0xFFF)/117(X11)
  Dec_32_Enbl16/24 -> Data_RAM (0x000 .. 0xFFF)/56(Y08)
  Dec_32_Enbl13/10 -> Data_RAM (0x000 .. 0xFFF)/106(X22)
  Dec_32_Enbl17/9 -> Data_RAM (0x000 .. 0xFFF)/9(Y55)
  Dec_32_Enbl13/25 -> Data_RAM (0x000 .. 0xFFF)/121(X07)
  Dec_32_Enbl13/2 -> Data_RAM (0x000 .. 0xFFF)/98(X30)
  Dec_32_Enbl16/29 -> Data_RAM (0x000 .. 0xFFF)/61(Y03)
  Dec_32_Enbl16/9 -> Data_RAM (0x000 .. 0xFFF)/41(Y23)
  Dec_32_Enbl18/27 -> Data_RAM (0x000 .. 0xFFF)/91(X37)
  Dec_32_Enbl16/10 -> Data_RAM (0x000 .. 0xFFF)/42(Y22)
  Dec_32_Enbl16/3 -> Data_RAM (0x000 .. 0xFFF)/35(Y29)
  Dec_32_Enbl16/11 -> Data_RAM (0x000 .. 0xFFF)/43(Y21)
  Align18/10 -> <0x1000..0x1FFF>/10(b06), Dec_32_Enbl13/6, Dec_32_Enbl18/6
  Dec_32_Enbl13/3 -> Data_RAM (0x000 .. 0xFFF)/99(X29)
  Dec_32_Enbl18/8 -> Data_RAM (0x000 .. 0xFFF)/72(X56)
  Dec_32_Enbl17/5 -> Data_RAM (0x000 .. 0xFFF)/5(Y59)
  Dec_32_Enbl17/26 -> Data_RAM (0x000 .. 0xFFF)/26(Y38)
  Dec_32_Enbl18/32 -> Data_RAM (0x000 .. 0xFFF)/96(X32)
  Dec_32_Enbl16/17 -> Data_RAM (0x000 .. 0xFFF)/49(Y15)
  Dec_32_Enbl13/6 -> Data_RAM (0x000 .. 0xFFF)/102(X26)
  Dec_32_Enbl16/28 -> Data_RAM (0x000 .. 0xFFF)/60(Y04)
  Dec_32_Enbl18/21 -> Data_RAM (0x000 .. 0xFFF)/85(X43)
  Dec_32_Enbl18/18 -> Data_RAM (0x000 .. 0xFFF)/82(X46)
  Dec_32_Enbl16/25 -> Data_RAM (0x000 .. 0xFFF)/57(Y07)
  Dec_32_Enbl17/7 -> Data_RAM (0x000 .. 0xFFF)/7(Y57)
  Dec_32_Enbl13/22 -> Data_RAM (0x000 .. 0xFFF)/118(X10)
  Dec_32_Enbl17/27 -> Data_RAM (0x000 .. 0xFFF)/27(Y37)
  Dec_32_Enbl13/8 -> Data_RAM (0x000 .. 0xFFF)/104(X24)
  Dec_32_Enbl18/12 -> Data_RAM (0x000 .. 0xFFF)/76(X52)
  Dec_32_Enbl16/26 -> Data_RAM (0x000 .. 0xFFF)/58(Y06)
  Align15/5 -> Dec_32_Enbl16/2, Dec_32_Enbl17/2
  Dec_32_Enbl13/18 -> Data_RAM (0x000 .. 0xFFF)/114(X14)
  Align18/12 -> <0x1000..0x1FFF>/12(b04), Align15/5
  Dec_32_Enbl16/14 -> Data_RAM (0x000 .. 0xFFF)/46(Y18)
  Dec_32_Enbl18/10 -> Data_RAM (0x000 .. 0xFFF)/74(X54)
  Dec_32_Enbl18/11 -> Data_RAM (0x000 .. 0xFFF)/75(X53)
  Dec_32_Enbl16/18 -> Data_RAM (0x000 .. 0xFFF)/50(Y14)
  Dec_32_Enbl16/19 -> Data_RAM (0x000 .. 0xFFF)/51(Y13)
  Dec_32_Enbl13/12 -> Data_RAM (0x000 .. 0xFFF)/108(X20)
  Dec_32_Enbl13/11 -> Data_RAM (0x000 .. 0xFFF)/107(X21)
  Dec_32_Enbl16/23 -> Data_RAM (0x000 .. 0xFFF)/55(Y09)
  Dec_32_Enbl13/17 -> Data_RAM (0x000 .. 0xFFF)/113(X15)
  Dec_32_Enbl13/5 -> Data_RAM (0x000 .. 0xFFF)/101(X27)
  Dec_32_Enbl18/22 -> Data_RAM (0x000 .. 0xFFF)/86(X42)
  Dec_32_Enbl13/9 -> Data_RAM (0x000 .. 0xFFF)/105(X23)
  Dec_32_Enbl13/4 -> Data_RAM (0x000 .. 0xFFF)/100(X28)
  Dec_32_Enbl16/16 -> Data_RAM (0x000 .. 0xFFF)/48(Y16)
  Dec_32_Enbl13/32 -> Data_RAM (0x000 .. 0xFFF)/128(X00)
  Dec_32_Enbl17/24 -> Data_RAM (0x000 .. 0xFFF)/24(Y40)
  Dec_32_Enbl18/20 -> Data_RAM (0x000 .. 0xFFF)/84(X44)
  Dec_32_Enbl16/30 -> Data_RAM (0x000 .. 0xFFF)/62(Y02)
  Dec_32_Enbl16/31 -> Data_RAM (0x000 .. 0xFFF)/63(Y01)
  Dec_32_Enbl17/20 -> Data_RAM (0x000 .. 0xFFF)/20(Y44)
  Dec_32_Enbl17/15 -> Data_RAM (0x000 .. 0xFFF)/15(Y49)
  Dec_32_Enbl18/30 -> Data_RAM (0x000 .. 0xFFF)/94(X34)
  Dec_32_Enbl13/31 -> Data_RAM (0x000 .. 0xFFF)/127(X01)
  Dec_32_Enbl18/31 -> Data_RAM (0x000 .. 0xFFF)/95(X33)
  Dec_32_Enbl16/7 -> Data_RAM (0x000 .. 0xFFF)/39(Y25)
  Dec_32_Enbl16/15 -> Data_RAM (0x000 .. 0xFFF)/47(Y17)
  Dec_32_Enbl18/13 -> Data_RAM (0x000 .. 0xFFF)/77(X51)
  Dec_32_Enbl17/31 -> Data_RAM (0x000 .. 0xFFF)/31(Y33)
  Dec_32_Enbl16/2 -> Data_RAM (0x000 .. 0xFFF)/34(Y30)
  Align18/2 -> <0x1000..0x1FFF>/2(b14)
  Dec_32_Enbl17/25 -> Data_RAM (0x000 .. 0xFFF)/25(Y39)
  "Select_Data  "/2 -> Bus Selector4/1
  Logical Operator52/1 -> Data_RAM (0x000 .. 0xFFF)/138(Write(1b))  "Write"
  CLK4/1 -> Data_RAM (0x000 .. 0xFFF)/129(CLK)  "CLK"
  Align45/12 -> Align20/12
  Align45/10 -> Align20/10
  Align45/9 -> Align20/9
  Align45/7 -> Align20/7
  Align45/8 -> Align20/8
  Align45/13 -> Align20/13
  Align45/16 -> Align20/16
  Align45/3 -> Align20/3
  Align45/1 -> Align20/1
  Align45/4 -> Align20/4
  Align45/11 -> Align20/11
  Align45/6 -> Align20/6
  Align45/5 -> Align20/5
  Align45/2 -> Align20/2
  Align45/15 -> Align20/15
  Align45/14 -> Align20/14
  Align33/1 -> Align23/1, <0xFFF6..0xFFF6>/1(b15)
  Align33/16 -> Align23/16, <0xFFF6..0xFFF6>/16(b00)
  Align33/8 -> Align23/8, <0xFFF6..0xFFF6>/8(b08)
  Align33/4 -> Align23/4, <0xFFF6..0xFFF6>/4(b12)
  Align33/13 -> Align23/13, <0xFFF6..0xFFF6>/13(b03)
  Align33/3 -> Align23/3, <0xFFF6..0xFFF6>/3(b13)
  Align33/7 -> Align23/7, <0xFFF6..0xFFF6>/7(b09)
  Align33/9 -> Align23/9, <0xFFF6..0xFFF6>/9(b07)
  Align33/12 -> Align23/12, <0xFFF6..0xFFF6>/12(b04)
  Align33/2 -> Align23/2, <0xFFF6..0xFFF6>/2(b14)
  Align33/14 -> Align23/14, <0xFFF6..0xFFF6>/14(b02)
  Align33/10 -> Align23/10, <0xFFF6..0xFFF6>/10(b06)
  Align33/5 -> Align23/5, <0xFFF6..0xFFF6>/5(b11)
  Align33/15 -> Align23/15, <0xFFF6..0xFFF6>/15(b01)
  Align33/11 -> Align23/11, <0xFFF6..0xFFF6>/11(b05)
  Align33/6 -> Align23/6, <0xFFF6..0xFFF6>/6(b10)
  Align23/1 -> Align22/1, Align42/1
  Align23/8 -> Align22/8, Align42/8
  Align23/4 -> Align22/4, Align42/4
  Align23/13 -> Align22/13, Align42/13
  Align23/3 -> Align22/3, Align42/3
  Align23/7 -> Align22/7, Align42/7
  Align23/9 -> Align22/9, Align42/9
  Align23/12 -> Align22/12, Align42/12
  Align23/2 -> Align22/2, Align42/2
  Align23/10 -> Align22/10, Align42/10
  Align23/5 -> Align22/5, Align42/5
  Align23/11 -> Align22/11, Align42/11
  Align23/6 -> Align22/6, Align42/6
  Alignment17/1 -> Alignment2/1
  Word_Enable30/7("b01 ") -> Merge2_8b_Simulated1/15
  Align25/1 -> Align26/1
  Align25/2 -> Align26/2
  Align25/3 -> Align26/3
  Align25/4 -> Align26/4
  Align25/5 -> Align26/5
  Align25/6 -> Align26/6
  Align25/7 -> Align26/7
  Align25/8 -> Align26/8
  Align53/1 -> Logical Operator54/1  "ReadFrom Ferrite Memory"
  Align53/2 -> Logical Operator14/1  "WriteTo Ferrite Memory"
  Align52/2 -> Align53/1
  Align52/1 -> Align53/2
  Align51/2 -> Align52/1
  Align51/3 -> Align52/2
  Align26/5 -> Data_RAM (0x000 .. 0xFFF)/134(Data_b03)
  Align26/3 -> Data_RAM (0x000 .. 0xFFF)/132(Data_b05)
  Align26/2 -> Data_RAM (0x000 .. 0xFFF)/131(Data_b06)
  Align26/4 -> Data_RAM (0x000 .. 0xFFF)/133(Data_b04)
  Align26/6 -> Data_RAM (0x000 .. 0xFFF)/135(Data_b02)
  Align26/7 -> Data_RAM (0x000 .. 0xFFF)/136(Data_b01)
  Align26/1 -> Data_RAM (0x000 .. 0xFFF)/130(Data_b07)
  Align26/8 -> Data_RAM (0x000 .. 0xFFF)/137(Data_b00)
  Video_RAM (0x000 .. 0x3FF)/9(b00) -> Word_Enable27/9(b00)
  Video_RAM (0x000 .. 0x3FF)/8(b01) -> Word_Enable27/8(b01)
  Video_RAM (0x000 .. 0x3FF)/7(b02) -> Word_Enable27/7(b02)
  Video_RAM (0x000 .. 0x3FF)/6(b03) -> Word_Enable27/6(b03)
  Video_RAM (0x000 .. 0x3FF)/5(b04) -> Word_Enable27/5(b04)
  Video_RAM (0x000 .. 0x3FF)/4(b05) -> Word_Enable27/4(b05)
  Video_RAM (0x000 .. 0x3FF)/3(b06) -> Word_Enable27/3(b06)
  Video_RAM (0x000 .. 0x3FF)/2(b07) -> Word_Enable27/2(b07)
  Data_RAM (0x000 .. 0xFFF)/4(b4) -> Word_Enable35/5(b04)
  Data_RAM (0x000 .. 0xFFF)/7(b7) -> Word_Enable35/8(b01)
  Data_RAM (0x000 .. 0xFFF)/5(b5) -> Word_Enable35/6(b03)
